simulink model "MIL4L3_SW6_V1_20220211"  (R2018b)
settings: Solver=FixedStepAuto  StartTime=0.0  StopTime=inf  FixedStep=0.001  RelTol=1e-3
PreLoadFcn:
  | A0_MILtest;
undefined symbols (not defined in the file or in its folder): Clb_ICADirect_LaneDisp_StateFive, Clb_ICADirect_LaneDisp_StateFour, Clb_ICADirect_LaneDisp_StateOne, Clb_ICADirect_LaneDisp_StateThree, Clb_ICADirect_LaneDisp_StateTwo, Clb_ICADirect_LaneDisp_StateZero, Clb_ICADirect_LaneDispSW, Clb_ICADirect_TrnLghtsCom_Switch, Clb_ICADirect_TrnLghtsCom_Value, Clb_ICADirect_TrnLghtsCrtl_Inhb, IMAP_Clb_ACU_Driver_Belt, IMAP_Clb_ACU_Driver_Belt_Over, IMAP_Clb_ACU_Passenger_Belt, IMAP_Clb_ACU_Passenger_Belt_Over, IMAP_Clb_ACU_RearLeft_Belt, IMAP_Clb_ACU_RearLeft_Belt_Over, IMAP_Clb_ACU_RearMiddle_Belt, IMAP_Clb_ACU_RearMiddle_Belt_Over, IMAP_Clb_ACU_RearRight_Belt, IMAP_Clb_ACU_RearRight_Belt_Over, IMAP_Clb_AEB_Switch, IMAP_Clb_AEB_Switch_Over, IMAP_Clb_ALC_TLC_Mode, IMAP_Clb_ALC_TLC_Mode_Over, IMAP_Clb_BCM_Battery_Voltage, IMAP_Clb_BCM_Battery_Voltage_Over, IMAP_Clb_BCM_BrakeLamp_State, IMAP_Clb_BCM_BrakeLamp_State_Over, IMAP_Clb_BCM_CHMSL_Status, IMAP_Clb_BCM_CHMSL_Status_Over, IMAP_Clb_BCM_Door_Lock_State, IMAP_Clb_BCM_Door_Lock_State_Over, IMAP_Clb_BCM_FrontWiper_State, IMAP_Clb_BCM_FrontWiper_State_Over, IMAP_Clb_BCM_FrontWiper_Switch, IMAP_Clb_BCM_FrontWiper_Switch_Over, IMAP_Clb_BCM_HazardLamp, IMAP_Clb_BCM_HazardLamp_Over, IMAP_Clb_BCM_HazardLamp_Switch, IMAP_Clb_BCM_HazardLamp_Switch_Over, IMAP_Clb_BCM_HighBeam_State, IMAP_Clb_BCM_HighBeam_State_Over, IMAP_Clb_BCM_Ignition_State, IMAP_Clb_BCM_Ignition_State_Over, IMAP_Clb_BCM_IHBC_Enabled, IMAP_Clb_BCM_IHBC_Enabled_Over, IMAP_Clb_BCM_Left_Light, IMAP_Clb_BCM_Left_Light_Over, IMAP_Clb_BCM_LeftTurn_Switch, IMAP_Clb_BCM_LeftTurn_Switch_Over, IMAP_Clb_BCM_LF_Door_State, IMAP_Clb_BCM_LF_Door_State_Over, IMAP_Clb_BCM_LowBeam_State, IMAP_Clb_BCM_LowBeam_State_Over, IMAP_Clb_BCM_LR_Door_State, IMAP_Clb_BCM_LR_Door_State_Over, IMAP_Clb_BCM_RF_Door_State, IMAP_Clb_BCM_RF_Door_State_Over, IMAP_Clb_BCM_Right_Light, IMAP_Clb_BCM_Right_Light_Over ... (+547)
libraries: CarMaker4SL x2153, simulink x292, dspstat3 x3, canmsglib x2, simulink_extras x1
(part 31 of 52)

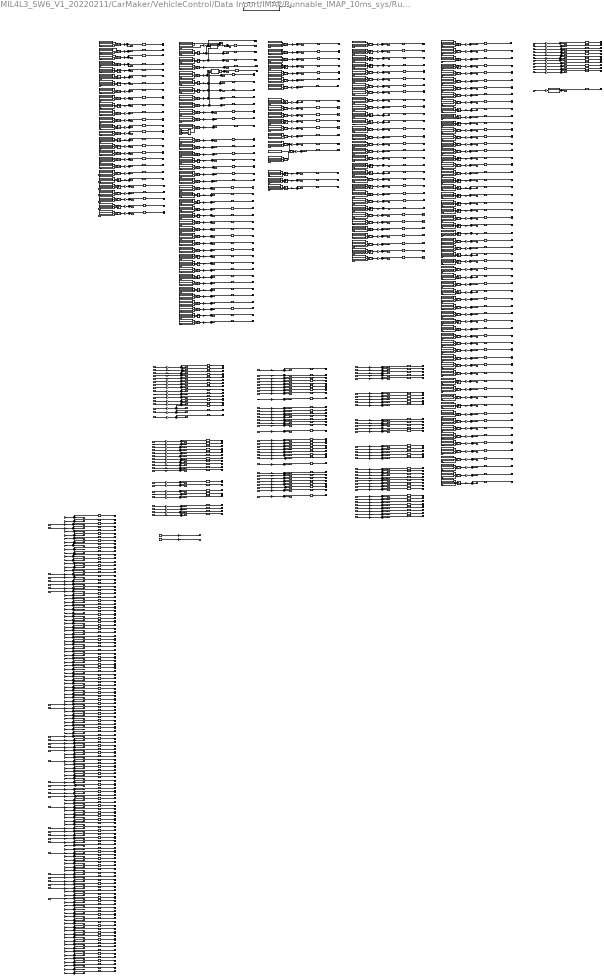
== system MIL4L3_SW6_V1_20220211/CarMaker/VehicleControl/Data Inport/IMAP/Runnable_IMAP_10ms_sys/Runnable_IMAP_10ms_sys/IMAP_Module ==
  note: SDFA_Lane_Back
  note: ORI
  note: SDFA_Sensor_Status
  note: MP5
  note: EMS
  note: SDFA_Lane
  note: SDFA_Obj
  note: BCM
  note: EPS
  note: DMS
  note: ESC
  note: 三个信号TBOX/语音/物理按键取或关系转译，转译结果0：开关关闭，1：开关开启
  SWINve_y_ABS_in_regulation : Inport
  SWINve_g_ACCEL_LONGI_CALIB : Inport  Port=2
  SWINve_y_ASR_ESP_disconnected : Inport  Port=3
  SWINve_y_ASR_in_regulation : Inport  Port=4
  SWINve_y_BCM_BrakeLampStatus : Inport  Port=5
  SWINve_y_BCM_CHMSLStatus : Inport  Port=6
  SWINve_y_BCM_State_Front_Wiper : Inport  Port=7
  SWINve_y_BCM_Status_Indicator : Inport  Port=8
  SWINve_y_Brake_secondary_contact : Inport  Port=9
  SWINve_y_Braking_effort : Inport  Port=10
  SWINve_y_Dynamic_slope : Inport  Port=11
  SWINve_y_Dynamic_slope_accuracy : Inport  Port=12
  SWINve_y_EMS_ACC_Effecitive_EMS : Inport  Port=13
  SWINve_y_EMS_ACCcontrol_Available : Inport  Port=14
  SWINve_g_EMS_Acceleration_pedal_position : Inport  Port=15
  SWINve_g_EMS_Actual_torque : Inport  Port=16
  SWINve_g_EMS_Actual_whlTrq : Inport  Port=17
  SWINve_g_EMS_Driver_request : Inport  Port=18
  SWINve_g_EMS_Driver_wheel_torque : Inport  Port=19
  SWINve_g_EMS_Engine_RPM : Inport  Port=20
  SWINve_y_EMS_Engine_state : Inport  Port=21
  SWINve_y_EMS_GearBox_ACC_Ctl_Available : Inport  Port=22
  SWINve_g_EMS_WhlTrq_max : Inport  Port=23
  SWINve_g_EMS_WhlTrq_max_offset : Inport  Port=24
  SWINve_g_EMS_WhlTrq_min : Inport  Port=25
  SWINve_g_EMS_WhlTrq_min_offset : Inport  Port=26
  SWINve_y_ESP_in_regulation : Inport  Port=27
  SWINve_y_Front_Left_pulse_malfunction : Inport  Port=28
  SWINve_y_Front_right_pulse_malfunction : Inport  Port=29
  SWINve_y_GW_BCM_SEV_main_state : Inport  Port=30
  SWINve_y_GW_EMS_ACC_Ihibited_By_Engine : Inport  Port=31
  SWINve_y_GW_EMS_EMS_Status_ACC : Inport  Port=32
  SWINve_g_GW_EMS_Pot_WhlTrq_Max : Inport  Port=33
  SWINve_g_GW_EMS_Pot_WhlTrq_Min : Inport  Port=34
  SWINve_y_GW_Mp5_ISA_Switch : Inport  Port=35
  SWINve_y_GW_Mp5_TSR_Switch : Inport  Port=36
  SWINve_y_GW_SCC_LeftSteeringWheelSwitch : Inport  Port=37
  SWINve_y_GW_SCC_RightSteeringWheelSwitch : Inport  Port=38
  SWINve_y_BCM_HazardSwitchrSt : Inport  Port=39  OutDataTypeStr=uint8  PortDimensions=1
  SWINve_y_MP5_HazardLampCtrlReq : Inport  Port=40  OutDataTypeStr=uint8  PortDimensions=1
  SWINve_y_T_box_RemoteHazardReq : Inport  Port=41  OutDataTypeStr=uint8  PortDimensions=1
  SWINve_y_High_beam_state : Inport  Port=42
  SWINve_y_IC_Fcw_Activation_Config : Inport  Port=43
  SWINve_y_IC_FCW_Sensitivity : Inport  Port=44
  SWINve_y_IC_passengerBeltSwitchSig : Inport  Port=45
  SWINve_y_IC_seat_bealt_driver_state : Inport  Port=46
  SWINve_y_Internal_SWS_status : Inport  Port=47
  SWINve_g_Lateral_acceleration : Inport  Port=48
  SWINve_y_LC_Mode : Inport  Port=49
  SWINve_y_LKA_main_switch : Inport  Port=50
  SWINve_y_Message_from_ESC_informing : Inport  Port=51
  SWINve_y_MP5_AEB_Activation_Config : Inport  Port=52
  SWINve_y_MSR_in_regulation : Inport  Port=53
  SWINve_g_No_filtered_front_left_speed : Inport  Port=54
  SWINve_g_No_filtered_front_right_speed : Inport  Port=55
  SWINve_g_No_filtered_rear_left_speed : Inport  Port=56
  SWINve_g_No_filtered_rear_rignt_speed : Inport  Port=57
  SWINve_g_number_of_kilometer : Inport  Port=58
  SWINve_y_Park_brake_function_status : Inport  Port=59
  SWINve_g_Pulse_counter_front_left_wheel : Inport  Port=60
  SWINve_g_Pulse_counter_front_right_wheel : Inport  Port=61
  SWINve_g_Pulse_counter_rearleft_wheel : Inport  Port=62
  SWINve_g_Pulse_counter_rearright_wheel : Inport  Port=63
  SWINve_y_Rear_Left_pulse_malfunction : Inport  Port=64
  SWINve_y_Rear_Right_pulse_malfunction : Inport  Port=65
  SWINve_y_Request_to_light_fault_lamp : Inport  Port=66
  SWINve_y_State_indicating_steer_or_not : Inport  Port=67
  SWINve_y_State_of_EPS_for_LKA_function : Inport  Port=68
  SWINve_g_Static_slope : Inport  Port=69
  SWINve_g_Steering_wheel_angle : Inport  Port=70
  SWINve_g_Steering_wheel_rotation_speed : Inport  Port=71
  SWINve_g_Steering_wheel_torque : Inport  Port=72
  SWINve_y_SWS_calibration : Inport  Port=73
  SWINve_y_SWS_trim : Inport  Port=74
  SWINve_y_TCU_AGB_Target_position : Inport  Port=75
  SWINve_y_TCU_ATFailure : Inport  Port=76
  SWINve_y_TCU_DCTClutchStatus : Inport  Port=77
  SWINve_y_TCU_Gear_lever_position : Inport  Port=78
  SWINve_y_TCU_GearEngagement : Inport  Port=79
  SWINve_y_TCU_PROGRAMME_ACC : Inport  Port=80
  SWINve_g_TMC_pressure : Inport  Port=81
  SWINve_y_Torque_limitation_if_DAE_limit : Inport  Port=82
  SWINve_y_Vehicle_detected_as_stationary : Inport  Port=83
  SWINve_y_Vehicle_driving_direction : Inport  Port=84
  SWINve_y_Vehicle_Hold_Status : Inport  Port=85
  SWINve_g_Vehicle_speed_of_wheelsensor : Inport  Port=86
  SWINve_y_Vehiclespd_unavailability_flag : Inport  Port=87
  SWINve_g_Yaw_speed : Inport  Port=88
  SWINve_g_YawRate_Raw : Inport  Port=89
  System_Clock : Inport  Port=90
  SDFAve_d_sensor_status : Inport  Port=91
  SDFAve_d_sen_sta_LF_radar : Inport  Port=92
  SDFAve_d_sen_sta_RF_radar : Inport  Port=93
  SDFAve_d_sen_sta_LB_radar : Inport  Port=94
  SDFAve_d_sen_sta_RB_radar : Inport  Port=95
  SDFAve_d_fusion_status : Inport  Port=96
  SDFAve_d_fusion_time_stamp : Inport  Port=97
  SDFAve_d_obj_Num : Inport  Port=98
  SDFAva_y_obj_id : Inport  Port=99
  SDFAva_g_obj_pos_x : Inport  Port=100
  SDFAva_g_obj_pos_y : Inport  Port=101
  SDFAva_g_obj_vel_x : Inport  Port=102
  SDFAva_g_obj_vel_y : Inport  Port=103
  SDFAva_g_obj_acc_x : Inport  Port=104
  SDFAva_g_obj_acc_y : Inport  Port=105
  SDFAva_g_obj_pos_var_x : Inport  Port=106
  SDFAva_g_obj_pos_var_y : Inport  Port=107
  SDFAva_g_obj_pos_var_xy : Inport  Port=108
  SDFAva_g_obj_width : Inport  Port=109
  SDFAva_g_obj_length : Inport  Port=110
  SDFAva_y_obj_class : Inport  Port=111
  SDFAva_y_obj_lane : Inport  Port=112
  SDFAva_d_obj_status : Inport  Port=113
  SDFAva_d_obj_age : Inport  Port=114
  SDFAva_y_obj_TurnLight : Inport  Port=115
  SDFAva_y_obj_BrakeLight : Inport  Port=116
  SDFAva_y_obj_MotionStatus : Inport  Port=117
  SDFAve_y_ROAD_TYPE : Inport  Port=118
  SDFAve_g_L0_C0_COEF : Inport  Port=119
  SDFAve_g_L0_C1_COEF : Inport  Port=120
  SDFAve_g_L0_C2_COEF : Inport  Port=121
  SDFAve_g_L0_C3_COEF : Inport  Port=122
  SDFAve_g_L0_VIEW_RANGE : Inport  Port=123
  SDFAve_y_L0_DETECT_QUALITY : Inport  Port=124
  SDFAve_d_L0_LINE_TYPE : Inport  Port=125
  SDFAve_g_L0_MARK_WIDTH : Inport  Port=126
  SDFAve_g_R0_C0_COEF : Inport  Port=127
  SDFAve_g_R0_C1_COEF : Inport  Port=128
  SDFAve_g_R0_C2_COEF : Inport  Port=129
  SDFAve_g_R0_C3_COEF : Inport  Port=130
  SDFAve_g_R0_VIEW_RANGE : Inport  Port=131
  SDFAve_y_R0_DETECT_QUALITY : Inport  Port=132
  SDFAve_d_R0_LINE_TYPE : Inport  Port=133
  SDFAve_g_R0_MARK_WIDTH : Inport  Port=134
  SDFAve_g_L1_C0_COEF : Inport  Port=135
  SDFAve_g_L1_C1_COEF : Inport  Port=136
  SDFAve_g_L1_C2_COEF : Inport  Port=137
  SDFAve_g_L1_C3_COEF : Inport  Port=138
  SDFAve_g_L1_VIEW_RANGE : Inport  Port=139
  SDFAve_y_L1_DETECT_QUALITY : Inport  Port=140
  SDFAve_d_L1_LINE_TYPE : Inport  Port=141
  SDFAve_g_L1_MARK_WIDTH : Inport  Port=142
  SDFAve_g_R1_C0_COEF : Inport  Port=143
  SDFAve_g_R1_C1_COEF : Inport  Port=144
  SDFAve_g_R1_C2_COEF : Inport  Port=145
  SDFAve_g_R1_C3_COEF : Inport  Port=146
  SDFAve_g_R1_VIEW_RANGE : Inport  Port=147
  SDFAve_y_R1_DETECT_QUALITY : Inport  Port=148
  SDFAve_d_R1_LINE_TYPE : Inport  Port=149
  SDFAve_g_R1_MARK_WIDTH : Inport  Port=150
  SDFAve_g_L0_C0_BACK_COEF : Inport  Port=151
  SDFAve_g_L0_C1_BACK_COEF : Inport  Port=152
  SDFAve_g_L0_C2_BACK_COEF : Inport  Port=153
  SDFAve_g_L0_C3_BACK_COEF : Inport  Port=154
  SDFAve_g_L0_BACK_RANGE : Inport  Port=155
  SDFAve_g_R0_C0_BACK_COEF : Inport  Port=156
  SDFAve_g_R0_C1_BACK_COEF : Inport  Port=157
  SDFAve_g_R0_C2_BACK_COEF : Inport  Port=158
  SDFAve_g_R0_C3_BACK_COEF : Inport  Port=159
  SDFAve_g_R0_BACK_RANGE : Inport  Port=160
  SDFAve_g_L1_C0_BACK_COEF : Inport  Port=161
  SDFAve_g_L1_C1_BACK_COEF : Inport  Port=162
  SDFAve_g_L1_C2_BACK_COEF : Inport  Port=163
  SDFAve_g_L1_C3_BACK_COEF : Inport  Port=164
  SDFAve_g_L1_BACK_RANGE : Inport  Port=165
  SDFAve_g_R1_C0_BACK_COEF : Inport  Port=166
  SDFAve_g_R1_C1_BACK_COEF : Inport  Port=167
  SDFAve_g_R1_C2_BACK_COEF : Inport  Port=168
  SDFAve_g_R1_C3_BACK_COEF : Inport  Port=169
  SDFAve_g_R1_BACK_RANGE : Inport  Port=170
  SDFAve_g_Lrg_C0_BACK_COEF : Inport  Port=171
  SDFAve_g_Lrg_C1_BACK_COEF : Inport  Port=172
  SDFAve_g_Lrg_C2_BACK_COEF : Inport  Port=173
  SDFAve_g_Lrg_C3_BACK_COEF : Inport  Port=174
  SDFAve_g_Lrg_VIEW_RANGE_start : Inport  Port=175
  SDFAve_g_Lrg_VIEW_RANGE_end : Inport  Port=176
  SDFAve_y_Lrg_DETECT_QUALITY : Inport  Port=177
  SDFAve_y_Lrg_LINE_TYPE : Inport  Port=178
  SDFAve_g_Rrg_C0_BACK_COEF : Inport  Port=179
  SDFAve_g_Rrg_C1_BACK_COEF : Inport  Port=180
  SDFAve_g_Rrg_C2_BACK_COEF : Inport  Port=181
  SDFAve_g_Rrg_C3_BACK_COEF : Inport  Port=182
  SDFAve_g_Rrg_VIEW_RANGE_start : Inport  Port=183
  SDFAve_g_Rrg_VIEW_RANGE_end : Inport  Port=184
  SDFAve_y_Rrg_DETECT_QUALITY : Inport  Port=185
  SDFAve_y_Rrg_LINE_TYPE : Inport  Port=186
  SDFAve_y_ISAValue : Inport  Port=187
  SDFAve_y_ISAPopupMessage : Inport  Port=188
  SDFAve_y_ISASignType : Inport  Port=189
  SDFAve_y_ISAStatus : Inport  Port=190
  SDFAve_y_TSR_Sign_Type : Inport  Port=191
  SDFAve_g_CameraSignalFault : Inport  Port=192
  SDFAve_y_Radar_State : Inport  Port=193
  SDFAve_y_OperatingStatus : Inport  Port=194
  SDFAve_y_Radar_FaultBitSetting_Signal : Inport  Port=195
  SWINve_y_ESC_FLWDirection : Inport  Port=196  OutDataTypeStr=uint8  PortDimensions=1
  SWINve_y_ESC_FRWDirection : Inport  Port=197  OutDataTypeStr=uint8  PortDimensions=1
  SWINve_y_ESC_TCSErrorStatus : Inport  Port=198  OutDataTypeStr=uint8  PortDimensions=1
  SWINve_y_ESC-RLWDirection : Inport  Port=199  OutDataTypeStr=uint8  PortDimensions=1
  SWINve_y_ESC_RRWDirection : Inport  Port=200  OutDataTypeStr=uint8  PortDimensions=1
  SWINve_y_ESC_EPBErrorStatus : Inport  Port=201  OutDataTypeStr=uint8  PortDimensions=1
  SWINve_y_EPS_SteeringAngle_Flag : Inport  Port=202  OutDataTypeStr=uint8  PortDimensions=1
  SWINve_g_EPS_SteeringAngle : Inport  Port=203  OutDataTypeStr=single  PortDimensions=1
  SWINve_y_EPS_DriverOverride : Inport  Port=204  OutDataTypeStr=uint8  PortDimensions=1
  SWINve_y_EPS_DriverInitializedESA : Inport  Port=205  OutDataTypeStr=uint8
  SWINve_y_EPS_ESAState : Inport  Port=206  OutDataTypeStr=uint8
  SWINve_y_ACU_RearLeftBeltSwitchSig : Inport  Port=207  OutDataTypeStr=uint8
  SWINve_y_ACU_RearMiddleBeltSwitchSig : Inport  Port=208  OutDataTypeStr=uint8
  SWINve_y_ACU_RearRightBeltSwitchSig : Inport  Port=209  OutDataTypeStr=uint8
  SWINve_y_EMS_PowertrainControlSt : Inport  Port=210  OutDataTypeStr=uint8
  SWINve_y_TCU_TCUAvailable : Inport  Port=211  OutDataTypeStr=uint8
  SWINve_y_BCM_LeftTurnSwitchSt : Inport  Port=212  OutDataTypeStr=uint8
  SWINve_y_BCM_RightTurnSwitchSt : Inport  Port=213  OutDataTypeStr=uint8
  SWINve_y_BCM_FrontWiperSwitchSt : Inport  Port=214  OutDataTypeStr=uint8
  SWINve_y_BCM_IHBC_Function_Enabled : Inport  Port=215  OutDataTypeStr=uint8
  SWINve_y_MP5_WorkSt : Inport  Port=216  OutDataTypeStr=uint8
  SWINve_y_MP5_APAModeSelect : Inport  Port=217  OutDataTypeStr=uint8
  SWINve_y_MP5_LanguageSet : Inport  Port=218  OutDataTypeStr=uint8
  SWINve_y_MP5_UPASwitch : Inport  Port=219  OutDataTypeStr=uint8
  SWINve_y_MP5_FLKActivation : Inport  Port=220  OutDataTypeStr=uint8
  SWINve_y_MP5_AutoPilotSwitch : Inport  Port=221  OutDataTypeStr=uint8
  SWINve_y_MP5_DMS_MessageType : Inport  Port=222  OutDataTypeStr=uint8
  SWINve_y_MP5_DMS_SystemEnable : Inport  Port=223  OutDataTypeStr=uint8
  SWINve_y_MP5_DMS_DeleteUserNum : Inport  Port=224  OutDataTypeStr=uint8
  SWINve_y_MP5_DMS_Sensity : Inport  Port=225  OutDataTypeStr=uint8
  SWINve_y_MP5_DMS_EyeFatigueMonitor : Inport  Port=226  OutDataTypeStr=uint8
  SWINve_y_MP5_DMS_LongtimeDriveMonitor : Inport  Port=227  OutDataTypeStr=uint8
  SWINve_y_MP5_DMS_SideViewMonitor : Inport  Port=228  OutDataTypeStr=uint8
  SWINve_y_MP5_DMS_UsingPhoneMonitor : Inport  Port=229  OutDataTypeStr=uint8
  SWINve_y_MP5_DMS_SmokingMonitor : Inport  Port=230  OutDataTypeStr=uint8
  SWINve_y_MP5_DMS_DrinkWaterMonitor : Inport  Port=231  OutDataTypeStr=uint8
  SWINve_y_MP5_DMS_UserAccount : Inport  Port=232  OutDataTypeStr=uint8
  SWINve_y_Mp5_ISAMode : Inport  Port=233  OutDataTypeStr=uint8  PortDimensions=1
  SWINve_y_Mp5_LDWWarningMode : Inport  Port=234  OutDataTypeStr=uint8  PortDimensions=1
  SWINve_y_MP5_ADASSpeedLimit : Inport  Port=235  OutDataTypeStr=uint8  PortDimensions=1
  SWINve_y_MP5_TLCModeSelection : Inport  Port=236  OutDataTypeStr=uint8  PortDimensions=1
  SWINve_y_MP5_ESASwitch : Inport  Port=237  OutDataTypeStr=uint8  PortDimensions=1
  SWINve_y_Mp5_ELKSwitch : Inport  Port=238  OutDataTypeStr=uint8
  SWINve_y_PEPS_RKECommand : Inport  Port=239  OutDataTypeStr=uint8  PortDimensions=1
  SWINve_y_MP5_BSD_LCW_Activation : Inport  Port=240  OutDataTypeStr=uint8  PortDimensions=1
  SWINve_y_MP5_FCTAActivation : Inport  Port=241  OutDataTypeStr=uint8  PortDimensions=1
  SWINve_y_MP5_RCTAActivation : Inport  Port=242  OutDataTypeStr=uint8  PortDimensions=1
  SWINve_y_MP5_DOWActivation : Inport  Port=243  OutDataTypeStr=uint8
  SWINve_y_MP5_JA_Modes : Inport  Port=244  OutDataTypeStr=uint8
  SWINve_y_MP5_JA_Alert_Switch : Inport  Port=245  OutDataTypeStr=uint8
  SWINve_y_ESC_BLRequest : Inport  Port=246  OutDataTypeStr=uint8  PortDimensions=1
  SWINve_y_PEPS_DoorLockReq : Inport  Port=247  OutDataTypeStr=uint8  PortDimensions=1
  SWINve_y_BCM_DoorLockSt : Inport  Port=248  OutDataTypeStr=uint8  PortDimensions=1
  SWINve_y_BCM_LowBeamStatus : Inport  Port=249  OutDataTypeStr=uint8  PortDimensions=1
  SWINve_g_BCM_BattVolt : Inport  Port=250  OutDataTypeStr=single  PortDimensions=1
  SWINve_d_TBOX_LocalTimeYear : Inport  Port=251  OutDataTypeStr=uint16  PortDimensions=1
  SWINve_y_TBOX_LocalTimeMonth : Inport  Port=252  OutDataTypeStr=uint8  PortDimensions=1
  SWINve_y_TBOX_LocalTimeDate : Inport  Port=253  OutDataTypeStr=uint8  PortDimensions=1
  SWINve_y_TBOX_LocalTimeHour : Inport  Port=254  OutDataTypeStr=uint8  PortDimensions=1
  SWINve_y_TBOX_LocalTimeMinute : Inport  Port=255  OutDataTypeStr=uint8
  SWINve_y_TBOX_LocalTimeSecond : Inport  Port=256  OutDataTypeStr=uint8
  SWINve_y_TBOX_LocalTimeValid : Inport  Port=257  OutDataTypeStr=uint8
  SWINve_g_AC_AmbTemp : Inport  Port=258  OutDataTypeStr=single
  SWINve_y_EPS_SteeringTorqueSensorSt : Inport  Port=259  OutDataTypeStr=uint8  PortDimensions=1
  SWINve_g_EPS_LKACurrentOverlay : Inport  Port=260  OutDataTypeStr=single  PortDimensions=1
  SWINve_y_EPS_WarningLampSt : Inport  Port=261  OutDataTypeStr=uint8  PortDimensions=1
  SWINve_g_EPS_ElectPowerConsumption : Inport  Port=262  OutDataTypeStr=single  PortDimensions=1
  SWINve_g_EMS_EngActualIndTorque : Inport  Port=263  OutDataTypeStr=single  PortDimensions=1
  SWINve_y_EMS_AccPedalFaultBit : Inport  Port=264  OutDataTypeStr=uint8  PortDimensions=1
  SWINve_y_TCU_PRNDLStatus : Inport  Port=265  OutDataTypeStr=uint8  PortDimensions=1
  SWINve_y_TCU_ShiftLeverPosValidFlag : Inport  Port=266  OutDataTypeStr=uint8  PortDimensions=1
  SWINve_y_ESC_LateralAccelarationValidity : Inport  Port=267  OutDataTypeStr=uint8  PortDimensions=1
  SWINve_y_ESC_YawrateValidity : Inport  Port=268  OutDataTypeStr=uint8
  SWINve_y_ESC_LongitudinalAccelerationValidity : Inport  Port=269  OutDataTypeStr=uint8
  SWINve_y_ESC_ABSValidity : Inport  Port=270  OutDataTypeStr=uint8
  SWINve_y_ESC_ABSAlarmSig : Inport  Port=271  OutDataTypeStr=uint8
  SWINve_y_ESC_FLWHeelSpdFaultSignal : Inport  Port=272  OutDataTypeStr=uint8
  SWINve_y_ESC_FRWHeelSpdFaultSignal : Inport  Port=273  OutDataTypeStr=uint8
  SWINve_y_ESC_RLWHeelSpdFaultSignal : Inport  Port=274  OutDataTypeStr=uint8
  SWINve_y_ESC_RRWHeelSpdFaultSignal : Inport  Port=275  OutDataTypeStr=uint8
  SWINve_y_ESC_AEBAvailable : Inport  Port=276  OutDataTypeStr=uint8
  SWINve_y_ESC_AEBActive : Inport  Port=277  OutDataTypeStr=uint8
  SWINve_y_ESC_ACCAvailable : Inport  Port=278  OutDataTypeStr=uint8
  SWINve_y_ESC_ACCActive : Inport  Port=279  OutDataTypeStr=uint8
  SWINve_y_ESC_EPBDisplayMessageReq : Inport  Port=280  OutDataTypeStr=uint8
  SWINve_y_ESC_EPBWarningIndicationReq : Inport  Port=281  OutDataTypeStr=uint8
  SWINve_y_ESC_EPBSwitchStatics : Inport  Port=282  OutDataTypeStr=uint8
  SWINve_y_ESC_EPBSwitchStaticsValidity : Inport  Port=283  OutDataTypeStr=uint8
  SWINve_y_ESC_EBDAlarmSig : Inport  Port=284  OutDataTypeStr=uint8
  SWINve_y_ESC_AVHStatus : Inport  Port=285  OutDataTypeStr=uint8
  SWINve_y_BCM_LeftlightSt : Inport  Port=286  OutDataTypeStr=uint8  PortDimensions=1
  SWINve_y_BCM_RightlightSt : Inport  Port=287  OutDataTypeStr=uint8  PortDimensions=1
  SWINve_y_BCM_TrunkSt : Inport  Port=288  OutDataTypeStr=uint8  PortDimensions=1
  SWINve_y_BCM_LFDoorSwitchSt : Inport  Port=289  OutDataTypeStr=uint8  PortDimensions=1
  SWINve_y_BCM_RFDoorSwitchSt : Inport  Port=290  OutDataTypeStr=uint8  PortDimensions=1
  SWINve_y_BCM_RRDoorSwitchSt : Inport  Port=291  OutDataTypeStr=uint8  PortDimensions=1
  SWINve_y_BCM_LRDoorSwitchSt : Inport  Port=292  OutDataTypeStr=uint8  PortDimensions=1
  SWINve_g_ESC_BrakeWheelCylinderPressure : Inport  Port=293  OutDataTypeStr=single  PortDimensions=1
  FAPAve_Cnt_AdvancedParkingAssist : Inport  Port=294
  SDFAve_d_ORI_CIPV_ID : Inport  Port=295
  SDFAve_d_ORI_Obj_Num : Inport  Port=296
  SDFAva_g_ORI_Obj_AbsAx : Inport  Port=297  PortDimensions=20
  SDFAva_g_ORI_Obj_AbsAy : Inport  Port=298  PortDimensions=20
  SDFAva_g_ORI_Obj_RelVel : Inport  Port=299  PortDimensions=20
  SDFAva_g_ORI_Obj_RelVely : Inport  Port=300  PortDimensions=20
  SDFAva_g_ORI_Obj_LongDis : Inport  Port=301  PortDimensions=20
  SDFAva_g_ORI_Obj_LateralDis : Inport  Port=302  PortDimensions=20
  SDFAva_d_ORI_Obj_Class : Inport  Port=303  PortDimensions=20
  SDFAva_d_ORI_Obj_ID : Inport  Port=304  PortDimensions=20
  SDFAve_g_ORI_L0_C3 : Inport  Port=305
  SDFAve_g_ORI_L0_C2 : Inport  Port=306
  SDFAve_g_ORI_L0_C1 : Inport  Port=307
  SDFAve_g_ORI_L0_C0 : Inport  Port=308
  SDFAve_d_ORI_L0_Type : Inport  Port=309
  SDFAve_g_ORI_L0_VR : Inport  Port=310
  SDFAve_g_ORI_L1_C3 : Inport  Port=311
  SDFAve_g_ORI_L1_C2 : Inport  Port=312
  SDFAve_g_ORI_L1_C1 : Inport  Port=313
  SDFAve_g_ORI_L1_C0 : Inport  Port=314
  SDFAve_d_ORI_L1_Type : Inport  Port=315
  SDFAve_g_ORI_L1_VR : Inport  Port=316
  SDFAve_g_ORI_R0_C3 : Inport  Port=317
  SDFAve_g_ORI_R0_C2 : Inport  Port=318
  SDFAve_g_ORI_R0_C1 : Inport  Port=319
  SDFAve_g_ORI_R0_C0 : Inport  Port=320
  SDFAve_d_ORI_R0_LT : Inport  Port=321
  SDFAve_g_ORI_R0_VR : Inport  Port=322
  SDFAve_g_ORI_R1_C3 : Inport  Port=323
  SDFAve_g_ORI_R1_C2 : Inport  Port=324
  SDFAve_g_ORI_R1_C1 : Inport  Port=325
  SDFAve_g_ORI_R1_C0 : Inport  Port=326
  SDFAve_d_ORI_R1_LT : Inport  Port=327
  SDFAve_g_ORI_R1_VR : Inport  Port=328
  AND : Logic  Operator=OR  Inputs=3  AllPortsSameDT=off  OutDataTypeStr=boolean
  Constant : Constant  Value=IMAP_Clb_LKA_Main_Switch  OutDataTypeStr=uint16
  Constant1 : Constant  Value=IMAP_Clb_LKA_Main_Switch_Over  OutDataTypeStr=boolean
  Constant10 : Constant  Value=IMAP_Clb_ISA_Switch  OutDataTypeStr=uint16
  Constant100 : Constant  Value=IMAP_Clb_TBOX_LocalTimeM  OutDataTypeStr=uint16
  Constant101 : Constant  Value=IMAP_Clb_TBOX_LocalTimeM_Over  OutDataTypeStr=boolean
  Constant102 : Constant  Value=IMAP_Clb_TBOX_LocalTimeD  OutDataTypeStr=uint16
  Constant103 : Constant  Value=IMAP_Clb_TBOX_LocalTimeD_Over  OutDataTypeStr=boolean
  Constant104 : Constant  Value=IMAP_Clb_TBOX_LocalTimeH  OutDataTypeStr=uint16
  Constant105 : Constant  Value=IMAP_Clb_TBOX_LocalTimeH_Over  OutDataTypeStr=boolean
  Constant106 : Constant  Value=IMAP_Clb_TBOX_LocalTimeMin  OutDataTypeStr=uint16
  Constant107 : Constant  Value=IMAP_Clb_TBOX_LocalTimeMin_Over  OutDataTypeStr=boolean
  Constant108 : Constant  Value=IMAP_Clb_TBOX_LocalTimeS  OutDataTypeStr=uint16
  Constant109 : Constant  Value=IMAP_Clb_TBOX_LocalTimeS_Over  OutDataTypeStr=boolean
  Constant11 : Constant  Value=IMAP_Clb_ISA_Switch_Over  OutDataTypeStr=boolean
  Constant110 : Constant  Value=IMAP_Clb_TBOX_LocalTime_Valid  OutDataTypeStr=uint16
  Constant111 : Constant  Value=IMAP_Clb_TBOX_LocalTime_Valid_Over  OutDataTypeStr=boolean
  Constant112 : Constant  Value=IMAP_Clb_Time_System_Clock  OutDataTypeStr=uint16
  Constant113 : Constant  Value=IMAP_Clb_Time_System_Clock_Over  OutDataTypeStr=boolean
  Constant114 : Constant  Value=IMAP_Clb_GW_IC_Odometer  OutDataTypeStr=uint32
  Constant115 : Constant  Value=IMAP_Clb_GW_IC_Odometer_Over  OutDataTypeStr=boolean
  Constant116 : Constant  Value=IMAP_Clb_Outside_Temp  OutDataTypeStr=uint16
  Constant117 : Constant  Value=IMAP_Clb_Outside_Temp_Over  OutDataTypeStr=boolean
  Constant118 : Constant  Value=IMAP_Clb_ACU_RearLeft_Belt  OutDataTypeStr=uint16
  Constant119 : Constant  Value=IMAP_Clb_ACU_RearLeft_Belt_Over  OutDataTypeStr=boolean
  Constant12 : Constant  Value=IMAP_Clb_TSR_Switch  OutDataTypeStr=uint16
  Constant120 : Constant  Value=IMAP_Clb_ACU_RearMiddle_Belt  OutDataTypeStr=uint16
  Constant121 : Constant  Value=IMAP_Clb_ACU_RearMiddle_Belt_Over  OutDataTypeStr=boolean
  Constant122 : Constant  Value=IMAP_Clb_ACU_RearRight_Belt  OutDataTypeStr=uint16
  Constant123 : Constant  Value=IMAP_Clb_ACU_RearRight_Belt_Over  OutDataTypeStr=boolean
  Constant124 : Constant  Value=IMAP_Clb_BCM_LeftTurn_Switch  OutDataTypeStr=uint16
  Constant125 : Constant  Value=IMAP_Clb_BCM_LeftTurn_Switch_Over  OutDataTypeStr=boolean
  Constant126 : Constant  Value=IMAP_Clb_BCM_RightTurn_Switch  OutDataTypeStr=uint16
  Constant127 : Constant  Value=IMAP_Clb_BCM_RightTurn_Switch_Over  OutDataTypeStr=boolean
  Constant128 : Constant  Value=IMAP_Clb_BCM_FrontWiper_Switch  OutDataTypeStr=uint16
  Constant129 : Constant  Value=IMAP_Clb_BCM_FrontWiper_Switch_Over  OutDataTypeStr=boolean
  Constant13 : Constant  Value=IMAP_Clb_TSR_Switch_Over  OutDataTypeStr=boolean
  Constant130 : Constant  Value=IMAP_Clb_BCM_IHBC_Enabled  OutDataTypeStr=uint16
  Constant131 : Constant  Value=IMAP_Clb_BCM_IHBC_Enabled_Over  OutDataTypeStr=boolean
  Constant132 : Constant  Value=IMAP_Clb_EPS_LKA_State  OutDataTypeStr=uint16
  Constant133 : Constant  Value=IMAP_Clb_EPS_LKA_State_Over  OutDataTypeStr=boolean
  Constant134 : Constant  Value=IMAP_Clb_EPS_SW_Trq  OutDataTypeStr=single
  Constant135 : Constant  Value=IMAP_Clb_EPS_SW_Trq_Over  OutDataTypeStr=boolean
  Constant136 : Constant  Value=IMAP_Clb_EPS_Trq_State  OutDataTypeStr=uint16
  Constant137 : Constant  Value=IMAP_Clb_EPS_Trq_State_Over  OutDataTypeStr=boolean
  Constant138 : Constant  Value=IMAP_Clb_SAS_Clb_State  OutDataTypeStr=uint16
  Constant139 : Constant  Value=IMAP_Clb_SAS_Clb_State_Over  OutDataTypeStr=boolean
  Constant14 : Constant  Value=IMAP_Clb_ISA_ISLC_Mode  OutDataTypeStr=uint16
  Constant140 : Constant  Value=IMAP_Clb_SAS_Trim_State  OutDataTypeStr=uint16
  Constant141 : Constant  Value=IMAP_Clb_SAS_Trim_State_Over  OutDataTypeStr=boolean
  Constant142 : Constant  Value=IMAP_Clb_EPS_TrqLim_State  OutDataTypeStr=uint16
  Constant143 : Constant  Value=IMAP_Clb_EPS_TrqLim_State_Over  OutDataTypeStr=boolean
  Constant144 : Constant  Value=IMAP_Clb_EPS_LKA_Current  OutDataTypeStr=single
  Constant145 : Constant  Value=IMAP_Clb_EPS_LKA_Current_Over  OutDataTypeStr=boolean
  Constant146 : Constant  Value=IMAP_Clb_SW_Angle  OutDataTypeStr=single
  Constant147 : Constant  Value=IMAP_Clb_SW_Angle_Over  OutDataTypeStr=boolean
  Constant148 : Constant  Value=IMAP_Clb_SW_Angle_Speed  OutDataTypeStr=single
  Constant149 : Constant  Value=IMAP_Clb_SW_Angle_Speed_Over  OutDataTypeStr=boolean
  Constant15 : Constant  Value=IMAP_Clb_ISA_ISLC_Mode_Over  OutDataTypeStr=boolean
  Constant150 : Constant  Value=IMAP_Clb_SWS_Failure_Status  OutDataTypeStr=uint16
  Constant151 : Constant  Value=IMAP_Clb_SWS_Failure_Status_Over  OutDataTypeStr=boolean
  Constant152 : Constant  Value=IMAP_Clb_EPS_Steer_Hold_State  OutDataTypeStr=uint16
  Constant153 : Constant  Value=IMAP_Clb_EPS_Steer_Hold_State_Over  OutDataTypeStr=boolean
  Constant154 : Constant  Value=IMAP_Clb_EPS_Warning_State  OutDataTypeStr=uint16
  Constant155 : Constant  Value=IMAP_Clb_EPS_Warning_State_Over  OutDataTypeStr=boolean
  Constant156 : Constant  Value=IMAP_Clb_EPS_PowerCon  OutDataTypeStr=single
  Constant157 : Constant  Value=IMAP_Clb_EPS_PowerCon_Over  OutDataTypeStr=boolean
  Constant158 : Constant  Value=IMAP_Clb_EPS_SteeringAngle_Flag  OutDataTypeStr=uint16
  Constant159 : Constant  Value=IMAP_Clb_EPS_SteeringAngle_Flag_Over  OutDataTypeStr=boolean
  Constant16 : Constant  Value=IMAP_Clb_LDW_Warn_Mode  OutDataTypeStr=uint16
  Constant160 : Constant  Value=IMAP_Clb_EPS_SteeringAngle  OutDataTypeStr=single
  Constant161 : Constant  Value=IMAP_Clb_EPS_SteeringAngle_Over  OutDataTypeStr=boolean
  Constant162 : Constant  Value=IMAP_Clb_EPS_Driver_Override  OutDataTypeStr=uint16
  Constant163 : Constant  Value=IMAP_Clb_EPS_Driver_Override_Over  OutDataTypeStr=boolean
  Constant164 : Constant  Value=IMAP_Clb_EPS_Driver_Active_ESA  OutDataTypeStr=uint16
  Constant165 : Constant  Value=IMAP_Clb_EPS_Driver_Active_ESA_Over  OutDataTypeStr=boolean
  Constant166 : Constant  Value=IMAP_Clb_EPS_ESA_State  OutDataTypeStr=uint16
  Constant167 : Constant  Value=IMAP_Clb_EPS_ESA_State_Over  OutDataTypeStr=boolean
  Constant168 : Constant  Value=IMAP_Clb_EMS_ACC_Status  OutDataTypeStr=uint16
  Constant169 : Constant  Value=IMAP_Clb_EMS_ACC_Status_Over  OutDataTypeStr=boolean
  Constant17 : Constant  Value=IMAP_Clb_LDW_Warn_Mode_Over  OutDataTypeStr=boolean
  Constant170 : Constant  Value=IMAP_Clb_EMS_Pot_WhlT_Max  OutDataTypeStr=single
  Constant171 : Constant  Value=IMAP_Clb_EMS_Pot_WhlT_Max_Over  OutDataTypeStr=boolean
  Constant172 : Constant  Value=IMAP_Clb_EMS_Pot_WhlT_Min  OutDataTypeStr=single
  Constant173 : Constant  Value=IMAP_Clb_EMS_Pot_WhlT_Min_Over  OutDataTypeStr=boolean
  Constant174 : Constant  Value=IMAP_Clb_EMS_RealPedal  OutDataTypeStr=single
  Constant175 : Constant  Value=IMAP_Clb_EMS_RealPedal_Over  OutDataTypeStr=boolean
  Constant176 : Constant  Value=IMAP_Clb_EMS_MaxTWhl  OutDataTypeStr=single
  Constant177 : Constant  Value=IMAP_Clb_EMS_MaxTWhl_Over  OutDataTypeStr=boolean
  Constant178 : Constant  Value=IMAP_Clb_EMS_MaxTWhl_Offset  OutDataTypeStr=single
  Constant179 : Constant  Value=IMAP_Clb_EMS_MaxTWhl_Offset_Over  OutDataTypeStr=boolean
  Constant18 : Constant  Value=0  OutDataTypeStr=uint32  SampleTime=-1
  Constant180 : Constant  Value=IMAP_Clb_EMS_MinTWhl  OutDataTypeStr=single
  Constant181 : Constant  Value=IMAP_Clb_EMS_MinTWhl_Over  OutDataTypeStr=boolean
  Constant182 : Constant  Value=IMAP_Clb_EMS_MinTWhl_Offset  OutDataTypeStr=single
  Constant183 : Constant  Value=IMAP_Clb_EMS_MinTWhl_Offset_Over  OutDataTypeStr=boolean
  Constant184 : Constant  Value=IMAP_Clb_EMS_Actual_FlwT  OutDataTypeStr=single
  Constant185 : Constant  Value=IMAP_Clb_EMS_Actual_FlwT_Over  OutDataTypeStr=boolean
  Constant186 : Constant  Value=IMAP_Clb_EMS_Actual_IndT  OutDataTypeStr=single
  Constant187 : Constant  Value=IMAP_Clb_EMS_Actual_IndT_Over  OutDataTypeStr=boolean
  Constant188 : Constant  Value=IMAP_Clb_EMS_Realize_TWhl  OutDataTypeStr=single
  Constant189 : Constant  Value=IMAP_Clb_EMS_Realize_TWhl_Over  OutDataTypeStr=boolean
  Constant19 : Constant  Value=0  OutDataTypeStr=uint32  SampleTime=-1
  Constant190 : Constant  Value=IMAP_Clb_EMS_ACC_VirtualPedal  OutDataTypeStr=single
  Constant191 : Constant  Value=IMAP_Clb_EMS_ACC_VirtualPedal_Over  OutDataTypeStr=boolean
  Constant192 : Constant  Value=IMAP_Clb_EMS_AccPedal_Fault  OutDataTypeStr=uint16
  Constant193 : Constant  Value=IMAP_Clb_EMS_AccPedal_Fault_Over  OutDataTypeStr=boolean
  Constant194 : Constant  Value=IMAP_Clb_EMS_Driver_Torque  OutDataTypeStr=single
  Constant195 : Constant  Value=IMAP_Clb_EMS_Driver_Torque_Over  OutDataTypeStr=boolean
  Constant196 : Constant  Value=IMAP_Clb_EMS_Engine_Speed  OutDataTypeStr=single
  Constant197 : Constant  Value=IMAP_Clb_EMS_Engine_Speed_Over  OutDataTypeStr=boolean
  Constant198 : Constant  Value=IMAP_Clb_TCU_Actual_Gear  OutDataTypeStr=uint16
  Constant199 : Constant  Value=IMAP_Clb_TCU_Actual_Gear_Over  OutDataTypeStr=boolean
  Constant2 : Constant  Value=IMAP_Clb_LKA_Mode  OutDataTypeStr=uint16
  Constant20 : Constant  Value=IMAP_Clb_Speed_Limit  OutDataTypeStr=uint16
  Constant200 : Constant  Value=IMAP_Clb_TCU_Target_Gear  OutDataTypeStr=uint16
  Constant201 : Constant  Value=IMAP_Clb_TCU_Target_Gear_Over  OutDataTypeStr=boolean
  Constant202 : Constant  Value=IMAP_Clb_TCU_PRND_State  OutDataTypeStr=uint16
  Constant203 : Constant  Value=IMAP_Clb_TCU_PRND_State_Over  OutDataTypeStr=boolean
  Constant204 : Constant  Value=IMAP_Clb_TCU_AT_Failure  OutDataTypeStr=uint16
  Constant205 : Constant  Value=IMAP_Clb_TCU_AT_Failure_Over  OutDataTypeStr=boolean
  Constant206 : Constant  Value=IMAP_Clb_TCU_Shift_Valid  OutDataTypeStr=uint16
  Constant207 : Constant  Value=IMAP_Clb_TCU_Shift_Valid_Over  OutDataTypeStr=boolean
  Constant208 : Constant  Value=IMAP_Clb_TCU_DCT_Clutch_State  OutDataTypeStr=uint16
  Constant209 : Constant  Value=IMAP_Clb_TCU_DCT_Clutch_State_Over  OutDataTypeStr=boolean
  Constant21 : Constant  Value=IMAP_Clb_Speed_Limit_Over  OutDataTypeStr=boolean
  Constant210 : Constant  Value=IMAP_Clb_TCU_Gear_Engage  OutDataTypeStr=uint16
  Constant211 : Constant  Value=IMAP_Clb_TCU_Gear_Engage_Over  OutDataTypeStr=boolean
  Constant212 : Constant  Value=IMAP_Clb_TCU_Select_ATMode  OutDataTypeStr=uint16
  Constant213 : Constant  Value=IMAP_Clb_TCU_Select_ATMode_Over  OutDataTypeStr=boolean
  Constant214 : Constant  Value=IMAP_Clb_EMS_Engine_Status  OutDataTypeStr=uint16
  Constant215 : Constant  Value=IMAP_Clb_EMS_Engine_Status_Over  OutDataTypeStr=boolean
  Constant216 : Constant  Value=IMAP_Clb_EMS_Gearbox_CtlAvail  OutDataTypeStr=uint16
  Constant217 : Constant  Value=IMAP_Clb_EMS_Gearbox_CtlAvail_Over  OutDataTypeStr=boolean
  Constant218 : Constant  Value=IMAP_Clb_EMS_ACC_Effective  OutDataTypeStr=uint16
  Constant219 : Constant  Value=IMAP_Clb_EMS_ACC_Effective_Over  OutDataTypeStr=boolean
  Constant22 : Constant  Value=IMAP_Clb_ALC_TLC_Mode  OutDataTypeStr=uint16
  Constant220 : Constant  Value=IMAP_Clb_EMS_ACC_CtlAvail  OutDataTypeStr=uint16
  Constant221 : Constant  Value=IMAP_Clb_EMS_ACC_CtlAvail_Over  OutDataTypeStr=boolean
  Constant222 : Constant  Value=IMAP_Clb_EMS_ACC_Inhibited  OutDataTypeStr=uint16
  Constant223 : Constant  Value=IMAP_Clb_EMS_ACC_Inhibited_Over  OutDataTypeStr=boolean
  Constant224 : Constant  Value=IMAP_Clb_EMS_Brake_Pedal  OutDataTypeStr=uint16
  Constant225 : Constant  Value=IMAP_Clb_EMS_Brake_Pedal_Over  OutDataTypeStr=boolean
  Constant226 : Constant  Value=IMAP_Clb_EMS_PowertrainCtl_State  OutDataTypeStr=uint16
  Constant227 : Constant  Value=IMAP_Clb_EMS_PowertrainCtl_State_Over  OutDataTypeStr=boolean
  Constant228 : Constant  Value=IMAP_Clb_TCU_TCU_Available  OutDataTypeStr=uint16
  Constant229 : Constant  Value=IMAP_Clb_TCU_TCU_Available_Over  OutDataTypeStr=boolean
  Constant23 : Constant  Value=IMAP_Clb_ALC_TLC_Mode_Over  OutDataTypeStr=boolean
  Constant230 : Constant  Value=IMAP_Clb_ESC_LatAcc  OutDataTypeStr=single
  Constant231 : Constant  Value=IMAP_Clb_ESC_LatAcc_Over  OutDataTypeStr=boolean
  Constant232 : Constant  Value=IMAP_Clb_ESC_LatAcc_Valid  OutDataTypeStr=uint16
  Constant233 : Constant  Value=IMAP_Clb_ESC_LatAcc_Valid_Over  OutDataTypeStr=boolean
  Constant234 : Constant  Value=IMAP_Clb_ESC_YawRate  OutDataTypeStr=single
  Constant235 : Constant  Value=IMAP_Clb_ESC_YawRate_Over  OutDataTypeStr=boolean
  Constant236 : Constant  Value=IMAP_Clb_ESC_YawRate_Valid  OutDataTypeStr=uint16
  Constant237 : Constant  Value=IMAP_Clb_ESC_YawRate_Valid_Over  OutDataTypeStr=boolean
  Constant238 : Constant  Value=IMAP_Clb_ESC_UnYawRate  OutDataTypeStr=single
  Constant239 : Constant  Value=IMAP_Clb_ESC_UnYawRate_Over  OutDataTypeStr=boolean
  Constant24 : Constant  Value=IMAP_Clb_ESA_Switch  OutDataTypeStr=uint16
  Constant240 : Constant  Value=IMAP_Clb_ESC_VehSpd  OutDataTypeStr=single
  Constant241 : Constant  Value=IMAP_Clb_ESC_VehSpd_Over  OutDataTypeStr=boolean
  Constant242 : Constant  Value=IMAP_Clb_ESC_LonAcc  OutDataTypeStr=single
  Constant243 : Constant  Value=IMAP_Clb_ESC_LonAcc_Over  OutDataTypeStr=boolean
  Constant244 : Constant  Value=IMAP_Clb_ESC_LonAcc_Valid  OutDataTypeStr=uint16
  Constant245 : Constant  Value=IMAP_Clb_ESC_LonAcc_Valid_Over  OutDataTypeStr=boolean
  Constant246 : Constant  Value=IMAP_Clb_ESC_Brake_Press  OutDataTypeStr=single
  Constant247 : Constant  Value=IMAP_Clb_ESC_Brake_Press_Over  OutDataTypeStr=boolean
  Constant248 : Constant  Value=IMAP_Clb_ESC_Static_Slope  OutDataTypeStr=single
  Constant249 : Constant  Value=IMAP_Clb_ESC_Static_Slope_Over  OutDataTypeStr=boolean
  Constant25 : Constant  Value=IMAP_Clb_ESA_Switch_Over  OutDataTypeStr=boolean
  Constant250 : Constant  Value=IMAP_Clb_ESC_DySlope_Accuracy  OutDataTypeStr=single
  Constant251 : Constant  Value=IMAP_Clb_ESC_DySlope_Accuracy_Over  OutDataTypeStr=boolean
  Constant252 : Constant  Value=IMAP_Clb_ESC_DySlope  OutDataTypeStr=single
  Constant253 : Constant  Value=IMAP_Clb_ESC_DySlope_Over  OutDataTypeStr=boolean
  Constant254 : Constant  Value=IMAP_Clb_ESC_Brake_Effort  OutDataTypeStr=uint16
  Constant255 : Constant  Value=IMAP_Clb_ESC_Brake_Effort_Over  OutDataTypeStr=boolean
  Constant256 : Constant  Value=IMAP_Clb_ESC_Veh_Standstill  OutDataTypeStr=uint16
  Constant257 : Constant  Value=IMAP_Clb_ESC_Veh_Standstill_Over  OutDataTypeStr=boolean
  Constant258 : Constant  Value=IMAP_Clb_ESC_OFF  OutDataTypeStr=uint16
  Constant259 : Constant  Value=IMAP_Clb_ESC_OFF_Over  OutDataTypeStr=boolean
  Constant26 : Constant  Value=IMAP_Clb_ELK_Switch  OutDataTypeStr=uint16
  Constant260 : Constant  Value=IMAP_Clb_ESC_AlarmSig  OutDataTypeStr=uint16
  Constant261 : Constant  Value=IMAP_Clb_ESC_AlarmSig_Over  OutDataTypeStr=boolean
  Constant262 : Constant  Value=IMAP_Clb_ESC_ESC_Active  OutDataTypeStr=uint16
  Constant263 : Constant  Value=IMAP_Clb_ESC_ESC_Active_Over  OutDataTypeStr=boolean
  Constant264 : Constant  Value=IMAP_Clb_ESC_MSR_Active  OutDataTypeStr=uint16
  Constant265 : Constant  Value=IMAP_Clb_ESC_MSR_Active_Over  OutDataTypeStr=boolean
  Constant266 : Constant  Value=IMAP_Clb_ESC_TCS_Active  OutDataTypeStr=uint16
  Constant267 : Constant  Value=IMAP_Clb_ESC_TCS_Active_Over  OutDataTypeStr=boolean
  Constant268 : Constant  Value=IMAP_Clb_ESC_VehSpd_Valid  OutDataTypeStr=uint16
  Constant269 : Constant  Value=IMAP_Clb_ESC_VehSpd_Valid_Over  OutDataTypeStr=boolean
  Constant27 : Constant  Value=IMAP_Clb_ELK_Switch_Over  OutDataTypeStr=boolean
  Constant270 : Constant  Value=IMAP_Clb_ESC_ABS_Active  OutDataTypeStr=uint16
  Constant271 : Constant  Value=IMAP_Clb_ESC_ABS_Active_Over  OutDataTypeStr=boolean
  Constant272 : Constant  Value=IMAP_Clb_ESC_ABS_Valid  OutDataTypeStr=uint16
  Constant273 : Constant  Value=IMAP_Clb_ESC_ABS_Valid_Over  OutDataTypeStr=boolean
  Constant274 : Constant  Value=IMAP_Clb_ESC_ABS_AlarmSig  OutDataTypeStr=uint16
  Constant275 : Constant  Value=IMAP_Clb_ESC_ABS_AlarmSig_Over  OutDataTypeStr=boolean
  Constant276 : Constant  Value=IMAP_Clb_ESC_FL_WheelPulVal  OutDataTypeStr=uint16
  Constant277 : Constant  Value=IMAP_Clb_ESC_FL_WheelPulVal_Over  OutDataTypeStr=boolean
  Constant278 : Constant  Value=IMAP_Clb_ESC_FR_WheelPulVal  OutDataTypeStr=uint16
  Constant279 : Constant  Value=IMAP_Clb_ESC_FR_WheelPulVal_Over  OutDataTypeStr=boolean
  Constant28 : Constant  Value=IMAP_Clb_PEPS_RKE_Command  OutDataTypeStr=uint16
  Constant280 : Constant  Value=IMAP_Clb_ESC_RL_WheelPulVal  OutDataTypeStr=uint16
  Constant281 : Constant  Value=IMAP_Clb_ESC_RL_WheelPulVal_Over  OutDataTypeStr=boolean
  Constant282 : Constant  Value=IMAP_Clb_ESC_RR_WheelPulVal  OutDataTypeStr=uint16
  Constant283 : Constant  Value=IMAP_Clb_ESC_RR_WheelPulVal_Over  OutDataTypeStr=boolean
  Constant284 : Constant  Value=IMAP_Clb_ESC_FL_WhlSpd  OutDataTypeStr=single
  Constant285 : Constant  Value=IMAP_Clb_ESC_FL_WhlSpd_Over  OutDataTypeStr=boolean
  Constant286 : Constant  Value=IMAP_Clb_ESC_FL_WhlSpd_Fault  OutDataTypeStr=uint16
  Constant287 : Constant  Value=IMAP_Clb_ESC_FL_WhlSpd_Fault_Over  OutDataTypeStr=boolean
  Constant288 : Constant  Value=IMAP_Clb_ESC_FR_WhlSpd  OutDataTypeStr=single
  Constant289 : Constant  Value=IMAP_Clb_ESC_FR_WhlSpd_Over  OutDataTypeStr=boolean
  Constant29 : Constant  Value=IMAP_Clb_PEPS_RKE_Command_Over  OutDataTypeStr=boolean
  Constant290 : Constant  Value=IMAP_Clb_ESC_FR_WhlSpd_Fault  OutDataTypeStr=uint16
  Constant291 : Constant  Value=IMAP_Clb_ESC_FR_WhlSpd_Fault_Over  OutDataTypeStr=boolean
  Constant292 : Constant  Value=IMAP_Clb_ESC_RL_WhlSpd  OutDataTypeStr=single
  Constant293 : Constant  Value=IMAP_Clb_ESC_RL_WhlSpd_Over  OutDataTypeStr=boolean
  Constant294 : Constant  Value=IMAP_Clb_ESC_RL_WhlSpd_Fault  OutDataTypeStr=uint16
  Constant295 : Constant  Value=IMAP_Clb_ESC_RL_WhlSpd_Fault_Over  OutDataTypeStr=boolean
  Constant296 : Constant  Value=IMAP_Clb_ESC_RR_WhlSpd  OutDataTypeStr=single
  Constant297 : Constant  Value=IMAP_Clb_ESC_RR_WhlSpd_Over  OutDataTypeStr=boolean
  Constant298 : Constant  Value=IMAP_Clb_ESC_RR_WhlSpd_Fault  OutDataTypeStr=uint16
  Constant299 : Constant  Value=IMAP_Clb_ESC_RR_WhlSpd_Fault_Over  OutDataTypeStr=boolean
  Constant3 : Constant  Value=IMAP_Clb_LKA_Mode_Over  OutDataTypeStr=boolean
  Constant30 : Constant  Value=IMAP_Clb_BSD_LCW_Switch  OutDataTypeStr=uint16
  Constant300 : Constant  Value=IMAP_Clb_ESC_FL_Wheel_Pulse  OutDataTypeStr=uint16
  Constant301 : Constant  Value=IMAP_Clb_ESC_FL_Wheel_Pulse_Over  OutDataTypeStr=boolean
  Constant302 : Constant  Value=IMAP_Clb_ESC_FR_Wheel_Pulse  OutDataTypeStr=uint16
  Constant303 : Constant  Value=IMAP_Clb_ESC_FR_Wheel_Pulse_Over  OutDataTypeStr=boolean
  Constant304 : Constant  Value=IMAP_Clb_ESC_RL_Wheel_Pulse  OutDataTypeStr=uint16
  Constant305 : Constant  Value=IMAP_Clb_ESC_RL_Wheel_Pulse_Over  OutDataTypeStr=boolean
  Constant306 : Constant  Value=IMAP_Clb_ESC_RR_Wheel_Pulse  OutDataTypeStr=uint16
  Constant307 : Constant  Value=IMAP_Clb_ESC_RR_Wheel_Pulse_Over  OutDataTypeStr=boolean
  Constant308 : Constant  Value=IMAP_Clb_ESC_Brake_Failsafe  OutDataTypeStr=uint16
  Constant309 : Constant  Value=IMAP_Clb_ESC_Brake_Failsafe_Over  OutDataTypeStr=boolean
  Constant31 : Constant  Value=IMAP_Clb_BSD_LCW_Switch_Over  OutDataTypeStr=boolean
  Constant310 : Constant  Value=IMAP_Clb_ESC_AEB_Available  OutDataTypeStr=uint16
  Constant311 : Constant  Value=IMAP_Clb_ESC_AEB_Available_Over  OutDataTypeStr=boolean
  Constant312 : Constant  Value=IMAP_Clb_ESC_AEB_Active  OutDataTypeStr=uint16
  Constant313 : Constant  Value=IMAP_Clb_ESC_AEB_Active_Over  OutDataTypeStr=boolean
  Constant314 : Constant  Value=IMAP_Clb_ESC_ACC_Available  OutDataTypeStr=uint16
  Constant315 : Constant  Value=IMAP_Clb_ESC_ACC_Available_Over  OutDataTypeStr=boolean
  Constant316 : Constant  Value=IMAP_Clb_ESC_ACC_Active  OutDataTypeStr=uint16
  Constant317 : Constant  Value=IMAP_Clb_ESC_ACC_Active_Over  OutDataTypeStr=boolean
  Constant318 : Constant  Value=IMAP_Clb_EPB_Status  OutDataTypeStr=uint16
  Constant319 : Constant  Value=IMAP_Clb_EPB_Status_Over  OutDataTypeStr=boolean
  Constant32 : Constant  Value=IMAP_Clb_FCTA_Switch  OutDataTypeStr=uint16
  Constant320 : Constant  Value=IMAP_Clb_EPB_Display_Req  OutDataTypeStr=uint16
  Constant321 : Constant  Value=IMAP_Clb_EPB_Display_Req_Over  OutDataTypeStr=boolean
  Constant322 : Constant  Value=IMAP_Clb_EPB_Warn_Req  OutDataTypeStr=uint16
  Constant323 : Constant  Value=IMAP_Clb_EPB_Warn_Req_Over  OutDataTypeStr=boolean
  Constant324 : Constant  Value=IMAP_Clb_EPB_Switch_State  OutDataTypeStr=uint16
  Constant325 : Constant  Value=IMAP_Clb_EPB_Switch_State_Over  OutDataTypeStr=boolean
  Constant326 : Constant  Value=IMAP_Clb_EPB_Switch_Valid  OutDataTypeStr=uint16
  Constant327 : Constant  Value=IMAP_Clb_EPB_Switch_Valid_Over  OutDataTypeStr=boolean
  Constant328 : Constant  Value=IMAP_Clb_ESC_Drive_Direction  OutDataTypeStr=uint16
  Constant329 : Constant  Value=IMAP_Clb_ESC_Drive_Direction_Over  OutDataTypeStr=boolean
  Constant33 : Constant  Value=IMAP_Clb_FCTA_Switch_Over  OutDataTypeStr=boolean
  Constant330 : Constant  Value=IMAP_Clb_ESC_Hold_State  OutDataTypeStr=uint16
  Constant331 : Constant  Value=IMAP_Clb_ESC_Hold_State_Over  OutDataTypeStr=boolean
  Constant332 : Constant  Value=IMAP_Clb_ESC_EBD_AlarmSig  OutDataTypeStr=uint16
  Constant333 : Constant  Value=IMAP_Clb_ESC_EBD_AlarmSig_Over  OutDataTypeStr=boolean
  Constant334 : Constant  Value=IMAP_Clb_ESC_AVH_Status  OutDataTypeStr=uint16
  Constant335 : Constant  Value=IMAP_Clb_ESC_AVH_Status_Over  OutDataTypeStr=boolean
  Constant336 : Constant  Value=IMAP_Clb_ESC_FLW_Direction  OutDataTypeStr=uint16
  Constant337 : Constant  Value=IMAP_Clb_ESC_FLW_Direction_Over  OutDataTypeStr=boolean
  Constant338 : Constant  Value=IMAP_Clb_ESC_FRW_Direction  OutDataTypeStr=uint16
  Constant339 : Constant  Value=IMAP_Clb_ESC_FRW_Direction_Over  OutDataTypeStr=boolean
  Constant34 : Constant  Value=IMAP_Clb_RCTA_Swtich  OutDataTypeStr=uint16
  Constant340 : Constant  Value=IMAP_Clb_ESC_TCS_ErrorStatus  OutDataTypeStr=uint16
  Constant341 : Constant  Value=IMAP_Clb_ESC_TCS_ErrorStatus_Over  OutDataTypeStr=boolean
  Constant342 : Constant  Value=IMAP_Clb_ESC_RLW_Direction  OutDataTypeStr=uint16
  Constant343 : Constant  Value=IMAP_Clb_ESC_RLW_Direction_Over  OutDataTypeStr=boolean
  Constant344 : Constant  Value=IMAP_Clb_ESC_RRW_Direction  OutDataTypeStr=uint16
  Constant345 : Constant  Value=IMAP_Clb_ESC_RRW_Direction_Over  OutDataTypeStr=boolean
  Constant346 : Constant  Value=IMAP_Clb_ESC_EPB_ErrorStatus  OutDataTypeStr=uint16
  Constant347 : Constant  Value=IMAP_Clb_ESC_EPB_ErrorStatus_Over  OutDataTypeStr=boolean
  Constant348 : Constant  Value=IMAP_Clb_ESC_BrkWhlCylinder_Pressure  OutDataTypeStr=single
  Constant349 : Constant  Value=IMAP_Clb_ESC_BrkWhlCylinder_Pressure_Over  OutDataTypeStr=boolean
  Constant35 : Constant  Value=IMAP_Clb_RCTA_Swtich_Over  OutDataTypeStr=boolean
  Constant351 : Constant  Value=IMAP_Clb_BCM_HazardLamp_Switch  OutDataTypeStr=uint16
  Constant352 : Constant  Value=IMAP_Clb_BCM_HazardLamp_Switch_Over  OutDataTypeStr=boolean
  Constant354 : Constant  Value=IMAP_Clb_SAS_Or_EPS_SW_Angle_Over  OutDataTypeStr=boolean
  Constant36 : Constant  Value=IMAP_Clb_DOW_Switch  OutDataTypeStr=uint16
  Constant37 : Constant  Value=IMAP_Clb_DOW_Switch_Over  OutDataTypeStr=boolean
  Constant38 : Constant  Value=IMAP_Clb_JA_Brake_Switch  OutDataTypeStr=uint16
  Constant39 : Constant  Value=IMAP_Clb_JA_Brake_Switch_Over  OutDataTypeStr=boolean
  Constant4 : Constant  Value=IMAP_Clb_AEB_Switch  OutDataTypeStr=uint16
  Constant40 : Constant  Value=IMAP_Clb_JA_Alert_Switch  OutDataTypeStr=uint16
  Constant41 : Constant  Value=IMAP_Clb_JA_Alert_Switch_Over  OutDataTypeStr=boolean
  Constant42 : Constant  Value=IMAP_Clb_MP5_Work_State  OutDataTypeStr=uint16
  Constant43 : Constant  Value=IMAP_Clb_MP5_Work_State_Over  OutDataTypeStr=boolean
  Constant44 : Constant  Value=IMAP_Clb_MP5_APA_ModeSelect  OutDataTypeStr=uint16
  Constant45 : Constant  Value=IMAP_Clb_MP5_APA_ModeSelect_Over  OutDataTypeStr=boolean
  Constant46 : Constant  Value=IMAP_Clb_MP5_LanguageSet  OutDataTypeStr=uint16
  Constant47 : Constant  Value=IMAP_Clb_MP5_LanguageSet_Over  OutDataTypeStr=boolean
  Constant48 : Constant  Value=IMAP_Clb_MP5_UPA_Switch  OutDataTypeStr=uint16
  Constant49 : Constant  Value=IMAP_Clb_MP5_UPA_Switch_Over  OutDataTypeStr=boolean
  Constant5 : Constant  Value=IMAP_Clb_AEB_Switch_Over  OutDataTypeStr=boolean
  Constant50 : Constant  Value=IMAP_Clb_MP5_FLK_Activation  OutDataTypeStr=uint16
  Constant51 : Constant  Value=IMAP_Clb_MP5_FLK_Activation_Over  OutDataTypeStr=boolean
  Constant52 : Constant  Value=IMAP_Clb_MP5_AutoPilot_Switch  OutDataTypeStr=uint16
  Constant53 : Constant  Value=IMAP_Clb_MP5_AutoPilot_Switch_Over  OutDataTypeStr=boolean
  Constant54 : Constant  Value=IMAP_Clb_BCM_HazardLamp  OutDataTypeStr=uint16
  Constant55 : Constant  Value=IMAP_Clb_BCM_HazardLamp_Over  OutDataTypeStr=boolean
  Constant56 : Constant  Value=IMAP_Clb_BCM_Left_Light  OutDataTypeStr=uint16
  Constant57 : Constant  Value=IMAP_Clb_BCM_Left_Light_Over  OutDataTypeStr=boolean
  Constant58 : Constant  Value=IMAP_Clb_BCM_Right_Light  OutDataTypeStr=uint16
  Constant59 : Constant  Value=IMAP_Clb_BCM_Right_Light_Over  OutDataTypeStr=boolean
  Constant6 : Constant  Value=IMAP_Clb_FCW_Switch  OutDataTypeStr=uint16
  Constant60 : Constant  Value=IMAP_Clb_ESC_BrakeLamp_Req  OutDataTypeStr=uint16
  Constant61 : Constant  Value=IMAP_Clb_ESC_BrakeLamp_Req_Over  OutDataTypeStr=boolean
  Constant62 : Constant  Value=IMAP_Clb_BCM_Trunk_State  OutDataTypeStr=uint16
  Constant63 : Constant  Value=IMAP_Clb_BCM_Trunk_State_Over  OutDataTypeStr=boolean
  Constant64 : Constant  Value=IMAP_Clb_BCM_LF_Door_State  OutDataTypeStr=uint16
  Constant65 : Constant  Value=IMAP_Clb_BCM_LF_Door_State_Over  OutDataTypeStr=boolean
  Constant66 : Constant  Value=IMAP_Clb_BCM_RF_Door_State  OutDataTypeStr=uint16
  Constant67 : Constant  Value=IMAP_Clb_BCM_RF_Door_State_Over  OutDataTypeStr=boolean
  Constant68 : Constant  Value=IMAP_Clb_BCM_RR_Door_State  OutDataTypeStr=uint16
  Constant69 : Constant  Value=IMAP_Clb_BCM_RR_Door_State_Over  OutDataTypeStr=boolean
  Constant7 : Constant  Value=IMAP_Clb_FCW_Switch_Over  OutDataTypeStr=boolean
  Constant70 : Constant  Value=IMAP_Clb_BCM_LR_Door_State  OutDataTypeStr=uint16
  Constant71 : Constant  Value=IMAP_Clb_BCM_LR_Door_State_Over  OutDataTypeStr=boolean
  Constant72 : Constant  Value=IMAP_Clb_SCC_Left_SwitchSig  OutDataTypeStr=uint16
  Constant73 : Constant  Value=IMAP_Clb_SCC_Left_SwitchSig_Over  OutDataTypeStr=boolean
  Constant74 : Constant  Value=IMAP_Clb_SCC_Right_SwitchSig  OutDataTypeStr=uint16
  Constant75 : Constant  Value=IMAP_Clb_SCC_Right_SwitchSig_Over  OutDataTypeStr=boolean
  Constant76 : Constant  Value=IMAP_Clb_PEPS_Door_Lock_Req  OutDataTypeStr=uint16
  Constant77 : Constant  Value=IMAP_Clb_PEPS_Door_Lock_Req_Over  OutDataTypeStr=boolean
  Constant78 : Constant  Value=IMAP_Clb_BCM_Door_Lock_State  OutDataTypeStr=uint16
  Constant79 : Constant  Value=IMAP_Clb_BCM_Door_Lock_State_Over  OutDataTypeStr=boolean
  Constant8 : Constant  Value=IMAP_Clb_FCW_Sensitivity  OutDataTypeStr=uint16
  Constant80 : Constant  Value=IMAP_Clb_BCM_Ignition_State  OutDataTypeStr=uint16
  Constant81 : Constant  Value=IMAP_Clb_BCM_Ignition_State_Over  OutDataTypeStr=boolean
  Constant82 : Constant  Value=IMAP_Clb_ACU_Driver_Belt  OutDataTypeStr=uint16
  Constant83 : Constant  Value=IMAP_Clb_ACU_Driver_Belt_Over  OutDataTypeStr=boolean
  Constant84 : Constant  Value=IMAP_Clb_BCM_FrontWiper_State  OutDataTypeStr=uint16
  Constant85 : Constant  Value=IMAP_Clb_BCM_FrontWiper_State_Over  OutDataTypeStr=boolean
  Constant86 : Constant  Value=IMAP_Clb_BCM_CHMSL_Status  OutDataTypeStr=uint16
  Constant87 : Constant  Value=IMAP_Clb_BCM_CHMSL_Status_Over  OutDataTypeStr=boolean
  Constant88 : Constant  Value=IMAP_Clb_BCM_BrakeLamp_State  OutDataTypeStr=uint16
  Constant89 : Constant  Value=IMAP_Clb_BCM_BrakeLamp_State_Over  OutDataTypeStr=boolean
  Constant9 : Constant  Value=IMAP_Clb_FCW_Sensitivity_Over  OutDataTypeStr=boolean
  Constant90 : Constant  Value=IMAP_Clb_ACU_Passenger_Belt  OutDataTypeStr=uint16
  Constant91 : Constant  Value=IMAP_Clb_ACU_Passenger_Belt_Over  OutDataTypeStr=boolean
  Constant92 : Constant  Value=IMAP_Clb_BCM_LowBeam_State  OutDataTypeStr=uint16
  Constant93 : Constant  Value=IMAP_Clb_BCM_LowBeam_State_Over  OutDataTypeStr=boolean
  Constant94 : Constant  Value=IMAP_Clb_BCM_HighBeam_State  OutDataTypeStr=uint16
  Constant95 : Constant  Value=IMAP_Clb_BCM_HighBeam_State_Over  OutDataTypeStr=boolean
  Constant96 : Constant  Value=IMAP_Clb_BCM_Battery_Voltage  OutDataTypeStr=single
  Constant97 : Constant  Value=IMAP_Clb_BCM_Battery_Voltage_Over  OutDataTypeStr=boolean
  Constant98 : Constant  Value=IMAP_Clb_TBOX_LocalTimeY  OutDataTypeStr=uint16
  Constant99 : Constant  Value=IMAP_Clb_TBOX_LocalTimeY_Over  OutDataTypeStr=boolean
  Data Type Conversion : DataTypeConversion  OutDataTypeStr=uint16
  Data Type Conversion{1..7,9..71,73..116,118..131,134..140,142,144..145,147..150,154..157,159..160,162,164..167,169..170,172,174..177,179..180,182,184..187,189..190,192..234,236,238..244,246,249..255,257,260..266,268,271..277,279,282..286,291..295,300..304,309..313,318..328,330..347,349..350,353..354,360..371,374..387,389..401,403..488} (423 alike) : DataTypeConversion
  Data Type Conversion8 : DataTypeConversion  OutDataTypeStr=uint16
  Gain{,288,354..357,359,364..369,380..381,384,386..387,390,392,396..397,400..403,405..406,408..416,421..427,432..434} (47 alike) : Gain  OutDataTypeStr=single  SaturateOnIntegerOverflow=on  ParamDataTypeStr=Inherit: Same as input
  Gain{1..5,8,12,15..16,27..29,37,39..58,63..94,96..99,102..103,105,108..109,128,130..132,138,155,162..163,169..170,176..177,183..189,192..194,196,201..212,215..218,228..236,241,249,255,273,279..280,282,286..287,289..318,320..328,330,333..353,373..374,378..379,385,391,443,445,448..452} (205 alike) : Gain  OutDataTypeStr=uint16
  Gain{6..7,9..11,13..14,17..26,30..36,38,59..62,95,101,104,106..107,110..127,129,134..137,140,143..147,150..154,157..161,165..168,172,174..175,179,190..191,198..200,213..214,219..227,238..239,242,244,246..247,250,252,254,256,258,260,262,264,266..267,270..271,274,277..278,281,283..285,319,329,331..332,375..377,442,444} (131 alike) : Gain  OutDataTypeStr=single
  Gain100 : Gain  OutDataTypeStr=uint32
  Gain{237,261,265,269} (4 alike) : Gain  Gain=0.5  OutDataTypeStr=single
  Gain{358,361..363,371..372,382..383,388..389,393..395,398,404,407,417..420,428..431,435..441} (31 alike) : Gain  OutDataTypeStr=uint16  SaturateOnIntegerOverflow=on  ParamDataTypeStr=Inherit: Same as input
  Gain360 : Gain  Gain=0.5  OutDataTypeStr=single  SaturateOnIntegerOverflow=on  ParamDataTypeStr=Inherit: Same as input
  Gain370 : Gain  Gain=0.5  OutDataTypeStr=single  SaturateOnIntegerOverflow=on  ParamDataTypeStr=Inherit: Same as input
  Gain399 : Gain  SaturateOnIntegerOverflow=on  OutDataTypeStr=Inherit: Same as input  ParamDataTypeStr=Inherit: Same as input
  Gain446 : Gain  OutDataTypeStr=uint32
  Gain447 : Gain  OutDataTypeStr=uint32
  MATLAB Function : MATLAB Function  TreatAsAtomicUnit=on
  Switch{,1..175} (176 alike) : Switch  Criteria=u2 > Threshold
  Terminator{1..143,145..148,150..151,153,155..158,160..161,163,165..168,170..171,173,175..178,180..181,183..225,227,229..235,237,240..246,248,251..257,259,262..268,270,273..277,282..286,291..295,300..304,309..319,321..353,356..383,385..471} (425 alike) : Terminator
  Version : Constant  Value=1126  OutDataTypeStr=uint16
  array_transfer10 : MATLAB Function  TreatAsAtomicUnit=on
  array_transfer11 : MATLAB Function  TreatAsAtomicUnit=on
  IMAPve_d_LKA_Main_Switch : Outport
  IMAPve_d_LKA_Mode : Outport  Port=2
  IMAPve_d_AEB_Switch : Outport  Port=3
  IMAPve_d_FCW_Switch : Outport  Port=4
  IMAPve_d_FCW_Sensitivity : Outport  Port=5
  IMAPve_d_ISA_Switch : Outport  Port=6
  IMAPve_d_TSR_Switch : Outport  Port=7
  IMAPve_d_ISA_ISLC_Mode : Outport  Port=8
  IMAPve_d_LDW_Warn_Mode : Outport  Port=9
  IMAPve_d_Speed_Limit : Outport  Port=10
  IMAPve_d_ALC_TLC_Mode : Outport  Port=11
  IMAPve_d_ESA_Switch : Outport  Port=12
  IMAPve_d_ELK_Switch : Outport  Port=13
  IMAPve_d_PEPS_RKE_Command : Outport  Port=14
  IMAPve_d_BSD_LCW_Switch : Outport  Port=15
  IMAPve_d_FCTA_Switch : Outport  Port=16
  IMAPve_d_RCTA_Swtich : Outport  Port=17
  IMAPve_d_DOW_Switch : Outport  Port=18
  IMAPve_d_JA_Brake_Switch : Outport  Port=19
  IMAPve_d_JA_Alert_Switch : Outport  Port=20
  IMAPve_d_EPS_LKA_State : Outport  Port=21
  IMAPve_g_EPS_SW_Trq : Outport  Port=22
  IMAPve_d_EPS_Trq_State : Outport  Port=23
  IMAPve_d_SAS_Clb_State : Outport  Port=24
  IMAPve_d_SAS_Trim_State : Outport  Port=25
  IMAPve_d_EPS_TrqLim_State : Outport  Port=26
  IMAPve_g_EPS_LKA_Current : Outport  Port=27
  IMAPve_g_ESC_LatAcc : Outport  Port=28
  IMAPve_d_ESC_LatAcc_Valid : Outport  Port=29
  IMAPve_g_ESC_YawRate : Outport  Port=30
  IMAPve_d_ESC_YawRate_Valid : Outport  Port=31
  IMAPve_g_ESC_UnYawRate : Outport  Port=32
  IMAPve_g_ESC_VehSpd : Outport  Port=33
  IMAPve_g_ESC_LonAcc : Outport  Port=34
  IMAPve_d_ESC_LonAcc_Valid : Outport  Port=35
  IMAPve_g_ESC_Brake_Press : Outport  Port=36
  IMAPve_g_ESC_Static_Slope : Outport  Port=37
  IMAPve_g_ESC_DySlope_Accuracy : Outport  Port=38
  IMAPve_g_ESC_DySlope : Outport  Port=39
  IMAPve_g_SW_Angle : Outport  Port=40
  IMAPve_g_SW_Angle_Speed : Outport  Port=41
  IMAPve_d_BCM_HazardLamp : Outport  Port=42
  IMAPve_d_BCM_Left_Light : Outport  Port=43
  IMAPve_d_BCM_Right_Light : Outport  Port=44
  IMAPve_d_ESC_BrakeLamp_Req : Outport  Port=45
  IMAPve_d_BCM_Opening_State : Outport  Port=46
  IMAPve_d_BCM_Trunk_State : Outport  Port=47
  IMAPve_d_BCM_LF_Door_State : Outport  Port=48
  IMAPve_d_BCM_RF_Door_State : Outport  Port=49
  IMAPve_d_BCM_RR_Door_State : Outport  Port=50
  IMAPve_d_BCM_LR_Door_State : Outport  Port=51
  IMAPve_d_SCC_Left_SwitchSig : Outport  Port=52
  IMAPve_d_SCC_Right_SwitchSig : Outport  Port=53
  IMAPve_d_BCM_HazardLamp_Switch : Outport  Port=54
  IMAPve_d_PEPS_Door_Lock_Req : Outport  Port=55
  IMAPve_d_BCM_Door_Lock_State : Outport  Port=56
  IMAPve_d_EMS_ACC_Status : Outport  Port=57
  IMAPve_g_EMS_Pot_WhlT_Max : Outport  Port=58
  IMAPve_g_EMS_Pot_WhlT_Min : Outport  Port=59
  IMAPve_g_EMS_RealPedal : Outport  Port=60
  IMAPve_g_EMS_MaxTWhl : Outport  Port=61
  IMAPve_g_EMS_MaxTWhl_Offset : Outport  Port=62
  IMAPve_g_EMS_MinTWhl : Outport  Port=63
  IMAPve_g_EMS_MinTWhl_Offset : Outport  Port=64
  IMAPve_g_EMS_Actual_FlwT : Outport  Port=65
  IMAPve_g_EMS_Actual_IndT : Outport  Port=66
  IMAPve_g_EMS_Realize_TWhl : Outport  Port=67
  IMAPve_g_EMS_ACC_VirtualPedal : Outport  Port=68
  IMAPve_d_EMS_AccPedal_Fault : Outport  Port=69
  IMAPve_g_EMS_Driver_Torque : Outport  Port=70
  IMAPve_d_ESC_Brake_Effort : Outport  Port=71
  IMAPve_g_EMS_Engine_Speed : Outport  Port=72
  IMAPve_d_ESC_Veh_Standstill : Outport  Port=73
  IMAPve_d_TCU_Actual_Gear : Outport  Port=74
  IMAPve_d_TCU_Target_Gear : Outport  Port=75
  IMAPve_d_TCU_PRND_State : Outport  Port=76
  IMAPve_d_BCM_Ignition_State : Outport  Port=77
  IMAPve_d_ACU_Driver_Belt : Outport  Port=78
  IMAPve_d_SWS_Failure_Status : Outport  Port=79
  IMAPve_d_ESC_OFF : Outport  Port=80
  IMAPve_d_ESC_AlarmSig : Outport  Port=81
  IMAPve_d_ESC_ESC_Active : Outport  Port=82
  IMAPve_d_ESC_MSR_Active : Outport  Port=83
  IMAPve_d_ESC_TCS_Active : Outport  Port=84
  IMAPve_d_ESC_VehSpd_Valid : Outport  Port=85
  IMAPve_d_ESC_ABS_Active : Outport  Port=86
  IMAPve_d_ESC_ABS_Valid : Outport  Port=87
  IMAPve_d_ESC_ABS_AlarmSig : Outport  Port=88
  IMAPve_d_ESC_FL_WheelPulVal : Outport  Port=89
  IMAPve_d_ESC_FR_WheelPulVal : Outport  Port=90
  IMAPve_d_ESC_RL_WheelPulVal : Outport  Port=91
  IMAPve_d_ESC_RR_WheelPulVal : Outport  Port=92
  IMAPve_g_ESC_FL_WhlSpd : Outport  Port=93
  IMAPve_d_ESC_FL_WhlSpd_Fault : Outport  Port=94
  IMAPve_g_ESC_FR_WhlSpd : Outport  Port=95
  IMAPve_d_ESC_FR_WhlSpd_Fault : Outport  Port=96
  IMAPve_g_ESC_RL_WhlSpd : Outport  Port=97
  IMAPve_d_ESC_RL_WhlSpd_Fault : Outport  Port=98
  IMAPve_g_ESC_RR_WhlSpd : Outport  Port=99
  IMAPve_d_ESC_RR_WhlSpd_Fault : Outport  Port=100
  IMAPve_d_ESC_FL_Wheel_Pulse : Outport  Port=101
  IMAPve_d_ESC_FR_Wheel_Pulse : Outport  Port=102
  IMAPve_d_ESC_RL_Wheel_Pulse : Outport  Port=103
  IMAPve_d_ESC_RR_Wheel_Pulse : Outport  Port=104
  IMAPve_d_TCU_AT_Failure : Outport  Port=105
  IMAPve_d_TCU_Shift_Valid : Outport  Port=106
  IMAPve_d_TCU_DCT_Clutch_State : Outport  Port=107
  IMAPve_d_TCU_Gear_Engage : Outport  Port=108
  IMAPve_d_TCU_Select_ATMode : Outport  Port=109
  IMAPve_d_EMS_Engine_Status : Outport  Port=110
  IMAPve_d_EMS_Gearbox_CtlAvail : Outport  Port=111
  IMAPve_d_ESC_Brake_Failsafe : Outport  Port=112
  IMAPve_d_ESC_AEB_Available : Outport  Port=113
  IMAPve_d_ESC_AEB_Active : Outport  Port=114
  IMAPve_d_ESC_ACC_Available : Outport  Port=115
  IMAPve_d_ESC_ACC_Active : Outport  Port=116
  IMAPve_d_EMS_ACC_Effective : Outport  Port=117
  IMAPve_d_BCM_FrontWiper_State : Outport  Port=118
  IMAPve_d_BCM_CHMSL_Status : Outport  Port=119
  IMAPve_d_BCM_BrakeLamp_State : Outport  Port=120
  IMAPve_d_ACU_Passenger_Belt : Outport  Port=121
  IMAPve_d_EMS_ACC_CtlAvail : Outport  Port=122
  IMAPve_d_EMS_ACC_Inhibited : Outport  Port=123
  IMAPve_d_EMS_Brake_Pedal : Outport  Port=124
  IMAPve_d_BCM_LowBeam_State : Outport  Port=125
  IMAPve_d_BCM_HighBeam_State : Outport  Port=126
  IMAPve_d_EPB_Status : Outport  Port=127
  IMAPve_d_EPB_Display_Req : Outport  Port=128
  IMAPve_d_EPB_Warn_Req : Outport  Port=129
  IMAPve_d_EPB_Switch_State : Outport  Port=130
  IMAPve_d_EPB_Switch_Valid : Outport  Port=131
  IMAPve_d_ESC_Drive_Direction : Outport  Port=132
  IMAPve_d_ESC_Hold_State : Outport  Port=133
  IMAPve_d_EPS_Steer_Hold_State : Outport  Port=134
  IMAPve_d_EPS_Warning_State : Outport  Port=135
  IMAPve_g_EPS_PowerCon : Outport  Port=136
  IMAPve_d_ESC_EBD_AlarmSig : Outport  Port=137
  IMAPve_d_ESC_AVH_Status : Outport  Port=138
  IMAPve_g_BCM_Battery_Voltage : Outport  Port=139
  IMAPve_d_TBOX_LocalTimeY : Outport  Port=140
  IMAPve_d_TBOX_LocalTimeM : Outport  Port=141
  IMAPve_d_TBOX_LocalTimeD : Outport  Port=142
  IMAPve_d_TBOX_LocalTimeH : Outport  Port=143
  IMAPve_d_TBOX_LocalTimeMin : Outport  Port=144
  IMAPve_d_TBOX_LocalTimeS : Outport  Port=145
  IMAPve_d_TBOX_LocalTime_Valid : Outport  Port=146
  IMAPve_d_Radar_State : Outport  Port=147
  IMAPve_d_Time_System_Clock : Outport  Port=148
  IMAPve_g_GW_IC_Odometer : Outport  Port=149
  IMAPve_d_Outside_Temp : Outport  Port=150
  IMAPve_d_ORI_CIPV_ID : Outport  Port=151  OutDataTypeStr=uint16
  IMAPve_d_ORI_Obj_Num : Outport  Port=152  OutDataTypeStr=uint16
  IMAPva_d_ORI_Obj_Class : Outport  Port=153  OutDataTypeStr=uint16  PortDimensions=20
  IMAPva_g_ORI_Obj_RelVel : Outport  Port=154  OutDataTypeStr=single  PortDimensions=20
  IMAPva_g_ORI_Obj_LongDis : Outport  Port=155  OutDataTypeStr=single  PortDimensions=20
  IMAPva_g_ORI_Obj_LAngle : Outport  Port=156  OutDataTypeStr=single  PortDimensions=20
  IMAPva_g_ORI_Obj_RAngle : Outport  Port=157  OutDataTypeStr=single  PortDimensions=20
  IMAPva_g_ORI_Obj_Width : Outport  Port=158  OutDataTypeStr=single  PortDimensions=20
  IMAPva_d_ORI_Obj_ID : Outport  Port=159  OutDataTypeStr=uint16  PortDimensions=20
  IMAPve_g_ORI_L0_C3 : Outport  Port=160  OutDataTypeStr=single
  IMAPve_g_ORI_L0_C2 : Outport  Port=161  OutDataTypeStr=single
  IMAPve_g_ORI_L0_C1 : Outport  Port=162  OutDataTypeStr=single
  IMAPve_g_ORI_L0_C0 : Outport  Port=163  OutDataTypeStr=single
  IMAPve_d_ORI_L0_Type : Outport  Port=164  OutDataTypeStr=uint16
  IMAPve_g_ORI_L0_VR : Outport  Port=165  OutDataTypeStr=single
  IMAPve_g_ORI_L0_W : Outport  Port=166  OutDataTypeStr=single
  IMAPve_g_ORI_L1_C3 : Outport  Port=167  OutDataTypeStr=single
  IMAPve_g_ORI_L1_C2 : Outport  Port=168  OutDataTypeStr=single
  IMAPve_g_ORI_L1_C1 : Outport  Port=169  OutDataTypeStr=single
  IMAPve_g_ORI_L1_C0 : Outport  Port=170  OutDataTypeStr=single
  IMAPve_d_ORI_L1_Type : Outport  Port=171  OutDataTypeStr=uint16
  IMAPve_g_ORI_L1_VR : Outport  Port=172  OutDataTypeStr=single
  IMAPve_g_ORI_L1_W : Outport  Port=173  OutDataTypeStr=single
  IMAPve_g_ORI_R0_C3 : Outport  Port=174  OutDataTypeStr=single
  IMAPve_g_ORI_R0_C2 : Outport  Port=175  OutDataTypeStr=single
  IMAPve_g_ORI_R0_C1 : Outport  Port=176  OutDataTypeStr=single
  IMAPve_g_ORI_R0_C0 : Outport  Port=177  OutDataTypeStr=single
  IMAPve_d_ORI_R0_LT : Outport  Port=178  OutDataTypeStr=uint16
  IMAPve_g_ORI_R0_VR : Outport  Port=179  OutDataTypeStr=single
  IMAPve_g_ORI_R0_W : Outport  Port=180  OutDataTypeStr=single
  IMAPve_g_ORI_R1_C3 : Outport  Port=181  OutDataTypeStr=single
  IMAPve_g_ORI_R1_C2 : Outport  Port=182  OutDataTypeStr=single
  IMAPve_g_ORI_R1_C1 : Outport  Port=183  OutDataTypeStr=single
  IMAPve_g_ORI_R1_C0 : Outport  Port=184  OutDataTypeStr=single
  IMAPve_d_ORI_R1_LT : Outport  Port=185  OutDataTypeStr=uint16
  IMAPve_g_ORI_R1_VR : Outport  Port=186  OutDataTypeStr=single
  IMAPve_g_ORI_R1_W : Outport  Port=187  OutDataTypeStr=single
  IMAPve_d_Sensor_Status : Outport  Port=188
  IMAPve_d_LF_Radar_Status : Outport  Port=189
  IMAPve_d_RF_Radar_Status : Outport  Port=190
  IMAPve_d_LR_Radar_Status : Outport  Port=191
  IMAPve_d_RR_Radar_Status : Outport  Port=192
  IMAPve_d_Fusion_Status : Outport  Port=193
  IMAPve_d_Fusion_Time_Stamp : Outport  Port=194
  IMAPve_d_obj_Num : Outport  Port=195
  IMAPva_d_obj_id : Outport  Port=196
  IMAPva_g_obj_pos_x : Outport  Port=197
  IMAPva_g_obj_pos_y : Outport  Port=198
  IMAPva_g_obj_vel_x : Outport  Port=199
  IMAPva_g_obj_vel_y : Outport  Port=200
  IMAPva_g_obj_acc_x : Outport  Port=201
  IMAPva_g_obj_acc_y : Outport  Port=202
  IMAPva_g_obj_pos_var_x : Outport  Port=203
  IMAPva_g_obj_pos_var_y : Outport  Port=204
  IMAPva_g_obj_pos_var_xy : Outport  Port=205
  IMAPva_g_obj_width : Outport  Port=206
  IMAPva_g_obj_length : Outport  Port=207
  IMAPva_d_obj_class : Outport  Port=208
  IMAPva_d_obj_lane : Outport  Port=209
  IMAPva_d_obj_status : Outport  Port=210
  IMAPva_d_obj_age : Outport  Port=211
  IMAPva_d_obj_TurnLight : Outport  Port=212
  IMAPva_d_obj_BrakeLight : Outport  Port=213
  IMAPva_d_obj_MotionStatus : Outport  Port=214
  IMAPve_d_Road_Type : Outport  Port=215
  IMAPve_g_L0_C0 : Outport  Port=216
  IMAPve_g_L0_C1 : Outport  Port=217
  IMAPve_g_L0_C2 : Outport  Port=218
  IMAPve_g_L0_C3 : Outport  Port=219
  IMAPve_g_L0_VR : Outport  Port=220
  IMAPve_d_L0_Q : Outport  Port=221
  IMAPve_d_L0_Type : Outport  Port=222
  IMAPve_g_L0_W : Outport  Port=223
  IMAPve_g_R0_C0 : Outport  Port=224
  IMAPve_g_R0_C1 : Outport  Port=225
  IMAPve_g_R0_C2 : Outport  Port=226
  IMAPve_g_R0_C3 : Outport  Port=227
  IMAPve_g_R0_VR : Outport  Port=228
  IMAPve_d_R0_Q : Outport  Port=229
  IMAPve_d_R0_Type : Outport  Port=230
  IMAPve_g_R0_W : Outport  Port=231
  IMAPve_g_L1_C0 : Outport  Port=232
  IMAPve_g_L1_C1 : Outport  Port=233
  IMAPve_g_L1_C2 : Outport  Port=234
  IMAPve_g_L1_C3 : Outport  Port=235
  IMAPve_g_L1_VR : Outport  Port=236
  IMAPve_d_L1_Q : Outport  Port=237
  IMAPve_d_L1_Type : Outport  Port=238
  IMAPve_g_L1_W : Outport  Port=239
  IMAPve_g_R1_C0 : Outport  Port=240
  IMAPve_g_R1_C1 : Outport  Port=241
  IMAPve_g_R1_C2 : Outport  Port=242
  IMAPve_g_R1_C3 : Outport  Port=243
  IMAPve_g_R1_VR : Outport  Port=244
  IMAPve_d_R1_Q : Outport  Port=245
  IMAPve_d_R1_Type : Outport  Port=246
  IMAPve_g_R1_W : Outport  Port=247
  IMAPve_g_L0_C0_Back : Outport  Port=248
  IMAPve_g_L0_C1_Back : Outport  Port=249
  IMAPve_g_L0_C2_Back : Outport  Port=250
  IMAPve_g_L0_C3_Back : Outport  Port=251
  IMAPve_g_L0_Range_Back : Outport  Port=252
  IMAPve_g_R0_C0_Back : Outport  Port=253
  IMAPve_g_R0_C1_Back : Outport  Port=254
  IMAPve_g_R0_C2_Back : Outport  Port=255
  IMAPve_g_R0_C3_Back : Outport  Port=256
  IMAPve_g_R0_Range_Back : Outport  Port=257
  IMAPve_g_L1_C0_Back : Outport  Port=258
  IMAPve_g_L1_C1_Back : Outport  Port=259
  IMAPve_g_L1_C2_Back : Outport  Port=260
  IMAPve_g_L1_C3_Back : Outport  Port=261
  IMAPve_g_L1_Range_Back : Outport  Port=262
  IMAPve_g_R1_C0_Back : Outport  Port=263
  IMAPve_g_R1_C1_Back : Outport  Port=264
  IMAPve_g_R1_C2_Back : Outport  Port=265
  IMAPve_g_R1_C3_Back : Outport  Port=266
  IMAPve_g_R1_Range_Back : Outport  Port=267
  IMAPve_g_Lrg_C0_BACK : Outport  Port=268
  IMAPve_g_Lrg_C1_BACK : Outport  Port=269
  IMAPve_g_Lrg_C2_BACK : Outport  Port=270
  IMAPve_g_Lrg_C3_BACK : Outport  Port=271
  IMAPve_g_Lrg_VR_Start_BACK : Outport  Port=272
  IMAPve_g_Lrg_VR_End_BACK : Outport  Port=273
  IMAPve_d_Lrg_Q_BACK : Outport  Port=274
  IMAPve_d_Lrg_TYPE_BACK : Outport  Port=275
  IMAPve_g_Rrg_C0_BACK : Outport  Port=276
  IMAPve_g_Rrg_C1_BACK : Outport  Port=277
  IMAPve_g_Rrg_C2_BACK : Outport  Port=278
  IMAPve_g_Rrg_C3_BACK : Outport  Port=279
  IMAPve_g_Rrg_VR_Start_BACK : Outport  Port=280
  IMAPve_g_Rrg_VR_End_BACK : Outport  Port=281
  IMAPve_d_Rrg_Q_BACK : Outport  Port=282
  IMAPve_d_Rrg_TYPE_BACK : Outport  Port=283
  IMAPve_d_Sign_ISA_Value : Outport  Port=284
  IMAPve_d_ISA_Popup_Message : Outport  Port=285
  IMAPve_d_ISA_Sign_Type : Outport  Port=286
  IMAPve_d_ISA_Status : Outport  Port=287
  IMAPve_d_TSR_Sign_Type : Outport  Port=288
  IMAPve_g_Camera_Signal_Fault : Outport  Port=289
  IMAPve_d_Camera_State : Outport  Port=290
  IMAPve_d_Radar_FaultBitSetting_Signal : Outport  Port=291
  IMAPve_d_Camera_Status : Outport  Port=292  OutDataTypeStr=uint16
  IMAPve_d_ESC_FLW_Direction : Outport  Port=293
  IMAPve_d_ESC_FRW_Direction : Outport  Port=294
  IMAPve_d_ESC_TCS_ErrorStatus : Outport  Port=295
  IMAPve_d_ESC_RLW_Direction : Outport  Port=296
  IMAPve_d_ESC_RRW_Direction : Outport  Port=297
  IMAPve_d_ESC_EPB_ErrorStatus : Outport  Port=298
  IMAPve_d_EPS_SteeringAngle_Flag : Outport  Port=299
  IMAPve_g_EPS_SteeringAngle : Outport  Port=300
  IMAPve_d_EPS_Driver_Override : Outport  Port=301
  IMAPve_d_EPS_Driver_Active_ESA : Outport  Port=302
  IMAPve_d_EPS_ESA_State : Outport  Port=303
  IMAPve_d_ACU_RearLeft_Belt : Outport  Port=304
  IMAPve_d_ACU_RearMiddle_Belt : Outport  Port=305
  IMAPve_d_ACU_RearRight_Belt : Outport  Port=306
  IMAPve_d_EMS_PowertrainCtl_State : Outport  Port=307
  IMAPve_d_TCU_TCU_Available : Outport  Port=308
  IMAPve_d_BCM_LeftTurn_Switch : Outport  Port=309
  IMAPve_d_BCM_RightTurn_Switch : Outport  Port=310
  IMAPve_d_BCM_FrontWiper_Switch : Outport  Port=311
  IMAPve_d_BCM_IHBC_Enabled : Outport  Port=312
  IMAPve_d_MP5_Work_State : Outport  Port=313
  IMAPve_d_MP5_APA_ModeSelect : Outport  Port=314
  IMAPve_d_MP5_LanguageSet : Outport  Port=315
  IMAPve_d_MP5_UPA_Switch : Outport  Port=316
  IMAPve_d_MP5_FLK_Activation : Outport  Port=317
  IMAPve_d_MP5_AutoPilot_Switch : Outport  Port=318
  IMAPve_d_MP5_DMS_MessageType : Outport  Port=319
  IMAPve_d_MP5_DMS_SystemEnable : Outport  Port=320
  IMAPve_d_MP5_DMS_DelUserNum : Outport  Port=321
  IMAPve_d_MP5_DMS_Sensity : Outport  Port=322
  IMAPve_d_MP5_DMS_EyeFatigue : Outport  Port=323
  IMAPve_d_MP5_DMS_LongtimeDrive : Outport  Port=324
  IMAPve_d_MP5_DMS_SideView : Outport  Port=325
  IMAPve_d_MP5_DMS_UsingPhone : Outport  Port=326
  IMAPve_d_MP5_DMS_Smoking : Outport  Port=327
  IMAPve_d_MP5_DMS_DrinkWater : Outport  Port=328
  IMAPve_d_MP5_DMS_UserAccount : Outport  Port=329
  IMAPve_g_ESC_BrkWhlCylinder_Pressure : Outport  Port=330
  IMAPva_d_ORI_Obj_TimeStamp : Outport  Port=331  OutDataTypeStr=uint16  PortDimensions=20
  IMAPve_d_ORI_FS_OutOfCalib : Outport  Port=332  OutDataTypeStr=uint16
  IMAPve_d_ORI_FS_Rain : Outport  Port=333  OutDataTypeStr=uint16
  IMAPve_d_ORI_FS_Fog : Outport  Port=334  OutDataTypeStr=uint16
  IMAPve_d_ORI_FS_Splashes0 : Outport  Port=335  OutDataTypeStr=uint16
  IMAPve_d_ORI_FS_SunRay0 : Outport  Port=336  OutDataTypeStr=uint16
  IMAPve_d_ORI_FS_LowSun0 : Outport  Port=337  OutDataTypeStr=uint16
  IMAPve_d_ORI_FS_BlurImage0 : Outport  Port=338  OutDataTypeStr=uint16
  IMAPve_d_ORI_FS_PartialBlockage0 : Outport  Port=339  OutDataTypeStr=uint16
  IMAPve_d_ORI_FS_FullBlockage0 : Outport  Port=340  OutDataTypeStr=uint16
  IMAPve_d_ORI_FS_FrozenWindshield0 : Outport  Port=341  OutDataTypeStr=uint16
  IMAPve_d_ORI_FS_OutOfFocus0 : Outport  Port=342  OutDataTypeStr=uint16
  IMAPva_g_ORI_Obj_AbsAx : Outport  Port=343  OutDataTypeStr=single  PortDimensions=20
  IMAPva_g_ORI_Obj_AbsAy : Outport  Port=344  OutDataTypeStr=single  PortDimensions=20
  IMAPva_g_ORI_Obj_RelVely : Outport  Port=345  OutDataTypeStr=single  PortDimensions=20
  IMAPva_g_ORI_Obj_LateralDis : Outport  Port=346  OutDataTypeStr=single  PortDimensions=20
  IMAPva_g_ORI_Obj_AbsAxStdDev : Outport  Port=347  OutDataTypeStr=single  PortDimensions=20
  IMAPva_g_ORI_Obj_AbsAyStdDev : Outport  Port=348  OutDataTypeStr=single  PortDimensions=20
  IMAPva_g_ORI_Obj_RelVelStdDev : Outport  Port=349  OutDataTypeStr=single  PortDimensions=20
  IMAPva_g_ORI_Obj_RelVelyStdDev : Outport  Port=350  OutDataTypeStr=single  PortDimensions=20
  IMAPva_g_ORI_Obj_LongDisStdDev : Outport  Port=351  OutDataTypeStr=single  PortDimensions=20
  IMAPva_g_ORI_Obj_LateralDisStdDev : Outport  Port=352  OutDataTypeStr=single  PortDimensions=20
  IMAPva_d_ORI_Obj_RelVelValid : Outport  Port=353  OutDataTypeStr=uint16  PortDimensions=20
  IMAPva_d_ORI_Obj_RelVelyValid : Outport  Port=354  OutDataTypeStr=uint16  PortDimensions=20
  IMAPva_d_ORI_Obj_RelVelStdDevValid : Outport  Port=355  OutDataTypeStr=uint16  PortDimensions=20
  IMAPva_d_ORI_Obj_RelVelyStdDevValid : Outport  Port=356  OutDataTypeStr=uint16  PortDimensions=20
  IMAPva_g_ORI_Obj_ExistProb : Outport  Port=357  OutDataTypeStr=single  PortDimensions=20
  IMAPva_g_ORI_Obj_ClassProb : Outport  Port=358  OutDataTypeStr=single  PortDimensions=20
  IMAPva_g_ORI_Obj_Height : Outport  Port=359  OutDataTypeStr=single  PortDimensions=20
  IMAPva_g_ORI_Obj_LengthStdDev : Outport  Port=360  OutDataTypeStr=single  PortDimensions=20
  IMAPva_g_ORI_Obj_WidthStdDev : Outport  Port=361  OutDataTypeStr=single  PortDimensions=20
  IMAPva_g_ORI_Obj_HeightStdDev : Outport  Port=362  OutDataTypeStr=single  PortDimensions=20
  IMAPva_g_ORI_Obj_3DAngle : Outport  Port=363  OutDataTypeStr=single  PortDimensions=20
  IMAPva_g_ORI_Obj_LAngleStdDev : Outport  Port=364  OutDataTypeStr=single  PortDimensions=20
  IMAPva_g_ORI_Obj_RAngleStdDev : Outport  Port=365  OutDataTypeStr=single  PortDimensions=20
  IMAPva_g_ORI_Obj_3DAngleStdDev : Outport  Port=366  OutDataTypeStr=single  PortDimensions=20
  IMAPva_g_ORI_Obj_AngleRate : Outport  Port=367  OutDataTypeStr=single  PortDimensions=20
  IMAPva_g_ORI_Obj_AngleRateStdDev : Outport  Port=368  OutDataTypeStr=single  PortDimensions=20
  IMAPva_g_ORI_Obj_PhiBottom : Outport  Port=369  OutDataTypeStr=single  PortDimensions=20
  IMAPva_g_ORI_Obj_PhiBottomStdDev : Outport  Port=370  OutDataTypeStr=single  PortDimensions=20
  IMAPva_d_ORI_Obj_Measured : Outport  Port=371  OutDataTypeStr=uint16  PortDimensions=20
  IMAPva_g_ORI_Obj_Heading : Outport  Port=372  OutDataTypeStr=single  PortDimensions=20
  IMAPva_g_ORI_Obj_HeadingStdDev : Outport  Port=373  OutDataTypeStr=single  PortDimensions=20
  IMAPva_d_ORI_Obj_HeadOrientation : Outport  Port=374  OutDataTypeStr=uint16  PortDimensions=20
  IMAPva_g_ORI_Obj_TTIPC : Outport  Port=375  OutDataTypeStr=single  PortDimensions=20
  IMAPva_g_ORI_Obj_TTIPCStdDev : Outport  Port=376  OutDataTypeStr=single  PortDimensions=20
  IMAPva_d_ORI_Obj_DirectionIndicator : Outport  Port=377  OutDataTypeStr=uint16  PortDimensions=20
  IMAPva_d_ORI_Obj_BrakeLight : Outport  Port=378  OutDataTypeStr=uint16  PortDimensions=20
  IMAPve_d_ORI_L0_ID : Outport  Port=379  OutDataTypeStr=uint16
  IMAPve_g_ORI_L0_ExistProb : Outport  Port=380  OutDataTypeStr=single
  IMAPve_g_ORI_L0_DxStart : Outport  Port=381  OutDataTypeStr=single
  IMAPve_d_ORI_L0_ColorClass : Outport  Port=382  OutDataTypeStr=uint16
  IMAPve_d_ORI_L0_MeasureType : Outport  Port=383  OutDataTypeStr=uint16
  IMAPve_g_ORI_L0_TypeConf : Outport  Port=384  OutDataTypeStr=single
  IMAPve_d_ORI_R0_ID : Outport  Port=385  OutDataTypeStr=uint16
  IMAPve_g_ORI_R0_ExistProb : Outport  Port=386  OutDataTypeStr=single
  IMAPve_g_ORI_R0_Dxstart : Outport  Port=387  OutDataTypeStr=single
  IMAPve_d_ORI_R0_ColorClass : Outport  Port=388  OutDataTypeStr=uint16
  IMAPve_d_ORI_R0_MeasureType : Outport  Port=389  OutDataTypeStr=uint16
  IMAPve_g_ORI_R0_TypeConf : Outport  Port=390  OutDataTypeStr=single
  IMAPve_d_ORI_L1_ID : Outport  Port=391  OutDataTypeStr=uint16
  IMAPve_g_ORI_L1_ExistProb : Outport  Port=392  OutDataTypeStr=single
  IMAPve_g_ORI_L1_Dxstart : Outport  Port=393  OutDataTypeStr=single
  IMAPve_d_ORI_L1_ColorClass : Outport  Port=394  OutDataTypeStr=uint16
  IMAPve_d_ORI_L1_MeasureType : Outport  Port=395  OutDataTypeStr=uint16
  IMAPve_g_ORI_L1_TypeConf : Outport  Port=396  OutDataTypeStr=single
  IMAPve_d_ORI_R1_ID : Outport  Port=397  OutDataTypeStr=uint16
  IMAPve_g_ORI_R1_ExistProb : Outport  Port=398  OutDataTypeStr=single
  IMAPve_g_ORI_R1_Dxstart : Outport  Port=399  OutDataTypeStr=single
  IMAPve_d_ORI_R1_ColorClass : Outport  Port=400  OutDataTypeStr=uint16
  IMAPve_d_ORI_R1_MeasureType : Outport  Port=401  OutDataTypeStr=uint16
  IMAPve_g_ORI_R1_TypeConf : Outport  Port=402  OutDataTypeStr=single
  IMAPve_d_ORI_RoadedgeL0_ID : Outport  Port=403  OutDataTypeStr=uint16
  IMAPve_g_ORI_RoadedgeL0_ExistProb : Outport  Port=404  OutDataTypeStr=single
  IMAPve_g_ORI_RoadedgeL0_DxStart : Outport  Port=405  OutDataTypeStr=single
  IMAPve_g_ORI_RoadedgeL0_DxEnd : Outport  Port=406  OutDataTypeStr=single
  IMAPve_g_ORI_RoadedgeL0_C1 : Outport  Port=407  OutDataTypeStr=single
  IMAPve_g_ORI_RoadedgeL0_C0 : Outport  Port=408  OutDataTypeStr=single
  IMAPve_g_ORI_RoadedgeL0_C3 : Outport  Port=409  OutDataTypeStr=single
  IMAPve_g_ORI_RoadedgeL0_C2 : Outport  Port=410  OutDataTypeStr=single
  IMAPve_d_ORI_RoadedgeL0_MeasureType : Outport  Port=411  OutDataTypeStr=uint16
  IMAPve_d_ORI_RoadedgeL0_Type : Outport  Port=412  OutDataTypeStr=uint16
  IMAPve_d_ORI_RoadedgeR0_ID : Outport  Port=413  OutDataTypeStr=uint16
  IMAPve_g_ORI_RoadedgeR0_ExistProb : Outport  Port=414  OutDataTypeStr=single
  IMAPve_g_ORI_RoadedgeR0_DxStart : Outport  Port=415  OutDataTypeStr=single
  IMAPve_g_ORI_RoadedgeR0_DxEnd : Outport  Port=416  OutDataTypeStr=single
  IMAPve_g_ORI_RoadedgeR0_C1 : Outport  Port=417  OutDataTypeStr=single
  IMAPve_g_ORI_RoadedgeR0_C0 : Outport  Port=418  OutDataTypeStr=single
  IMAPve_g_ORI_RoadedgeR0_C3 : Outport  Port=419  OutDataTypeStr=single
  IMAPve_g_ORI_RoadedgeR0_C2 : Outport  Port=420  OutDataTypeStr=single
  IMAPve_d_ORI_RoadedgeR0_MeasureType : Outport  Port=421  OutDataTypeStr=uint16
  IMAPve_d_ORI_RoadedgeR0_Type : Outport  Port=422  OutDataTypeStr=uint16
  IMAPve_d_APA_AutoPark_WorkSt : Outport  Port=423
  IMAPve_g_ob020H_100 : Outport  Port=424
  IMAPve_g_ob020L_100 : Outport  Port=425
  wires:
  Data Type Conversion63/1 -> Terminator143/1  "ob_IMAPve_d_Rrg_Q_BACK"
  Gain131/1 -> Data Type Conversion63/1, IMAPve_d_Rrg_Q_BACK/1  "IMAPve_d_Rrg_Q_BACK"
  SDFAve_y_Rrg_DETECT_QUALITY/1 -> Gain131/1
  Gain132/1 -> Data Type Conversion66/1, IMAPve_d_Rrg_TYPE_BACK/1  "IMAPve_d_Rrg_TYPE_BACK"
  Data Type Conversion66/1 -> Terminator142/1  "ob_IMAPve_d_Rrg_TYPE_BACK"
  SDFAve_y_Rrg_LINE_TYPE/1 -> Gain132/1
  SDFAve_y_Lrg_LINE_TYPE/1 -> Gain130/1
  Gain130/1 -> Data Type Conversion57/1, IMAPve_d_Lrg_TYPE_BACK/1  "IMAPve_d_Lrg_TYPE_BACK"
  SDFAve_y_Lrg_DETECT_QUALITY/1 -> Gain128/1
  Data Type Conversion57/1 -> Terminator134/1  "ob_IMAPve_d_Lrg_TYPE_BACK"
  Gain128/1 -> Data Type Conversion41/1, IMAPve_d_Lrg_Q_BACK/1  "IMAPve_d_Lrg_Q_BACK"
  Data Type Conversion41/1 -> Terminator137/1  "ob_IMAPve_d_Lrg_Q_BACK"
  SDFAve_g_Rrg_VIEW_RANGE_end/1 -> Gain127/1
  SDFAve_g_Rrg_C0_BACK_COEF/1 -> Gain13/1
  Gain127/1 -> Data Type Conversion33/1, IMAPve_g_Rrg_VR_End_BACK/1  "IMAPve_g_Rrg_VR_End_BACK"
  SDFAve_g_Rrg_VIEW_RANGE_start/1 -> Gain107/1
  SDFAve_g_Rrg_C2_BACK_COEF/1 -> Gain14/1
  Data Type Conversion33/1 -> Terminator54/1  "ob_IMAPve_g_Rrg_VR_End_BACK"
  Gain110/1 -> Data Type Conversion17/1, IMAPve_g_Rrg_C1_BACK/1  "IMAPve_g_Rrg_C1_BACK"
  Data Type Conversion26/1 -> Terminator124/1  "ob_IMAPve_g_Rrg_C3_BACK"
  Data Type Conversion25/1 -> Terminator109/1  "ob_IMAPve_g_Rrg_C2_BACK"
  Gain106/1 -> Data Type Conversion26/1, IMAPve_g_Rrg_C3_BACK/1  "IMAPve_g_Rrg_C3_BACK"
  Gain14/1 -> Data Type Conversion25/1, IMAPve_g_Rrg_C2_BACK/1  "IMAPve_g_Rrg_C2_BACK"
  SDFAve_g_Rrg_C3_BACK_COEF/1 -> Gain106/1
  Gain107/1 -> Data Type Conversion27/1, IMAPve_g_Rrg_VR_Start_BACK/1  "IMAPve_g_Rrg_VR_Start_BACK"
  Data Type Conversion17/1 -> Terminator63/1  "ob_IMAPve_g_Rrg_C1_BACK"
  Data Type Conversion27/1 -> Terminator132/1  "ob_IMAPve_g_Rrg_VR_Start_BACK"
  SDFAve_g_Rrg_C1_BACK_COEF/1 -> Gain110/1
  Gain13/1 -> Data Type Conversion16/1, IMAPve_g_Rrg_C0_BACK/1  "IMAPve_g_Rrg_C0_BACK"
  Data Type Conversion16/1 -> Terminator57/1  "ob_IMAPve_g_Rrg_C0_BACK"
  SDFAve_g_Lrg_VIEW_RANGE_end/1 -> Gain126/1
  Gain126/1 -> Data Type Conversion28/1, IMAPve_g_Lrg_VR_End_BACK/1  "IMAPve_g_Lrg_VR_End_BACK"
  Data Type Conversion28/1 -> Terminator125/1  "ob_IMAPve_g_Lrg_VR_End_BACK"
  Data Type Conversion13/1 -> Terminator26/1  "ob_IMAPve_g_Lrg_C2_BACK"
  Gain123/1 -> Data Type Conversion11/1, IMAPve_g_Lrg_C1_BACK/1  "IMAPve_g_Lrg_C1_BACK"
  SDFAve_g_Lrg_C2_BACK_COEF/1 -> Gain116/1
  SDFAve_g_Lrg_VIEW_RANGE_start/1 -> Gain118/1
  SDFAve_g_Lrg_C0_BACK_COEF/1 -> Gain115/1
  Data Type Conversion11/1 -> Terminator18/1  "ob_IMAPve_g_Lrg_C1_BACK"
  Gain118/1 -> Data Type Conversion15/1, IMAPve_g_Lrg_VR_Start_BACK/1  "IMAPve_g_Lrg_VR_Start_BACK"
  SDFAve_g_Lrg_C3_BACK_COEF/1 -> Gain117/1
  Gain116/1 -> Data Type Conversion13/1, IMAPve_g_Lrg_C2_BACK/1  "IMAPve_g_Lrg_C2_BACK"
  Gain115/1 -> Data Type Conversion10/1, IMAPve_g_Lrg_C0_BACK/1  "IMAPve_g_Lrg_C0_BACK"
  Gain117/1 -> Data Type Conversion14/1, IMAPve_g_Lrg_C3_BACK/1  "IMAPve_g_Lrg_C3_BACK"
  Data Type Conversion14/1 -> Terminator32/1  "ob_IMAPve_g_Lrg_C3_BACK"
  Data Type Conversion10/1 -> Terminator17/1  "ob_IMAPve_g_Lrg_C0_BACK"
  Data Type Conversion15/1 -> Terminator48/1  "ob_IMAPve_g_Lrg_VR_Start_BACK"
  SDFAve_g_Lrg_C1_BACK_COEF/1 -> Gain123/1
  SWINve_y_T_box_RemoteHazardReq/1 -> AND/3
  SWINve_y_MP5_HazardLampCtrlReq/1 -> AND/2
  SWINve_y_BCM_HazardSwitchrSt/1 -> AND/1
  AND/1 -> Switch175/3
  Switch175/1 -> Gain8/1  "IMAPve_d_BCM_HazardLamp_Switch"
  Data Type Conversion12/1 -> Terminator19/1  "ob_IMAPve_d_BCM_HazardLamp_Switch"
  Constant351/1 -> Switch175/1
  Gain8/1 -> Data Type Conversion12/1, IMAPve_d_BCM_HazardLamp_Switch/1
  Constant352/1 -> Switch175/2
  array_transfer10/1(output) -> Switch26/3
  Gain185/1 -> IMAPve_d_FCW_Switch/1, Data Type Conversion37/1
  Data Type Conversion393/1 -> Terminator389/1  "ob_IMAPva_g_ORI_Obj_AbsAy"
  Data Type Conversion84/1 -> Terminator75/1  "ob_IMAPve_g_EMS_Realize_TWhl"
  Data Type Conversion60/1 -> Terminator51/1  "ob_IMAPve_d_BCM_HighBeam_State"
  Data Type Conversion79/1 -> Terminator70/1  "ob_IMAPve_g_EMS_MaxTWhl"
  ? -> Gain362/1
  Data Type Conversion480/1 -> Terminator461/1  "ob_IMAPve_d_ORI_RoadedgeR0_Type"
  Data Type Conversion455/1 -> Terminator436/1  "ob_IMAPve_g_ORI_L1_ExistProb"
  Gain397/1 -> IMAPve_g_ORI_L0_DxStart/1, Data Type Conversion444/1  "IMAPve_g_ORI_L0_DxStart"
  Gain317/1 -> Data Type Conversion31/1, IMAPve_d_BCM_Door_Lock_State/1
  ? -> Gain426/1
  Gain389/1 -> Data Type Conversion448/1, IMAPve_d_ORI_R0_ID/1
  Gain442/1 -> Data Type Conversion486/1, IMAPve_g_ESC_BrkWhlCylinder_Pressure/1
  ? -> Gain428/1
  Data Type Conversion292/1 -> Terminator283/1  "ob_IMAPve_g_R0_C1_Back"
  ? -> Gain397/1
  Data Type Conversion223/1 -> Terminator214/1  "ob_IMAPva_d_obj_lane"
  Data Type Conversion83/1 -> Terminator74/1  "ob_IMAPve_g_EMS_Actual_FlwT"
  Gain418/1 -> Data Type Conversion419/1, IMAPva_d_ORI_Obj_RelVelStdDevValid/1  "IMAPva_d_ORI_Obj_RelVelStdDevValid"
  SDFAve_g_L0_BACK_RANGE/1 -> Gain129/1
  Gain187/1 -> IMAPve_d_ISA_Switch/1, Data Type Conversion39/1
  Constant19/1 -> Gain447/1
  Gain304/1 -> Data Type Conversion1/1, IMAPve_d_ISA_ISLC_Mode/1
  Gain404/1 -> IMAPva_d_ORI_Obj_Measured/1, Data Type Conversion435/1  "IMAPva_d_ORI_Obj_Measured"
  ? -> Gain408/1
  Data Type Conversion98/1 -> Terminator89/1  "ob_IMAPve_d_TCU_Gear_Engage"
  Data Type Conversion409/1 -> Terminator338/1  "ob_IMAPve_d_BCM_IHBC_Enabled"
  Gain447/1 -> IMAPve_g_ob020L_100/1  "IMAPve_g_ob020L_100"
  Gain320/1 -> Data Type Conversion342/1, IMAPve_d_TBOX_LocalTimeY/1
  Data Type Conversion341/1 -> Terminator332/1  "ob_IMAPve_d_ORI_FS_FullBlockage0"
  Data Type Conversion384/1 -> Terminator380/1  "ob_IMAPve_d_EPB_Switch_State"
  ? -> Gain402/1
  Data Type Conversion4/1 -> Terminator5/1  "ob_IMAPve_d_ALC_TLC_Mode"
  FAPAve_Cnt_AdvancedParkingAssist/1 -> Gain445/1
  Data Type Conversion202/1 -> Terminator193/1  "ob_IMAPve_g_Camera_Signal_Fault"
  Data Type Conversion322/1 -> Terminator313/1  "ob_IMAPve_d_ESC_RLW_Direction"
  Data Type Conversion294/1 -> Terminator285/1  "ob_IMAPve_g_R0_C3_Back"
  Data Type Conversion473/1 -> Terminator454/1  "ob_IMAPve_g_ORI_RoadedgeR0_ExistProb"
  SDFAva_y_obj_BrakeLight/1 -> Gain205/1
  Gain297/1 -> Data Type Conversion225/1, IMAPve_d_MP5_DMS_EyeFatigue/1  "IMAPve_d_MP5_DMS_EyeFatigue"
  SDFAve_g_R0_C3_COEF/1 -> Gain167/1
  ? -> Gain360/1
  Gain445/1 -> MATLAB Function/1(APA_FAPA_WorkSt)
  Gain2/1 -> Data Type Conversion140/1, IMAPve_d_ORI_Obj_Num/1  "IMAPve_d_ORI_Obj_Num"
  Data Type Conversion37/1 -> Terminator28/1  "ob_IMAPve_d_FCW_Switch"
  Data Type Conversion362/1 -> Terminator360/1  "ob_IMAPve_g_EPS_PowerCon"
  Gain22/1 -> Data Type Conversion105/1, IMAPve_g_ESC_Brake_Press/1
  Data Type Conversion447/1 -> Terminator428/1  "ob_IMAPve_d_ORI_R0_MeasureType"
  Data Type Conversion485/1 -> Terminator466/1  "ob_IMAPve_d_ORI_R1_ColorClass"
  Gain438/1 -> Data Type Conversion334/1, IMAPve_d_ORI_FS_Rain/1  "IMAPve_d_ORI_FS_Rain"
  Data Type Conversion423/1 -> Terminator404/1  "ob_IMAPva_g_ORI_Obj_Height"
  Gain10/1 -> Data Type Conversion148/1, IMAPva_g_ORI_Obj_RAngle/1  "IMAPva_g_ORI_Obj_RAngle"
  Gain108/1 -> Data Type Conversion200/1, IMAPve_d_Sign_ISA_Value/1  "IMAPve_d_Sign_ISA_Value"
  Data Type Conversion396/1 -> Terminator392/1  "ob_IMAPva_g_ORI_Obj_AbsAxStdDev"
  Gain431/1 -> Data Type Conversion340/1, IMAPve_d_ORI_FS_PartialBlockage0/1  "IMAPve_d_ORI_FS_PartialBlockage0"
  Gain229/1 -> Data Type Conversion194/1, IMAPve_d_LF_Radar_Status/1  "IMAPve_d_LF_Radar_Status"
  Gain444/1 -> Data Type Conversion394/1, IMAPva_g_ORI_Obj_RelVely/1  "IMAPva_g_ORI_Obj_RelVely"
  Data Type Conversion337/1 -> Terminator328/1  "ob_IMAPve_d_ORI_FS_SunRay0"
  Gain330/1 -> Data Type Conversion361/1, IMAPve_d_EPS_Warning_State/1
  Gain421/1 -> Data Type Conversion401/1, IMAPva_g_ORI_Obj_LateralDisStdDev/1  "IMAPva_g_ORI_Obj_LateralDisStdDev"
  Gain420/1 -> Data Type Conversion403/1, IMAPva_d_ORI_Obj_RelVelValid/1  "IMAPva_d_ORI_Obj_RelVelValid"
  Data Type Conversion263/1 -> Terminator254/1  "ob_IMAPve_g_L1_C3"
  ? -> Gain383/1
  Gain446/1 -> IMAPve_g_ob020H_100/1  "IMAPve_g_ob020H_100"
  ? -> Gain410/1
  Data Type Conversion20/1 -> Terminator11/1  "ob_IMAPve_d_FCTA_Switch"
  Data Type Conversion325/1 -> Terminator316/1  "ob_IMAPve_d_EPS_SteeringAngle_Flag"
  Gain163/1 -> Data Type Conversion266/1, IMAPve_d_L1_Type/1  "IMAPve_d_L1_Type"
  Constant18/1 -> Gain446/1
  Gain424/1 -> Data Type Conversion398/1, IMAPva_g_ORI_Obj_RelVelStdDev/1  "IMAPva_g_ORI_Obj_RelVelStdDev"
  Gain34/1 -> Data Type Conversion82/1, IMAPve_g_EMS_MinTWhl_Offset/1
  SDFAve_d_ORI_R1_LT/1 -> Gain241/1
  Data Type Conversion273/1 -> Terminator264/1  "ob_IMAPve_g_R1_C2"
  Data Type Conversion456/1 -> Terminator437/1  "ob_IMAPve_g_ORI_L1_Dxstart"
  Data Type Conversion126/1 -> Terminator118/1  "ob_IMAPve_g_ESC_RR_WhlSpd"
  Gain365/1 -> Data Type Conversion469/1, IMAPve_g_ORI_RoadedgeR0_DxStart/1  "IMAPve_g_ORI_RoadedgeR0_DxStart"
  Gain376/1 -> Data Type Conversion483/1, IMAPve_g_ORI_R1_ExistProb/1  "IMAPve_g_ORI_R1_ExistProb"
  SDFAve_g_R1_C0_COEF/1 -> Gain150/1
  Data Type Conversion24/1 -> Terminator15/1  "ob_IMAPve_d_JA_Alert_Switch"
  Data Type Conversion361/1 -> Terminator359/1  "ob_IMAPve_d_EPS_Warning_State"
  Data Type Conversion418/1 -> Terminator399/1  "ob_IMAPva_d_ORI_Obj_RelVelyValid"
  Gain124/1 -> Data Type Conversion301/1, IMAPve_g_L1_C1_Back/1  "IMAPve_g_L1_C1_Back"
  Gain439/1 -> Data Type Conversion333/1, IMAPve_d_ORI_FS_OutOfCalib/1  "IMAPve_d_ORI_FS_OutOfCalib"
  Data Type Conversion474/1 -> Terminator455/1  "ob_IMAPve_g_ORI_RoadedgeR0_DxEnd"
  Data Type Conversion479/1 -> Terminator460/1  "ob_IMAPve_d_ORI_RoadedgeR0_MeasureType"
  Data Type Conversion265/1 -> Terminator256/1  "ob_IMAPve_d_L1_Q"
  Data Type Conversion131/1 -> Terminator123/1  "ob_IMAPve_d_ESC_Brake_Failsafe"
  Gain206/1 -> Data Type Conversion230/1, IMAPva_d_obj_MotionStatus/1  "IMAPva_d_obj_MotionStatus"
  Data Type Conversion392/1 -> Terminator388/1  "ob_IMAPva_g_ORI_Obj_AbsAx"
  Data Type Conversion471/1 -> Terminator452/1  "ob_IMAPve_d_ORI_RoadedgeL0_Type"
  Data Type Conversion427/1 -> Terminator408/1  "ob_IMAPva_g_ORI_Obj_3DAngle"
  ? -> Gain423/1
  Data Type Conversion467/1 -> Terminator448/1  "ob_IMAPve_g_ORI_RoadedgeL0_C0"
  Data Type Conversion466/1 -> Terminator447/1  "ob_IMAPve_g_ORI_RoadedgeL0_C1"
  SDFAva_g_obj_width/1 -> Gain213/1
  ? -> Gain424/1
  Data Type Conversion461/1 -> Terminator442/1  "ob_IMAPve_d_ORI_RoadedgeL0_ID"
  Data Type Conversion375/1 -> Terminator371/1  "ob_IMAPve_d_ESC_FR_WhlSpd_Fault"
  Data Type Conversion450/1 -> Terminator431/1  "ob_IMAPve_g_ORI_R0_Dxstart"
  Gain165/1 -> Data Type Conversion250/1, IMAPve_g_R0_C1/1  "IMAPve_g_R0_C1"
  Data Type Conversion457/1 -> Terminator438/1  "ob_IMAPve_d_ORI_L1_ColorClass"
  Gain277/1 -> IMAPve_g_ORI_L0_C3/1, Data Type Conversion154/1  "IMAPve_g_ORI_L0_C3"
  Data Type Conversion379/1 -> Terminator375/1  "ob_IMAPve_d_ESC_AEB_Active"
  SDFAve_g_L0_C1_COEF/1 -> Gain199/1
  Data Type Conversion458/1 -> Terminator439/1  "ob_IMAPve_d_ORI_L1_MeasureType"
  Data Type Conversion381/1 -> Terminator377/1  "ob_IMAPve_d_ESC_ACC_Active"
  Gain364/1 -> Data Type Conversion473/1, IMAPve_g_ORI_RoadedgeR0_ExistProb/1  "IMAPve_g_ORI_RoadedgeR0_ExistProb"
  Data Type Conversion448/1 -> Terminator429/1  "ob_IMAPve_d_ORI_R0_ID"
  Data Type Conversion445/1 -> Terminator426/1  "ob_IMAPve_d_ORI_L0_ColorClass"
  Data Type Conversion446/1 -> Terminator427/1  "ob_IMAPve_d_ORI_L0_MeasureType"
  Data Type Conversion419/1 -> Terminator400/1  "ob_IMAPva_d_ORI_Obj_RelVelStdDevValid"
  Gain100/1 -> Data Type Conversion62/1, IMAPve_g_GW_IC_Odometer/1
  ? -> Gain390/1
  Data Type Conversion429/1 -> Terminator410/1  "ob_IMAPva_g_ORI_Obj_RAngleStdDev"
  Data Type Conversion435/1 -> Terminator416/1  "ob_IMAPva_d_ORI_Obj_Measured"
  Data Type Conversion434/1 -> Terminator415/1  "ob_IMAPva_g_ORI_Obj_PhiBottomStdDev"
  ? -> Gain400/1
  Data Type Conversion334/1 -> Terminator325/1  "ob_IMAPve_d_ORI_FS_Rain"
  Data Type Conversion472/1 -> Terminator453/1  "ob_IMAPve_d_ORI_RoadedgeR0_ID"
  Data Type Conversion433/1 -> Terminator414/1  "ob_IMAPva_g_ORI_Obj_PhiBottom"
  Gain429/1 -> Data Type Conversion338/1, IMAPve_d_ORI_FS_LowSun0/1  "IMAPve_d_ORI_FS_LowSun0"
  Gain401/1 -> Data Type Conversion430/1, IMAPva_g_ORI_Obj_3DAngleStdDev/1  "IMAPva_g_ORI_Obj_3DAngleStdDev"
  Data Type Conversion432/1 -> Terminator413/1  "ob_IMAPva_g_ORI_Obj_AngleRateStdDev"
  ? -> Gain438/1
  Data Type Conversion424/1 -> Terminator405/1  "ob_IMAPva_g_ORI_Obj_LengthStdDev"
  Data Type Conversion336/1 -> Terminator327/1  "ob_IMAPve_d_ORI_FS_Splashes0"
  Data Type Conversion422/1 -> Terminator403/1  "ob_IMAPva_g_ORI_Obj_ClassProb"
  Data Type Conversion431/1 -> Terminator412/1  "ob_IMAPva_g_ORI_Obj_AngleRate"
  ? -> Gain395/1
  Data Type Conversion425/1 -> Terminator406/1  "ob_IMAPva_g_ORI_Obj_WidthStdDev"
  Data Type Conversion459/1 -> Terminator440/1  "ob_IMAPve_d_ORI_R1_MeasureType"
  Data Type Conversion463/1 -> Terminator444/1  "ob_IMAPve_g_ORI_RoadedgeL0_ExistProb"
  Data Type Conversion128/1 -> Terminator120/1  "ob_IMAPve_d_ESC_FR_Wheel_Pulse"
  Gain289/1 -> Data Type Conversion46/1, IMAPve_d_BCM_RR_Door_State/1, array_transfer11/4(RR_Door)
  ? -> Gain401/1
  Data Type Conversion454/1 -> Terminator435/1  "ob_IMAPve_d_ORI_L1_ID"
  Data Type Conversion400/1 -> Terminator396/1  "ob_IMAPva_g_ORI_Obj_LongDisStdDev"
  Data Type Conversion391/1 -> Terminator387/1  "ob_IMAPva_g_ORI_Obj_TTIPCStdDev"
  Data Type Conversion85/1 -> Terminator76/1  "ob_IMAPve_g_EMS_ACC_VirtualPedal"
  Gain428/1 -> Data Type Conversion337/1, IMAPve_d_ORI_FS_SunRay0/1  "IMAPve_d_ORI_FS_SunRay0"
  Data Type Conversion395/1 -> Terminator391/1  "ob_IMAPva_g_ORI_Obj_LateralDis"
  Data Type Conversion333/1 -> Terminator324/1  "ob_IMAPve_d_ORI_FS_OutOfCalib"
  Data Type Conversion339/1 -> Terminator330/1  "ob_IMAPve_d_ORI_FS_BlurImage0"
  Data Type Conversion332/1 -> Terminator323/1  "ob_IMAPva_d_ORI_Obj_TimeStamp"
  Gain427/1 -> Data Type Conversion395/1, IMAPva_g_ORI_Obj_LateralDis/1  "IMAPva_g_ORI_Obj_LateralDis"
  Data Type Conversion399/1 -> Terminator395/1  "ob_IMAPva_g_ORI_Obj_RelVelyStdDev"
  ? -> Gain440/1
  Gain440/1 -> Data Type Conversion336/1, IMAPve_d_ORI_FS_Splashes0/1  "IMAPve_d_ORI_FS_Splashes0"
  Gain437/1 -> IMAPve_d_ORI_FS_FullBlockage0/1, Data Type Conversion341/1  "IMAPve_d_ORI_FS_FullBlockage0"
  ? -> Gain439/1
  Gain434/1 -> Data Type Conversion391/1, IMAPva_g_ORI_Obj_TTIPCStdDev/1  "IMAPva_g_ORI_Obj_TTIPCStdDev"
  Gain433/1 -> Data Type Conversion392/1, IMAPva_g_ORI_Obj_AbsAx/1  "IMAPva_g_ORI_Obj_AbsAx"
  Gain84/1 -> Data Type Conversion319/1, IMAPve_d_ESC_FLW_Direction/1
  ? -> Gain437/1
  Data Type Conversion115/1 -> Terminator107/1  "ob_IMAPve_d_ESC_TCS_Active"
  Gain280/1 -> Data Type Conversion69/1, IMAPve_d_EPS_TrqLim_State/1
  Gain430/1 -> Data Type Conversion339/1, IMAPve_d_ORI_FS_BlurImage0/1  "IMAPve_d_ORI_FS_BlurImage0"
  Gain189/1 -> Data Type Conversion64/1, IMAPve_d_EPS_LKA_State/1
  Gain288/1 -> Data Type Conversion463/1, IMAPve_g_ORI_RoadedgeL0_ExistProb/1  "IMAPve_g_ORI_RoadedgeL0_ExistProb"
  Gain370/1 -> Data Type Conversion478/1, IMAPve_g_ORI_RoadedgeR0_C2/1  "IMAPve_g_ORI_RoadedgeR0_C2"
  ? -> Gain430/1
  Data Type Conversion217/1 -> Terminator208/1  "ob_IMAPve_d_MP5_DMS_SystemEnable"
  ? -> Gain422/1
  ? -> Gain387/1
  Gain71/1 -> Data Type Conversion89/1, IMAPve_d_EMS_Engine_Status/1
  Data Type Conversion437/1 -> Terminator418/1  "ob_IMAPva_g_ORI_Obj_HeadingStdDev"
  Data Type Conversion475/1 -> Terminator456/1  "ob_IMAPve_g_ORI_RoadedgeR0_C1"
  ? -> Gain415/1
  ? -> Gain420/1
  Gain414/1 -> Data Type Conversion426/1, IMAPva_g_ORI_Obj_HeightStdDev/1  "IMAPva_g_ORI_Obj_HeightStdDev"
  Gain408/1 -> Data Type Conversion431/1, IMAPva_g_ORI_Obj_AngleRate/1  "IMAPva_g_ORI_Obj_AngleRate"
  Data Type Conversion166/1 -> Terminator157/1  "ob_IMAPve_g_ORI_L1_C1"
  Data Type Conversion468/1 -> Terminator449/1  "ob_IMAPve_g_ORI_RoadedgeL0_C3"
  Gain405/1 -> IMAPva_g_ORI_Obj_Heading/1, Data Type Conversion436/1  "IMAPva_g_ORI_Obj_Heading"
  Switch26/1 -> Data Type Conversion8/1
  Gain155/1 -> Data Type Conversion276/1, IMAPve_d_R1_Q/1  "IMAPve_d_R1_Q"
  Gain395/1 -> IMAPve_d_ORI_L0_ID/1, Data Type Conversion442/1  "IMAPve_d_ORI_L0_ID"
  ? -> Gain394/1
  ? -> Gain356/1
  Data Type Conversion340/1 -> Terminator331/1  "ob_IMAPve_d_ORI_FS_PartialBlockage0"
  Gain236/1 -> Data Type Conversion206/1, IMAPva_d_obj_id/1  "IMAPva_d_obj_id"
  Gain125/1 -> Data Type Conversion295/1, IMAPve_g_R0_Range_Back/1  "IMAPve_g_R0_Range_Back"
  Gain394/1 -> IMAPva_d_ORI_Obj_BrakeLight/1, Data Type Conversion441/1  "IMAPva_d_ORI_Obj_BrakeLight"
  ? -> Gain403/1
  ? -> Gain384/1
  ? -> Gain393/1
  ? -> Gain421/1
  Data Type Conversion414/1 -> Terminator343/1  "ob_IMAPve_d_MP5_LanguageSet"
  Data Type Conversion107/1 -> Terminator98/1  "ob_IMAPve_g_ESC_DySlope_Accuracy"
  Gain161/1 -> Data Type Conversion264/1, IMAPve_g_L1_VR/1  "IMAPve_g_L1_VR"
  ? -> Gain382/1
  Data Type Conversion38/1 -> Terminator29/1  "ob_IMAPve_d_FCW_Sensitivity"
  Gain381/1 -> Data Type Conversion456/1, IMAPve_g_ORI_L1_Dxstart/1  "IMAPve_g_ORI_L1_Dxstart"
  Gain383/1 -> Data Type Conversion454/1, IMAPve_d_ORI_L1_ID/1  "IMAPve_d_ORI_L1_ID"
  SDFAve_d_sen_sta_RB_radar/1 -> Gain232/1
  ? -> Gain370/1
  Data Type Conversion207/1 -> Terminator198/1  "ob_IMAPva_g_obj_pos_x"
  ? -> Gain372/1
  Gain371/1 -> Data Type Conversion479/1, IMAPve_d_ORI_RoadedgeR0_MeasureType/1  "IMAPve_d_ORI_RoadedgeR0_MeasureType"
  Data Type Conversion335/1 -> Terminator326/1  "ob_IMAPve_d_ORI_FS_Fog"
  Data Type Conversion444/1 -> Terminator425/1  "ob_IMAPve_g_ORI_L0_DxStart"
  Data Type Conversion416/1 -> Terminator345/1  "ob_IMAPve_d_MP5_FLK_Activation"
  Gain129/1 -> Data Type Conversion286/1, IMAPve_g_L0_Range_Back/1  "IMAPve_g_L0_Range_Back"
  Data Type Conversion460/1 -> Terminator441/1  "ob_IMAPve_g_ORI_R1_TypeConf"
  Gain368/1 -> Data Type Conversion476/1, IMAPve_g_ORI_RoadedgeR0_C0/1  "IMAPve_g_ORI_RoadedgeR0_C0"
  Data Type Conversion112/1 -> Terminator104/1  "ob_IMAPve_d_ESC_AlarmSig"
  ? -> Gain367/1
  ? -> Gain368/1
  Gain367/1 -> Data Type Conversion475/1, IMAPve_g_ORI_RoadedgeR0_C1/1  "IMAPve_g_ORI_RoadedgeR0_C1"
  SDFAve_g_ORI_L0_VR/1 -> Gain274/1
  Gain415/1 -> Data Type Conversion422/1, IMAPva_g_ORI_Obj_ClassProb/1  "IMAPva_g_ORI_Obj_ClassProb"
  Data Type Conversion387/1 -> Terminator383/1  "ob_IMAPve_d_ESC_AVH_Status"
  Gain366/1 -> Data Type Conversion474/1, IMAPve_g_ORI_RoadedgeR0_DxEnd/1  "IMAPve_g_ORI_RoadedgeR0_DxEnd"
  ? -> Gain359/1
  ? -> Gain366/1
  Data Type Conversion382/1 -> Terminator378/1  "ob_IMAPve_d_EPB_Display_Req"
  Gain363/1 -> IMAPve_d_ORI_RoadedgeR0_ID/1, Data Type Conversion472/1  "IMAPve_d_ORI_RoadedgeR0_ID"
  Gain270/1 -> IMAPve_g_ORI_L0_C1/1, Data Type Conversion156/1  "IMAPve_g_ORI_L0_C1"
  Gain407/1 -> Data Type Conversion438/1, IMAPva_d_ORI_Obj_HeadOrientation/1  "IMAPva_d_ORI_Obj_HeadOrientation"
  Gain135/1 -> Data Type Conversion292/1, IMAPve_g_R0_C1_Back/1  "IMAPve_g_R0_C1_Back"
  Gain204/1 -> Data Type Conversion228/1, IMAPva_d_obj_TurnLight/1  "IMAPva_d_obj_TurnLight"
  Data Type Conversion93/1 -> Terminator84/1  "ob_IMAPve_d_EMS_ACC_Inhibited"
  ? -> Gain363/1
  Gain331/1 -> Data Type Conversion362/1, IMAPve_g_EPS_PowerCon/1
  Gain86/1 -> Data Type Conversion135/1, IMAPve_d_ESC_Drive_Direction/1
  Gain18/1 -> Data Type Conversion101/1, IMAPve_g_ESC_YawRate/1
  Data Type Conversion330/1 -> Terminator321/1  "ob_IMAPve_d_EPS_ESA_State"
  Gain/1 -> Data Type Conversion460/1, IMAPve_g_ORI_R1_TypeConf/1  "IMAPve_g_ORI_R1_TypeConf"
  Gain362/1 -> Data Type Conversion471/1, IMAPve_d_ORI_RoadedgeL0_Type/1  "IMAPve_d_ORI_RoadedgeL0_Type"
  Gain355/1 -> Data Type Conversion465/1, IMAPve_g_ORI_RoadedgeL0_DxEnd/1  "IMAPve_g_ORI_RoadedgeL0_DxEnd"
  Gain237/1 -> IMAPve_g_ORI_R1_C2/1, Data Type Conversion185/1  "IMAPve_g_ORI_R1_C2"
  ? -> Gain288/1
  ? -> Gain389/1
  ? -> Gain354/1
  ? -> Gain357/1
  Gain92/1 -> Data Type Conversion323/1, IMAPve_d_ESC_RRW_Direction/1
  Gain302/1 -> Data Type Conversion234/1, IMAPve_d_MP5_DMS_DrinkWater/1  "IMAPve_d_MP5_DMS_DrinkWater"
  Data Type Conversion301/1 -> Terminator292/1  "ob_IMAPve_g_L1_C1_Back"
  ? -> Gain379/1
  SDFAva_g_obj_pos_y/1 -> Gain220/1
  ? -> Gain381/1
  Data Type Conversion312/1 -> Terminator303/1  "ob_IMAPve_g_R1_C3_Back"
  ? -> Gain413/1
  Data Type Conversion5/1 -> Terminator6/1  "ob_IMAPve_d_ESA_Switch"
  Gain413/1 -> Data Type Conversion425/1, IMAPva_g_ORI_Obj_WidthStdDev/1  "IMAPva_g_ORI_Obj_WidthStdDev"
  Gain419/1 -> Data Type Conversion418/1, IMAPva_d_ORI_Obj_RelVelyValid/1  "IMAPva_d_ORI_Obj_RelVelyValid"
  Data Type Conversion483/1 -> Terminator464/1  "ob_IMAPve_g_ORI_R1_ExistProb"
  Data Type Conversion385/1 -> Terminator381/1  "ob_IMAPve_d_EPB_Switch_Valid"
  ? -> Gain391/1
  Data Type Conversion476/1 -> Terminator457/1  "ob_IMAPve_g_ORI_RoadedgeR0_C0"
  ? -> Gain431/1
  Data Type Conversion486/1 -> Terminator467/1  "ob_IMAPve_g_ESC_BrkWhlCylinder_Pressure"
  Data Type Conversion462/1 -> Terminator443/1  "ob_IMAPve_g_ORI_RoadedgeL0_C2"
  Gain45/1 -> Data Type Conversion95/1, IMAPve_d_TCU_Target_Gear/1
  Data Type Conversion184/1 -> Terminator175/1  "ob_IMAPve_g_ORI_R1_C3"
  Data Type Conversion441/1 -> Terminator422/1  "ob_IMAPva_d_ORI_Obj_BrakeLight"
  Data Type Conversion478/1 -> Terminator459/1  "ob_IMAPve_g_ORI_RoadedgeR0_C2"
  Data Type Conversion2/1 -> Terminator3/1  "ob_IMAPve_d_LDW_Warn_Mode"
  MATLAB Function/1(IMAP_FAPA_WorkSt) -> Data Type Conversion487/1, IMAPve_d_APA_AutoPark_WorkSt/1  "IMAPve_d_APA_AutoPark_WorkSt"
  Data Type Conversion18/1 -> Terminator9/1  "ob_IMAPve_d_PEPS_RKE_Command"
  Gain378/1 -> Data Type Conversion482/1, IMAPve_d_ORI_R1_ID/1  "IMAPve_d_ORI_R1_ID"
  ? -> Gain262/1
  ? -> Gain/1
  Gain374/1 -> Data Type Conversion485/1, IMAPve_d_ORI_R1_ColorClass/1  "IMAPve_d_ORI_R1_ColorClass"
  Gain388/1 -> Data Type Conversion451/1, IMAPve_d_ORI_R0_ColorClass/1
  Gain379/1 -> Data Type Conversion458/1, IMAPve_d_ORI_L1_MeasureType/1  "IMAPve_d_ORI_L1_MeasureType"
  Gain390/1 -> Data Type Conversion449/1, IMAPve_g_ORI_R0_ExistProb/1
  ? -> Gain434/1
  SDFAva_g_obj_pos_var_x/1 -> Gain225/1
  SWINve_y_MP5_DMS_EyeFatigueMonitor/1 -> Gain297/1
  Gain328/1 -> Data Type Conversion354/1, IMAPve_d_EPS_Trq_State/1
  Gain255/1 -> Data Type Conversion169/1, IMAPve_d_ORI_L1_Type/1  "IMAPve_d_ORI_L1_Type"
  Data Type Conversion383/1 -> Terminator379/1  "ob_IMAPve_d_EPB_Warn_Req"
  ? -> Gain388/1
  ? -> Gain385/1
  ? -> Gain386/1
  Data Type Conversion182/1 -> Terminator173/1  "ob_IMAPve_g_ORI_R0_W"
  Data Type Conversion366/1 -> Terminator364/1  "ob_IMAPve_d_TCU_Shift_Valid"
  Gain75/1 -> Data Type Conversion58/1, IMAPve_d_ACU_Passenger_Belt/1
  Data Type Conversion104/1 -> Terminator95/1  "ob_IMAPve_g_ESC_LonAcc"
  Data Type Conversion380/1 -> Terminator376/1  "ob_IMAPve_d_ESC_ACC_Available"
  Gain411/1 -> Data Type Conversion423/1, IMAPva_g_ORI_Obj_Height/1  "IMAPva_g_ORI_Obj_Height"
  Gain93/1 -> Data Type Conversion324/1, IMAPve_d_ESC_EPB_ErrorStatus/1
  Data Type Conversion377/1 -> Terminator373/1  "ob_IMAPve_d_ESC_RR_WhlSpd_Fault"
  Data Type Conversion368/1 -> Terminator366/1  "ob_IMAPve_d_ESC_YawRate_Valid"
  SWINve_y_MP5_DMS_DrinkWaterMonitor/1 -> Gain302/1
  Gain183/1 -> IMAPve_d_LKA_Mode/1, Data Type Conversion35/1
  Gain373/1 -> Data Type Conversion459/1, IMAPve_d_ORI_R1_MeasureType/1  "IMAPve_d_ORI_R1_MeasureType"
  Data Type Conversion125/1 -> Terminator117/1  "ob_IMAPve_g_ESC_RL_WhlSpd"
  Data Type Conversion360/1 -> Terminator358/1  "ob_IMAPve_g_EPS_LKA_Current"
  Data Type Conversion363/1 -> Terminator361/1  "ob_IMAPve_g_EMS_Actual_IndT"
  Data Type Conversion149/1 -> Terminator140/1  "ob_IMAPva_g_ORI_Obj_Width"
  Data Type Conversion342/1 -> Terminator347/1  "ob_IMAPve_d_TBOX_LocalTimeY"
  Gain53/1 -> array_transfer11/1(Trunk_State), Data Type Conversion43/1, IMAPve_d_BCM_Trunk_State/1
  SDFAve_g_L1_C2_COEF/1 -> Gain159/1
  Data Type Conversion138/1 -> Terminator129/1  "ob_IMAPve_g_BCM_Battery_Voltage"
  Data Type Conversion32/1 -> Terminator23/1  "ob_IMAPve_d_BCM_LowBeam_State"
  Data Type Conversion177/1 -> Terminator168/1  "ob_IMAPve_g_ORI_R0_C0"
  Data Type Conversion23/1 -> Terminator14/1  "ob_IMAPve_d_JA_Brake_Switch"
  Data Type Conversion22/1 -> Terminator13/1  "ob_IMAPve_d_DOW_Switch"
  Gain91/1 -> Data Type Conversion322/1, IMAPve_d_ESC_RLW_Direction/1
  ? -> Gain443/1
  Data Type Conversion50/1 -> Terminator41/1  "ob_IMAPve_d_BCM_Left_Light"
  Data Type Conversion3/1 -> Terminator4/1  "ob_IMAPve_d_Speed_Limit"
  Data Type Conversion1/1 -> Terminator2/1  "ob_IMAPve_d_ISA_ISLC_Mode"
  Data Type Conversion21/1 -> Terminator12/1  "ob_IMAPve_d_RCTA_Swtich"
  Data Type Conversion120/1 -> Terminator112/1  "ob_IMAPve_d_ESC_FR_WheelPulVal"
  Gain7/1 -> Data Type Conversion145/1, IMAPva_g_ORI_Obj_LongDis/1  "IMAPva_g_ORI_Obj_LongDis"
  Gain208/1 -> Data Type Conversion408/1, IMAPve_d_BCM_FrontWiper_Switch/1
  Data Type Conversion8/1 -> IMAPve_d_BCM_HazardLamp/1, Data Type Conversion49/1
  Data Type Conversion77/1 -> Terminator68/1  "ob_IMAPve_g_EMS_Pot_WhlT_Min"
  Version/1 -> Terminator1/1  "ob_IMAP_Version"
  Data Type Conversion68/1 -> Terminator59/1  "ob_IMAPve_d_SAS_Trim_State"
  Data Type Conversion206/1 -> Terminator197/1  "ob_IMAPva_d_obj_id"
  Data Type Conversion95/1 -> Terminator86/1  "ob_IMAPve_d_TCU_Target_Gear"
  ? -> Gain436/1
  Data Type Conversion229/1 -> Terminator220/1  "ob_IMAPva_d_obj_BrakeLight"
  Gain50/1 -> Data Type Conversion114/1, IMAPve_d_ESC_MSR_Active/1
  Gain292/1 -> Data Type Conversion417/1, IMAPve_d_MP5_AutoPilot_Switch/1
  Gain309/1 -> Data Type Conversion18/1, IMAPve_d_PEPS_RKE_Command/1
  SDFAve_g_L0_C3_BACK_COEF/1 -> Gain146/1
  Data Type Conversion35/1 -> Terminator25/1  "ob_IMAPve_d_LKA_Mode"
  Data Type Conversion412/1 -> Terminator341/1  "ob_IMAPve_d_MP5_Work_State"
  Data Type Conversion405/1 -> Terminator334/1  "ob_IMAPve_d_ACU_RearRight_Belt"
  Data Type Conversion410/1 -> Terminator339/1  "ob_IMAPve_d_EMS_PowertrainCtl_State"
  Data Type Conversion291/1 -> Terminator282/1  "ob_IMAPve_g_R0_C0_Back"
  Data Type Conversion224/1 -> Terminator215/1  "ob_IMAPva_d_obj_status"
  Data Type Conversion282/1 -> Terminator273/1  "ob_IMAPve_g_L0_C0_Back"
  Gain306/1 -> Data Type Conversion3/1, IMAPve_d_Speed_Limit/1
  Data Type Conversion413/1 -> Terminator342/1  "ob_IMAPve_d_MP5_APA_ModeSelect"
  Data Type Conversion78/1 -> Terminator69/1  "ob_IMAPve_g_EMS_RealPedal"
  Data Type Conversion408/1 -> Terminator337/1  "ob_IMAPve_d_BCM_FrontWiper_Switch"
  Data Type Conversion233/1 -> Terminator224/1  "ob_IMAPve_d_MP5_DMS_Smoking"
  Data Type Conversion415/1 -> Terminator344/1  "ob_IMAPve_d_MP5_UPA_Switch"
  Data Type Conversion404/1 -> Terminator333/1  "ob_IMAPve_d_ACU_RearMiddle_Belt"
  SDFAve_g_ORI_R0_VR/1 -> Gain250/1
  Data Type Conversion324/1 -> Terminator315/1  "ob_IMAPve_d_ESC_EPB_ErrorStatus"
  Gain282/1 -> array_transfer10/1(HazardLamp), Terminator128/1  "ob_IMAP_SWINve_y_BCM_Status_Indicator"
  Data Type Conversion331/1 -> Terminator322/1  "ob_IMAPve_d_ACU_RearLeft_Belt"
  Gain258/1 -> Data Type Conversion172/1, IMAPve_g_ORI_L1_W/1  "IMAPve_g_ORI_L1_W"
  Gain290/1 -> Data Type Conversion134/1, IMAPve_d_EPB_Status/1
  Data Type Conversion327/1 -> Terminator318/1  "ob_IMAPve_d_EPS_Driver_Override"
  Data Type Conversion319/1 -> Terminator310/1  "ob_IMAPve_d_ESC_FLW_Direction"
  SDFAve_g_L0_C0_BACK_COEF/1 -> Gain143/1
  Data Type Conversion226/1 -> Terminator217/1  "ob_IMAPve_d_MP5_DMS_LongtimeDrive"
  SWINve_y_MP5_DMS_UserAccount/1 -> Gain303/1
  Data Type Conversion303/1 -> Terminator294/1  "ob_IMAPve_g_L1_C3_Back"
  SDFAve_y_TSR_Sign_Type/1 -> Gain109/1
  Data Type Conversion231/1 -> Terminator222/1  "ob_IMAPve_d_MP5_DMS_SideView"
  ? -> Gain418/1
  Data Type Conversion320/1 -> Terminator311/1  "ob_IMAPve_d_ESC_FRW_Direction"
  Gain300/1 -> Data Type Conversion232/1, IMAPve_d_MP5_DMS_UsingPhone/1  "IMAPve_d_MP5_DMS_UsingPhone"
  Data Type Conversion482/1 -> Terminator463/1  "ob_IMAPve_d_ORI_R1_ID"
  Data Type Conversion121/1 -> Terminator113/1  "ob_IMAPve_d_ESC_RL_WheelPulVal"
  ? -> Gain396/1
  Data Type Conversion428/1 -> Terminator409/1  "ob_IMAPva_g_ORI_Obj_LAngleStdDev"
  Data Type Conversion369/1 -> Terminator367/1  "ob_IMAPve_d_ESC_LonAcc_Valid"
  Gain301/1 -> Data Type Conversion233/1, IMAPve_d_MP5_DMS_Smoking/1  "IMAPve_d_MP5_DMS_Smoking"
  Gain98/1 -> Data Type Conversion330/1, IMAPve_d_EPS_ESA_State/1
  Gain382/1 -> Data Type Conversion457/1, IMAPve_d_ORI_L1_ColorClass/1  "IMAPve_d_ORI_L1_ColorClass"
  Gain294/1 -> Data Type Conversion217/1, IMAPve_d_MP5_DMS_SystemEnable/1  "IMAPve_d_MP5_DMS_MessageType"
  Gain193/1 -> Data Type Conversion405/1, IMAPve_d_ACU_RearRight_Belt/1
  Data Type Conversion469/1 -> Terminator450/1  "ob_IMAPve_g_ORI_RoadedgeR0_DxStart"
  Gain443/1 -> Data Type Conversion332/1, IMAPva_d_ORI_Obj_TimeStamp/1  "IMAPva_d_ORI_Obj_TimeStamp"
  Data Type Conversion213/1 -> Terminator204/1  "ob_IMAPva_g_obj_pos_var_x"
  Gain194/1 -> Data Type Conversion410/1, IMAPve_d_EMS_PowertrainCtl_State/1
  Gain31/1 -> Data Type Conversion79/1, IMAPve_g_EMS_MaxTWhl/1
  Gain293/1 -> IMAPve_d_MP5_DMS_MessageType/1, Data Type Conversion216/1  "IMAPve_d_MP5_DMS_MessageType"
  Gain94/1 -> Data Type Conversion325/1, IMAPve_d_EPS_SteeringAngle_Flag/1
  Data Type Conversion487/1 -> Terminator468/1  "ob_IMAPve_d_APA_AutoPark_WorkSt"
  Gain210/1 -> Data Type Conversion412/1, IMAPve_d_MP5_Work_State/1
  SWINve_y_MP5_DMS_LongtimeDriveMonitor/1 -> Gain298/1
  SDFAve_g_R0_C2_COEF/1 -> Gain166/1
  SDFAva_d_obj_age/1 -> Gain203/1
  Data Type Conversion443/1 -> Terminator424/1  "ob_IMAPve_g_ORI_L0_ExistProb"
  Data Type Conversion417/1 -> Terminator346/1  "ob_IMAPve_d_MP5_AutoPilot_Switch"
  Data Type Conversion310/1 -> Terminator301/1  "ob_IMAPve_g_R1_C1_Back"
  Gain99/1 -> Data Type Conversion331/1, IMAPve_d_ACU_RearLeft_Belt/1
  Data Type Conversion484/1 -> Terminator465/1  "ob_IMAPve_g_ORI_R1_Dxstart"
  SWINve_y_MP5_DMS_Sensity/1 -> Gain296/1
  Data Type Conversion208/1 -> Terminator199/1  "ob_IMAPva_g_obj_pos_y"
  Data Type Conversion228/1 -> Terminator219/1  "ob_IMAPva_d_obj_TurnLight"
  Data Type Conversion407/1 -> Terminator336/1  "ob_IMAPve_d_BCM_RightTurn_Switch"
  Gain341/1 -> Data Type Conversion385/1, IMAPve_d_EPB_Switch_Valid/1
  Data Type Conversion376/1 -> Terminator372/1  "ob_IMAPve_d_ESC_RL_WhlSpd_Fault"
  Gain158/1 -> Data Type Conversion261/1, IMAPve_g_L1_C1/1  "IMAPve_g_L1_C1"
  Gain339/1 -> Data Type Conversion383/1, IMAPve_d_EPB_Warn_Req/1
  Gain74/1 -> Data Type Conversion377/1, IMAPve_d_ESC_RR_WhlSpd_Fault/1
  SDFAve_g_ORI_L0_C1/1 -> Gain270/1
  Data Type Conversion266/1 -> Terminator257/1  "ob_IMAPve_d_L1_Type"
  Gain344/1 -> Data Type Conversion380/1, IMAPve_d_ESC_ACC_Available/1
  Gain338/1 -> Data Type Conversion382/1, IMAPve_d_EPB_Display_Req/1
  Gain348/1 -> Data Type Conversion370/1, IMAPve_d_ESC_ABS_Valid/1
  Gain346/1 -> Data Type Conversion375/1, IMAPve_d_ESC_FR_WhlSpd_Fault/1
  Gain384/1 -> Data Type Conversion455/1, IMAPve_g_ORI_L1_ExistProb/1  "IMAPve_g_ORI_L1_ExistProb"
  Gain286/1 -> Data Type Conversion376/1, IMAPve_d_ESC_RL_WhlSpd_Fault/1
  ? -> Gain371/1
  ? -> Gain378/1
  Gain23/1 -> Data Type Conversion106/1, IMAPve_g_ESC_Static_Slope/1
  Gain361/1 -> Data Type Conversion470/1, IMAPve_d_ORI_RoadedgeL0_MeasureType/1  "IMAPve_d_ORI_RoadedgeL0_MeasureType"
  Gain326/1 -> Data Type Conversion350/1, IMAPve_d_TBOX_LocalTime_Valid/1
  Gain385/1 -> Data Type Conversion447/1, IMAPve_d_ORI_R0_MeasureType/1  "IMAPve_d_ORI_R0_MeasureType"
  Gain449/1 -> Data Type Conversion6/1, IMAPve_d_ELK_Switch/1
  Gain335/1 -> Data Type Conversion366/1, IMAPve_d_TCU_Shift_Valid/1
  Gain319/1 -> Data Type Conversion138/1, IMAPve_g_BCM_Battery_Voltage/1
  Gain332/1 -> Data Type Conversion363/1, IMAPve_g_EMS_Actual_IndT/1
  Gain352/1 -> Data Type Conversion367/1, IMAPve_d_ESC_LatAcc_Valid/1
  Gain402/1 -> IMAPva_g_ORI_Obj_PhiBottom/1, Data Type Conversion433/1  "IMAPva_g_ORI_Obj_PhiBottom"
  Data Type Conversion311/1 -> Terminator302/1  "ob_IMAPve_g_R1_C2_Back"
  ? -> Gain435/1
  Gain321/1 -> Data Type Conversion343/1, IMAPve_d_TBOX_LocalTimeM/1
  Gain351/1 -> Data Type Conversion368/1, IMAPve_d_ESC_YawRate_Valid/1
  Data Type Conversion255/1 -> Terminator246/1  "ob_IMAPve_d_R0_Type"
  Data Type Conversion313/1 -> Terminator304/1  "ob_IMAPve_g_R1_Range_Back"
  Gain316/1 -> Data Type Conversion30/1, IMAPve_d_PEPS_Door_Lock_Req/1
  Gain360/1 -> Data Type Conversion462/1, IMAPve_g_ORI_RoadedgeL0_C2/1  "IMAPve_g_ORI_RoadedgeL0_C2"
  Data Type Conversion345/1 -> Terminator350/1  "ob_IMAPve_d_TBOX_LocalTimeH"
  Data Type Conversion119/1 -> Terminator106/1  "ob_IMAPve_d_ESC_FL_WheelPulVal"
  Data Type Conversion82/1 -> Terminator73/1  "ob_IMAPve_g_EMS_MinTWhl_Offset"
  Data Type Conversion477/1 -> Terminator458/1  "ob_IMAPve_g_ORI_RoadedgeR0_C3"
  Gain314/1 -> Data Type Conversion23/1, IMAPve_d_JA_Brake_Switch/1
  Gain172/1 -> Data Type Conversion257/1, IMAPve_g_R0_W/1  "IMAPve_g_R0_W"
  ? -> Gain392/1
  Gain21/1 -> Data Type Conversion104/1, IMAPve_g_ESC_LonAcc/1
  Data Type Conversion300/1 -> Terminator291/1  "ob_IMAPve_g_L1_C0_Back"
  ? -> Gain404/1
  Data Type Conversion304/1 -> Terminator295/1  "ob_IMAPve_g_L1_Range_Back"
  Gain323/1 -> Data Type Conversion345/1, IMAPve_d_TBOX_LocalTimeH/1
  Data Type Conversion295/1 -> Terminator286/1  "ob_IMAPve_g_R0_Range_Back"
  SDFAve_d_ORI_CIPV_ID/1 -> Gain1/1
  Gain89/1 -> Data Type Conversion320/1, IMAPve_d_ESC_FRW_Direction/1
  Gain291/1 -> Data Type Conversion416/1, IMAPve_d_MP5_FLK_Activation/1
  Gain342/1 -> Data Type Conversion378/1, IMAPve_d_ESC_AEB_Available/1
  Data Type Conversion394/1 -> Terminator390/1  "ob_IMAPva_g_ORI_Obj_RelVely"
  Data Type Conversion44/1 -> Terminator35/1  "ob_IMAPve_d_BCM_LF_Door_State"
  SDFAve_g_L1_C1_COEF/1 -> Gain158/1
  Data Type Conversion127/1 -> Terminator119/1  "ob_IMAPve_d_ESC_FL_Wheel_Pulse"
  Data Type Conversion285/1 -> Terminator276/1  "ob_IMAPve_g_L0_C3_Back"
  Gain307/1 -> Data Type Conversion4/1, IMAPve_d_ALC_TLC_Mode/1
  SDFAve_g_R0_C0_COEF/1 -> Gain191/1
  Gain95/1 -> Data Type Conversion326/1, IMAPve_g_EPS_SteeringAngle/1
  Data Type Conversion261/1 -> Terminator252/1  "ob_IMAPve_g_L1_C1"
  Data Type Conversion155/1 -> Terminator146/1  "ob_IMAPve_g_ORI_L0_C2"
  Gain179/1 -> Data Type Conversion246/1, IMAPve_g_L0_W/1  "IMAPve_g_L0_W"
  Data Type Conversion254/1 -> Terminator245/1  "ob_IMAPve_d_R0_Q"
  Data Type Conversion154/1 -> Terminator145/1  "ob_IMAPve_g_ORI_L0_C3"
  Gain308/1 -> Data Type Conversion5/1, IMAPve_d_ESA_Switch/1
  Data Type Conversion257/1 -> Terminator248/1  "ob_IMAPve_g_R0_W"
  Gain267/1 -> Data Type Conversion167/1, IMAPve_g_ORI_L1_C0/1  "IMAPve_g_ORI_L1_C0"
  Data Type Conversion209/1 -> Terminator200/1  "ob_IMAPva_g_obj_vel_x"
  Data Type Conversion241/1 -> Terminator232/1  "ob_IMAPve_g_L0_C3"
  Data Type Conversion172/1 -> Terminator163/1  "ob_IMAPve_g_ORI_L1_W"
  Data Type Conversion111/1 -> Terminator103/1  "ob_IMAPve_d_ESC_OFF"
  SDFAva_y_obj_lane/1 -> Gain217/1
  ? -> Gain252/1
  Data Type Conversion215/1 -> Terminator206/1  "ob_IMAPva_g_obj_pos_var_xy"
  Data Type Conversion242/1 -> Terminator233/1  "ob_IMAPve_g_L0_VR"
  Data Type Conversion227/1 -> Terminator218/1  "ob_IMAPva_d_obj_age"
  ? -> Gain376/1
  Data Type Conversion239/1 -> Terminator230/1  "ob_IMAPve_g_L0_C1"
  Data Type Conversion397/1 -> Terminator393/1  "ob_IMAPva_g_ORI_Obj_AbsAyStdDev"
  Data Type Conversion230/1 -> Terminator221/1  "ob_IMAPva_d_obj_MotionStatus"
  Gain96/1 -> Data Type Conversion327/1, IMAPve_d_EPS_Driver_Override/1
  ? -> Gain419/1
  Data Type Conversion49/1 -> Terminator40/1  "ob_IMAPve_d_BCM_HazardLamp"
  SDFAva_g_ORI_Obj_LongDis/1 -> Gain7/1
  Data Type Conversion276/1 -> Terminator267/1  "ob_IMAPve_d_R1_Q"
  Data Type Conversion109/1 -> Terminator100/1  "ob_IMAPve_d_ESC_Brake_Effort"
  Data Type Conversion205/1 -> Terminator196/1  "ob_IMAPve_d_obj_Num"
  Data Type Conversion218/1 -> Terminator209/1  "ob_IMAPve_d_MP5_DMS_DelUserNum"
  Gain152/1 -> Data Type Conversion273/1, IMAPve_g_R1_C2/1  "IMAPve_g_R1_C2"
  Gain1/1 -> Data Type Conversion139/1, IMAPve_d_ORI_CIPV_ID/1  "IMAPve_d_ORI_CIPV_ID"
  Gain387/1 -> Data Type Conversion450/1, IMAPve_g_ORI_R0_Dxstart/1
  SDFAve_g_L1_C3_COEF/1 -> Gain160/1
  Data Type Conversion150/1 -> Terminator141/1  "ob_IMAPva_d_ORI_Obj_ID"
  Data Type Conversion192/1 -> Terminator183/1  "ob_IMAPve_g_ORI_R1_W"
  Data Type Conversion274/1 -> Terminator265/1  "ob_IMAPve_g_R1_C3"
  Data Type Conversion164/1 -> Terminator155/1  "ob_IMAPve_g_ORI_L1_C3"
  Data Type Conversion179/1 -> Terminator170/1  "ob_IMAPve_d_ORI_R0_LT"
  Data Type Conversion240/1 -> Terminator231/1  "ob_IMAPve_g_L0_C2"
  Gain422/1 -> Data Type Conversion400/1, IMAPva_g_ORI_Obj_LongDisStdDev/1  "IMAPva_g_ORI_Obj_LongDisStdDev"
  Data Type Conversion180/1 -> Terminator171/1  "ob_IMAPve_g_ORI_R0_VR"
  Gain410/1 -> Data Type Conversion432/1, IMAPva_g_ORI_Obj_AngleRateStdDev/1  "IMAPva_g_ORI_Obj_AngleRateStdDev"
  Gain59/1 -> Data Type Conversion123/1, IMAPve_g_ESC_FL_WhlSpd/1
  Data Type Conversion190/1 -> Terminator181/1  "ob_IMAPve_g_ORI_R1_VR"
  Data Type Conversion338/1 -> Terminator329/1  "ob_IMAPve_d_ORI_FS_LowSun0"
  Data Type Conversion176/1 -> Terminator167/1  "ob_IMAPve_g_ORI_R0_C1"
  Gain78/1 -> Data Type Conversion54/1, IMAPve_d_BCM_FrontWiper_State/1
  Data Type Conversion75/1 -> Terminator66/1  "ob_IMAPve_d_EMS_ACC_Status"
  Gain356/1 -> Data Type Conversion466/1, IMAPve_g_ORI_RoadedgeL0_C1/1  "IMAPve_g_ORI_RoadedgeL0_C1"
  Gain303/1 -> Data Type Conversion318/1, IMAPve_d_MP5_DMS_UserAccount/1  "IMAPve_d_MP5_DMS_UserAccount"
  Data Type Conversion216/1 -> Terminator207/1  "ob_IMAPve_d_MP5_DMS_MessageType"
  Data Type Conversion116/1 -> Terminator108/1  "ob_IMAPve_d_ESC_VehSpd_Valid"
  Data Type Conversion76/1 -> Terminator67/1  "ob_IMAPve_g_EMS_Pot_WhlT_Max"
  Data Type Conversion130/1 -> Terminator122/1  "ob_IMAPve_d_ESC_RR_Wheel_Pulse"
  Data Type Conversion354/1 -> Terminator357/1  "ob_IMAPve_d_EPS_Trq_State"
  Gain134/1 -> Data Type Conversion291/1, IMAPve_g_R0_C0_Back/1  "IMAPve_g_R0_C0_Back"
  SDFAva_g_ORI_Obj_AbsAx/1 -> Gain433/1
  Data Type Conversion105/1 -> Terminator96/1  "ob_IMAPve_g_ESC_Brake_Press"
  Data Type Conversion139/1 -> Terminator130/1  "ob_IMAPve_d_ORI_CIPV_ID"
  Data Type Conversion80/1 -> Terminator71/1  "ob_IMAPve_g_EMS_MaxTWhl_Offset"
  Data Type Conversion108/1 -> Terminator99/1  "ob_IMAPve_g_ESC_DySlope"
  Data Type Conversion279/1 -> Terminator270/1  "ob_IMAPve_g_R1_W"
  Gain170/1 -> Data Type Conversion255/1, IMAPve_d_R0_Type/1  "IMAPve_d_R0_Type"
  Data Type Conversion94/1 -> Terminator85/1  "ob_IMAPve_d_EMS_Brake_Pedal"
  Data Type Conversion449/1 -> Terminator430/1  "ob_IMAPve_g_ORI_R0_ExistProb"
  Data Type Conversion114/1 -> Terminator101/1  "ob_IMAPve_d_ESC_MSR_Active"
  Gain175/1 -> Data Type Conversion242/1, IMAPve_g_L0_VR/1  "IMAPve_g_L0_VR"
  Gain311/1 -> Data Type Conversion20/1, IMAPve_d_FCTA_Switch/1
  Data Type Conversion169/1 -> Terminator160/1  "ob_IMAPve_d_ORI_L1_Type"
  Gain79/1 -> Data Type Conversion55/1, IMAPve_d_BCM_CHMSL_Status/1
  Data Type Conversion53/1 -> Terminator44/1  "ob_IMAPve_d_ACU_Driver_Belt"
  Data Type Conversion92/1 -> Terminator83/1  "ob_IMAPve_d_EMS_ACC_CtlAvail"
  Gain83/1 -> Data Type Conversion94/1, IMAPve_d_EMS_Brake_Pedal/1
  Data Type Conversion54/1 -> Terminator45/1  "ob_IMAPve_d_BCM_FrontWiper_State"
  SWINve_y_MP5_DMS_SystemEnable/1 -> Gain294/1
  Gain349/1 -> Data Type Conversion371/1, IMAPve_d_ESC_ABS_AlarmSig/1
  Gain24/1 -> Data Type Conversion71/1, IMAPve_g_SW_Angle_Speed/1
  SDFAva_d_ORI_Obj_Class/1 -> Gain4/1
  Gain43/1 -> Data Type Conversion73/1, IMAPve_d_SWS_Failure_Status/1
  Gain353/1 -> array_transfer11/5(LR_Door), Data Type Conversion47/1, IMAPve_d_BCM_LR_Door_State/1
  Data Type Conversion91/1 -> Terminator82/1  "ob_IMAPve_d_EMS_ACC_Effective"
  Data Type Conversion48/1 -> Terminator39/1  "ob_IMAPve_d_SCC_Left_SwitchSig"
  Data Type Conversion73/1 -> Terminator64/1  "ob_IMAPve_d_SWS_Failure_Status"
  Data Type Conversion89/1 -> Terminator80/1  "ob_IMAPve_d_EMS_Engine_Status"
  Data Type Conversion90/1 -> Terminator81/1  "ob_IMAPve_d_EMS_Gearbox_CtlAvail"
  Switch/1 -> Gain3/1  "IMAPve_d_LKA_Main_Switch"
  Data Type Conversion65/1 -> Terminator56/1  "ob_IMAPve_g_EPS_SW_Trq"
  Data Type Conversion62/1 -> Terminator53/1  "ob_IMAPve_g_GW_IC_Odometer"
  SDFAve_d_ORI_R0_LT/1 -> Gain249/1
  Data Type Conversion134/1 -> Terminator121/1  "ob_IMAPve_d_EPB_Status"
  ? -> Gain405/1
  Gain392/1 -> Data Type Conversion439/1, IMAPva_g_ORI_Obj_TTIPC/1  "IMAPva_g_ORI_Obj_TTIPC"
  SDFAva_g_ORI_Obj_LateralDis/1 -> Gain427/1
  Data Type Conversion58/1 -> Terminator49/1  "ob_IMAPve_d_ACU_Passenger_Belt"
  Data Type Conversion346/1 -> Terminator351/1  "ob_IMAPve_d_TBOX_LocalTimeMin"
  Data Type Conversion52/1 -> Terminator43/1  "ob_IMAPve_d_BCM_Ignition_State"
  Gain260/1 -> IMAPve_g_ORI_R0_C3/1, Data Type Conversion174/1  "ob_IMAPve_g_ORI_R0_C3"
  Data Type Conversion110/1 -> Terminator102/1  "ob_IMAPve_d_ESC_Veh_Standstill"
  Data Type Conversion59/1 -> Terminator50/1  "ob_IMAPve_d_SCC_Right_SwitchSig"
  Data Type Conversion45/1 -> Terminator36/1  "ob_IMAPve_d_BCM_RF_Door_State"
  Data Type Conversion411/1 -> Terminator340/1  "ob_IMAPve_d_TCU_TCU_Available"
  Data Type Conversion51/1 -> Terminator42/1  "ob_IMAPve_d_BCM_Right_Light"
  Gain345/1 -> Data Type Conversion381/1, IMAPve_d_ESC_ACC_Active/1
  Data Type Conversion46/1 -> Terminator37/1  "ob_IMAPve_d_BCM_RR_Door_State"
  Gain337/1 -> Data Type Conversion387/1, IMAPve_d_ESC_AVH_Status/1
  Gain324/1 -> Data Type Conversion346/1, IMAPve_d_TBOX_LocalTimeMin/1
  Gain279/1 -> array_transfer11/3(RF_Door), Data Type Conversion45/1, IMAPve_d_BCM_RF_Door_State/1
  Data Type Conversion40/1 -> Terminator31/1  "ob_IMAPve_d_TSR_Switch"
  SDFAve_g_R1_C3_COEF/1 -> Gain153/1
  SDFAve_g_R0_C1_BACK_COEF/1 -> Gain135/1
  Data Type Conversion47/1 -> Terminator38/1  "ob_IMAPve_d_BCM_LR_Door_State"
  Gain66/1 -> Data Type Conversion130/1, IMAPve_d_ESC_RR_Wheel_Pulse/1
  Gain188/1 -> IMAPve_d_TSR_Switch/1, Data Type Conversion40/1
  Data Type Conversion6/1 -> Terminator7/1  "ob_IMAPve_d_ELK_Switch"
  Gain278/1 -> Data Type Conversion78/1, IMAPve_g_EMS_RealPedal/1
  Data Type Conversion34/1 -> Terminator24/1  "ob_IMAPve_d_LKA_Main_Switch"
  Gain285/1 -> Data Type Conversion85/1, IMAPve_g_EMS_ACC_VirtualPedal/1
  Gain283/1 -> Data Type Conversion83/1, IMAPve_g_EMS_Actual_FlwT/1
  Data Type Conversion30/1 -> Terminator21/1  "ob_IMAPve_d_PEPS_Door_Lock_Req"
  ? -> Gain9/1
  array_transfer11/1(output) -> Data Type Conversion/1
  Data Type Conversion29/1 -> Terminator20/1  "ob_IMAPve_d_ESC_BrakeLamp_Req"
  Gain201/1 -> Data Type Conversion411/1, IMAPve_d_TCU_TCU_Available/1
  Gain266/1 -> Data Type Conversion166/1, IMAPve_g_ORI_L1_C1/1  "IMAPve_g_ORI_L1_C1"
  ? -> Gain399/1
  Gain97/1 -> Data Type Conversion328/1, IMAPve_d_EPS_Driver_Active_ESA/1
  Gain412/1 -> Data Type Conversion424/1, IMAPva_g_ORI_Obj_LengthStdDev/1  "IMAPva_g_ORI_Obj_LengthStdDev"
  Gain274/1 -> IMAPve_g_ORI_L0_VR/1, Data Type Conversion160/1  "IMAPve_g_ORI_L0_VR"
  Gain273/1 -> Data Type Conversion159/1, IMAPve_d_ORI_L0_Type/1  "IMAPve_d_ORI_L0_Type"
  Gain377/1 -> Data Type Conversion481/1, IMAPve_g_ORI_L1_TypeConf/1  "IMAPve_g_ORI_L1_TypeConf"
  Data Type Conversion200/1 -> Terminator191/1  "ob_IMAPve_d_Sign_ISA_Value"
  Gain209/1 -> Data Type Conversion409/1, IMAPve_d_BCM_IHBC_Enabled/1
  Data Type Conversion39/1 -> Terminator30/1  "ob_IMAPve_d_ISA_Switch"
  SDFAve_g_ORI_L0_C0/1 -> Gain271/1
  Gain271/1 -> IMAPve_g_ORI_L0_C0/1, Data Type Conversion157/1  "IMAPve_g_ORI_L0_C0"
  Gain281/1 -> Data Type Conversion70/1, IMAPve_g_SW_Angle/1
  Data Type Conversion293/1 -> Terminator284/1  "ob_IMAPve_g_R0_C2_Back"
  Data Type Conversion106/1 -> Terminator97/1  "ob_IMAPve_g_ESC_Static_Slope"
  Gain252/1 -> IMAPve_g_ORI_R0_W/1, Data Type Conversion182/1  "ob_IMAPve_g_ORI_R0_W"
  SDFAve_d_ORI_L0_Type/1 -> Gain273/1
  Data Type Conversion219/1 -> Terminator210/1  "ob_IMAPva_g_obj_width"
  SDFAve_g_ORI_L0_C2/1 -> Gain269/1
  Gain28/1 -> Data Type Conversion59/1, IMAPve_d_SCC_Right_SwitchSig/1
  Gain76/1 -> array_transfer11/2(LF_Door), Data Type Conversion44/1, IMAPve_d_BCM_LF_Door_State/1
  Gain242/1 -> IMAPve_g_ORI_R1_VR/1, Data Type Conversion190/1  "ob_IMAPve_g_ORI_R1_VR"
  Gain192/1 -> Data Type Conversion404/1, IMAPve_d_ACU_RearMiddle_Belt/1
  Gain49/1 -> Data Type Conversion113/1, IMAPve_d_ESC_ESC_Active/1
  Data Type Conversion36/1 -> Terminator27/1  "ob_IMAPve_d_AEB_Switch"
  Data Type Conversion349/1 -> Terminator352/1  "ob_IMAPve_d_TBOX_LocalTimeS"
  SDFAve_g_ORI_L1_C2/1 -> Gain265/1
  Gain264/1 -> IMAPve_g_ORI_L1_C3/1, Data Type Conversion164/1  "ob_IMAPve_g_ORI_L1_C3"
  Data Type Conversion389/1 -> Terminator385/1  "ob_IMAPve_d_ORI_FS_FrozenWindshield0"
  SDFAve_g_ORI_L1_C0/1 -> Gain267/1
  Data Type Conversion174/1 -> Terminator165/1  "ob_IMAPve_g_ORI_R0_C3"
  Gain244/1 -> Data Type Conversion192/1, IMAPve_g_ORI_R1_W/1  "IMAPve_g_ORI_R1_W"
  Gain239/1 -> Data Type Conversion187/1, IMAPve_g_ORI_R1_C0/1  "IMAPve_g_ORI_R1_C0"
  Data Type Conversion225/1 -> Terminator216/1  "ob_IMAPve_d_MP5_DMS_EyeFatigue"
  Gain247/1 -> Data Type Conversion177/1, IMAPve_g_ORI_R0_C0/1  "IMAPve_g_ORI_R0_C0"
  Data Type Conversion201/1 -> Terminator192/1  "ob_IMAPve_d_TSR_Sign_Type"
  Data Type Conversion96/1 -> Terminator87/1  "ob_IMAPve_d_TCU_AT_Failure"
  Data Type Conversion142/1 -> Terminator133/1  "ob_IMAPva_d_ORI_Obj_Class"
  Data Type Conversion481/1 -> Terminator462/1  "ob_IMAPve_g_ORI_L1_TypeConf"
  Gain305/1 -> Data Type Conversion2/1, IMAPve_d_LDW_Warn_Mode/1
  Gain256/1 -> Data Type Conversion170/1, IMAPve_g_ORI_L1_VR/1  "IMAPve_g_ORI_L1_VR"
  Gain232/1 -> Data Type Conversion197/1, IMAPve_d_RR_Radar_Status/1  "IMAPve_d_RR_Radar_Status"
  Gain261/1 -> Data Type Conversion175/1, IMAPve_g_ORI_R0_C2/1  "IMAPve_g_ORI_R0_C2"
  Gain249/1 -> Data Type Conversion179/1, IMAPve_d_ORI_R0_LT/1  "IMAPve_d_ORI_R0_LT"
  Data Type Conversion442/1 -> Terminator423/1  "ob_IMAPve_d_ORI_L0_ID"
  Gain138/1 -> Data Type Conversion277/1, IMAPve_d_R1_Type/1  "IMAPve_d_R1_Type"
  SDFAve_g_ORI_R0_C1/1 -> Gain246/1
  Gain358/1 -> Data Type Conversion461/1, IMAPve_d_ORI_RoadedgeL0_ID/1  "IMAPve_d_ORI_RoadedgeL0_ID"
  Gain357/1 -> Data Type Conversion467/1, IMAPve_g_ORI_RoadedgeL0_C0/1  "IMAPve_g_ORI_RoadedgeL0_C0"
  ? -> Gain244/1
  SDFAve_g_ORI_R0_C0/1 -> Gain247/1
  SDFAve_g_ORI_R0_C2/1 -> Gain261/1
  Gain241/1 -> Data Type Conversion189/1, IMAPve_d_ORI_R1_LT/1  "IMAPve_d_ORI_R1_LT"
  SDFAve_g_ORI_R0_C3/1 -> Gain260/1
  SDFAve_g_ORI_R1_C2/1 -> Gain237/1
  Gain221/1 -> Data Type Conversion209/1, IMAPva_g_obj_vel_x/1  "IMAPva_g_obj_vel_x"
  SDFAva_y_obj_id/1 -> Gain236/1
  Gain228/1 -> Data Type Conversion193/1, IMAPve_d_Sensor_Status/1  "IMAPve_d_Sensor_Status"
  Gain359/1 -> Data Type Conversion468/1, IMAPve_g_ORI_RoadedgeL0_C3/1  "IMAPve_g_ORI_RoadedgeL0_C3"
  SDFAva_g_obj_pos_var_xy/1 -> Gain227/1
  Data Type Conversion162/1 -> Terminator153/1  "ob_IMAPve_g_ORI_L0_W"
  ? -> Gain411/1
  SDFAve_g_ORI_L1_VR/1 -> Gain256/1
  Gain393/1 -> Data Type Conversion440/1, IMAPva_d_ORI_Obj_DirectionIndicator/1  "IMAPva_d_ORI_Obj_DirectionIndicator"
  Data Type Conversion222/1 -> Terminator213/1  "ob_IMAPva_d_obj_class"
  Gain231/1 -> Data Type Conversion196/1, IMAPve_d_LR_Radar_Status/1  "IMAPve_d_LR_Radar_Status"
  SWINve_y_MP5_DMS_MessageType/1 -> Gain293/1
  Data Type Conversion232/1 -> Terminator223/1  "ob_IMAPve_d_MP5_DMS_UsingPhone"
  SDFAve_d_sensor_status/1 -> Gain228/1
  ? -> Gain416/1
  Data Type Conversion86/1 -> Terminator77/1  "ob_IMAPve_g_EMS_Driver_Torque"
  Gain15/1 -> Data Type Conversion67/1, IMAPve_d_SAS_Clb_State/1
  SDFAve_g_R0_BACK_RANGE/1 -> Gain125/1
  Data Type Conversion438/1 -> Terminator419/1  "ob_IMAPva_d_ORI_Obj_HeadOrientation"
  Gain220/1 -> Data Type Conversion208/1, IMAPva_g_obj_pos_y/1  "IMAPva_g_obj_pos_y"
  Data Type Conversion252/1 -> Terminator243/1  "ob_IMAPve_g_R0_C3"
  Gain322/1 -> Data Type Conversion344/1, IMAPve_d_TBOX_LocalTimeD/1
  Data Type Conversion135/1 -> Terminator126/1  "ob_IMAPve_d_ESC_Drive_Direction"
  ? -> Gain380/1
  Gain47/1 -> Data Type Conversion112/1, IMAPve_d_ESC_AlarmSig/1
  Gain119/1 -> Data Type Conversion300/1, IMAPve_g_L1_C0_Back/1  "IMAPve_g_L1_C0_Back"
  SDFAve_y_ISAValue/1 -> Gain108/1
  Gain227/1 -> Data Type Conversion215/1, IMAPva_g_obj_pos_var_xy/1  "IMAPva_g_obj_pos_var_xy"
  Gain219/1 -> Data Type Conversion207/1, IMAPva_g_obj_pos_x/1  "IMAPva_g_obj_pos_x"
  Gain315/1 -> Data Type Conversion29/1, IMAPve_d_ESC_BrakeLamp_Req/1
  Gain225/1 -> Data Type Conversion213/1, IMAPva_g_obj_pos_var_x/1  "IMAPva_g_obj_pos_var_x"
  Gain51/1 -> Data Type Conversion115/1, IMAPve_d_ESC_TCS_Active/1
  Gain399/1 -> Data Type Conversion427/1, IMAPva_g_ORI_Obj_3DAngle/1  "IMAPva_g_ORI_Obj_3DAngle"
  SDFAva_y_obj_TurnLight/1 -> Gain204/1
  SDFAve_g_R1_C0_BACK_COEF/1 -> Gain111/1
  SDFAve_g_R1_MARK_WIDTH/1 -> Gain140/1
  Gain205/1 -> Data Type Conversion229/1, IMAPva_d_obj_BrakeLight/1  "IMAPva_d_obj_BrakeLight"
  SDFAve_g_L0_C2_COEF/1 -> Gain200/1
  SDFAve_d_obj_Num/1 -> Gain235/1
  Gain343/1 -> Data Type Conversion379/1, IMAPve_d_ESC_AEB_Active/1
  SDFAve_g_L0_C0_COEF/1 -> Gain198/1
  Gain403/1 -> Data Type Conversion434/1, IMAPva_g_ORI_Obj_PhiBottomStdDev/1  "IMAPva_g_ORI_Obj_PhiBottomStdDev"
  SDFAva_g_obj_pos_x/1 -> Gain219/1
  Data Type Conversion246/1 -> Terminator237/1  "ob_IMAPve_g_L0_W"
  Data Type Conversion264/1 -> Terminator255/1  "ob_IMAPve_g_L1_VR"
  Data Type Conversion31/1 -> Terminator22/1  "ob_IMAPve_d_BCM_Door_Lock_State"
  SDFAve_d_L0_LINE_TYPE/1 -> Gain177/1
  Gain235/1 -> Data Type Conversion205/1, IMAPve_d_obj_Num/1  "IMAPve_d_obj_Num"
  Data Type Conversion440/1 -> Terminator421/1  "ob_IMAPva_d_ORI_Obj_DirectionIndicator"
  Gain417/1 -> Data Type Conversion420/1, IMAPva_d_ORI_Obj_RelVelyStdDevValid/1  "IMAPva_d_ORI_Obj_RelVelyStdDevValid"
  SDFAve_y_L0_DETECT_QUALITY/1 -> Gain176/1
  Data Type Conversion260/1 -> Terminator251/1  "ob_IMAPve_g_L1_C0"
  SDFAve_g_L0_MARK_WIDTH/1 -> Gain179/1
  SDFAve_y_ROAD_TYPE/1 -> Gain196/1
  Data Type Conversion212/1 -> Terminator203/1  "ob_IMAPva_g_obj_acc_y"
  Gain167/1 -> Data Type Conversion252/1, IMAPve_g_R0_C3/1  "IMAPve_g_R0_C3"
  Gain217/1 -> Data Type Conversion223/1, IMAPva_d_obj_lane/1  "IMAPva_d_obj_lane"
  Gain212/1 -> Data Type Conversion414/1, IMAPve_d_MP5_LanguageSet/1
  Data Type Conversion251/1 -> Terminator242/1  "ob_IMAPve_g_R0_C2"
  SDFAve_g_L0_C3_COEF/1 -> Gain174/1
  SDFAve_g_R0_C1_COEF/1 -> Gain165/1
  Gain354/1 -> Data Type Conversion464/1, IMAPve_g_ORI_RoadedgeL0_DxStart/1  "IMAPve_g_ORI_RoadedgeL0_DxStart"
  SDFAve_g_R0_VIEW_RANGE/1 -> Gain168/1
  Data Type Conversion401/1 -> Terminator397/1  "ob_IMAPva_g_ORI_Obj_LateralDisStdDev"
  SDFAva_g_obj_acc_y/1 -> Gain224/1
  Gain168/1 -> Data Type Conversion253/1, IMAPve_g_R0_VR/1  "IMAPve_g_R0_VR"
  Data Type Conversion426/1 -> Terminator407/1  "ob_IMAPva_g_ORI_Obj_HeightStdDev"
  Data Type Conversion/1 -> Data Type Conversion42/1, IMAPve_d_BCM_Opening_State/1
  Gain169/1 -> Data Type Conversion254/1, IMAPve_d_R0_Q/1  "IMAPve_d_R0_Q"
  SDFAva_g_ORI_Obj_RelVel/1 -> Gain6/1
  SDFAve_g_L1_C0_COEF/1 -> Gain157/1
  Data Type Conversion420/1 -> Terminator401/1  "ob_IMAPva_d_ORI_Obj_RelVelyStdDevValid"
  Gain191/1 -> Data Type Conversion249/1, IMAPve_g_R0_C0/1  "IMAPve_g_R0_C0"
  Gain85/1 -> Data Type Conversion60/1, IMAPve_d_BCM_HighBeam_State/1
  SDFAve_d_L1_LINE_TYPE/1 -> Gain163/1
  Gain334/1 -> Data Type Conversion365/1, IMAPve_d_TCU_PRND_State/1
  Gain336/1 -> Data Type Conversion386/1, IMAPve_d_ESC_EBD_AlarmSig/1
  SDFAve_g_R0_C0_BACK_COEF/1 -> Gain134/1
  Gain160/1 -> Data Type Conversion263/1, IMAPve_g_L1_C3/1  "IMAPve_g_L1_C3"
  SDFAve_g_R1_C1_COEF/1 -> Gain151/1
  Data Type Conversion100/1 -> Terminator91/1  "ob_IMAPve_g_ESC_LatAcc"
  Data Type Conversion390/1 -> Terminator386/1  "ob_IMAPve_d_ORI_FS_OutOfFocus0"
  SDFAve_y_L1_DETECT_QUALITY/1 -> Gain162/1
  SDFAve_y_R1_DETECT_QUALITY/1 -> Gain155/1
  SDFAve_d_R0_LINE_TYPE/1 -> Gain170/1
  Data Type Conversion195/1 -> Terminator186/1  "ob_IMAPve_d_RF_Radar_Status"
  SDFAve_g_L1_C1_BACK_COEF/1 -> Gain124/1
  Gain162/1 -> Data Type Conversion265/1, IMAPve_d_L1_Q/1  "IMAPve_d_L1_Q"
  Data Type Conversion220/1 -> Terminator211/1  "ob_IMAPva_g_obj_length"
  Gain202/1 -> Data Type Conversion406/1, IMAPve_d_BCM_LeftTurn_Switch/1
  ? -> Gain425/1
  SDFAve_g_L1_MARK_WIDTH/1 -> Gain147/1
  Data Type Conversion185/1 -> Terminator176/1  "ob_IMAPve_g_ORI_R1_C2"
  Gain199/1 -> Data Type Conversion239/1, IMAPve_g_L0_C1/1  "IMAPve_g_L0_C1"
  Data Type Conversion268/1 -> Terminator259/1  "ob_IMAPve_g_L1_W"
  SDFAve_g_ORI_L1_C3/1 -> Gain264/1
  SDFAve_g_ORI_R1_C1/1 -> Gain238/1
  Data Type Conversion243/1 -> Terminator234/1  "ob_IMAPve_d_L0_Q"
  Data Type Conversion328/1 -> Terminator319/1  "ob_IMAPve_d_EPS_Driver_Active_ESA"
  Data Type Conversion321/1 -> Terminator312/1  "ob_IMAPve_d_ESC_TCS_ErrorStatus"
  Gain196/1 -> Data Type Conversion236/1, IMAPve_d_Road_Type/1  "IMAPve_d_Road_Type"
  Data Type Conversion124/1 -> Terminator111/1  "ob_IMAPve_g_ESC_FR_WhlSpd"
  Gain19/1 -> Data Type Conversion102/1, IMAPve_g_ESC_UnYawRate/1
  Gain347/1 -> Data Type Conversion374/1, IMAPve_d_ESC_FL_WhlSpd_Fault/1
  Gain207/1 -> Data Type Conversion407/1, IMAPve_d_BCM_RightTurn_Switch/1
  ? -> Gain407/1
  Gain150/1 -> Data Type Conversion271/1, IMAPve_g_R1_C0/1  "IMAPve_g_R1_C0"
  Data Type Conversion123/1 -> Terminator115/1  "ob_IMAPve_g_ESC_FL_WhlSpd"
  Data Type Conversion193/1 -> Terminator184/1  "ob_IMAPve_d_Sensor_Status"
  Gain425/1 -> Data Type Conversion397/1, IMAPva_g_ORI_Obj_AbsAyStdDev/1  "IMAPva_g_ORI_Obj_AbsAyStdDev"
  Gain154/1 -> Data Type Conversion275/1, IMAPve_g_R1_VR/1  "IMAPve_g_R1_VR"
  Data Type Conversion236/1 -> Terminator227/1  "ob_IMAPve_d_Road_Type"
  Data Type Conversion19/1 -> Terminator10/1  "ob_IMAPve_d_BSD_LCW_Switch"
  Gain147/1 -> Data Type Conversion268/1, IMAPve_g_L1_W/1  "IMAPve_g_L1_W"
  SDFAva_d_obj_status/1 -> Gain218/1
  Gain151/1 -> Data Type Conversion272/1, IMAPve_g_R1_C1/1  "IMAPve_g_R1_C1"
  Data Type Conversion439/1 -> Terminator420/1  "ob_IMAPva_g_ORI_Obj_TTIPC"
  Data Type Conversion326/1 -> Terminator317/1  "ob_IMAPve_g_EPS_SteeringAngle"
  SDFAve_g_ORI_R1_C3/1 -> Gain254/1
  Data Type Conversion277/1 -> Terminator268/1  "ob_IMAPve_d_R1_Type"
  Gain380/1 -> Data Type Conversion453/1, IMAPve_g_ORI_R0_TypeConf/1  "IMAPve_g_ORI_R0_TypeConf"
  Data Type Conversion197/1 -> Terminator188/1  "ob_IMAPve_d_RR_Radar_Status"
  Gain190/1 -> Data Type Conversion65/1, IMAPve_g_EPS_SW_Trq/1
  SDFAve_g_R1_VIEW_RANGE/1 -> Gain154/1
  Gain213/1 -> Data Type Conversion219/1, IMAPva_g_obj_width/1  "IMAPva_g_obj_width"
  Gain140/1 -> Data Type Conversion279/1, IMAPve_g_R1_W/1  "IMAPve_g_R1_W"
  Gain398/1 -> IMAPve_d_ORI_L0_ColorClass/1, Data Type Conversion445/1  "IMAPve_d_ORI_L0_ColorClass"
  SDFAve_g_R0_C2_BACK_COEF/1 -> Gain136/1
  Data Type Conversion323/1 -> Terminator314/1  "ob_IMAPve_d_ESC_RRW_Direction"
  Gain298/1 -> Data Type Conversion226/1, IMAPve_d_MP5_DMS_LongtimeDrive/1  "IMAPve_d_MP5_DMS_LongtimeDrive"
  SDFAve_d_fusion_time_stamp/1 -> Gain234/1
  SDFAva_g_obj_vel_y/1 -> Gain222/1
  SDFAve_g_L0_C1_BACK_COEF/1 -> Gain144/1
  Data Type Conversion118/1 -> Terminator110/1  "ob_IMAPve_d_ESC_ABS_Active"
  Gain327/1 -> Data Type Conversion353/1, IMAPve_d_Outside_Temp/1
  Gain350/1 -> Data Type Conversion369/1, IMAPve_d_ESC_LonAcc_Valid/1
  Gain340/1 -> Data Type Conversion384/1, IMAPve_d_EPB_Switch_State/1
  Data Type Conversion101/1 -> Terminator92/1  "ob_IMAPve_g_ESC_YawRate"
  Data Type Conversion97/1 -> Terminator88/1  "ob_IMAPve_d_TCU_DCT_Clutch_State"
  Gain176/1 -> Data Type Conversion243/1, IMAPve_d_L0_Q/1  "IMAPve_d_L0_Q"
  Data Type Conversion262/1 -> Terminator253/1  "ob_IMAPve_g_L1_C2"
  SDFAve_d_R1_LINE_TYPE/1 -> Gain138/1
  Data Type Conversion64/1 -> Terminator55/1  "ob_IMAPve_d_EPS_LKA_State"
  Data Type Conversion451/1 -> Terminator432/1  "ob_IMAPve_d_ORI_R0_ColorClass"
  Gain299/1 -> Data Type Conversion231/1, IMAPve_d_MP5_DMS_SideView/1  "IMAPve_d_MP5_DMS_SideView"
  Data Type Conversion210/1 -> Terminator201/1  "ob_IMAPva_g_obj_vel_y"
  Data Type Conversion74/1 -> Terminator65/1  "ob_IMAPve_d_EPS_Steer_Hold_State"
  Gain391/1 -> Data Type Conversion446/1, IMAPve_d_ORI_L0_MeasureType/1  "IMAPve_d_ORI_L0_MeasureType"
  Gain146/1 -> Data Type Conversion285/1, IMAPve_g_L0_C3_Back/1  "IMAPve_g_L0_C3_Back"
  Gain16/1 -> Data Type Conversion68/1, IMAPve_d_SAS_Trim_State/1
  SDFAve_g_ORI_L0_C3/1 -> Gain277/1
  Gain121/1 -> Data Type Conversion303/1, IMAPve_g_L1_C3_Back/1  "IMAPve_g_L1_C3_Back"
  Gain396/1 -> IMAPve_g_ORI_L0_ExistProb/1, Data Type Conversion443/1  "IMAPve_g_ORI_L0_ExistProb"
  Gain214/1 -> Data Type Conversion220/1, IMAPva_g_obj_length/1  "IMAPva_g_obj_length"
  Gain120/1 -> Data Type Conversion302/1, IMAPve_g_L1_C2_Back/1  "IMAPve_g_L1_C2_Back"
  Gain137/1 -> Data Type Conversion294/1, IMAPve_g_R0_C3_Back/1  "IMAPve_g_R0_C3_Back"
  Data Type Conversion61/1 -> Terminator52/1  "ob_IMAPve_d_Time_System_Clock"
  Gain104/1 -> Data Type Conversion313/1, IMAPve_g_R1_Range_Back/1  "IMAPve_g_R1_Range_Back"
  Gain122/1 -> Data Type Conversion304/1, IMAPve_g_L1_Range_Back/1  "IMAPve_g_L1_Range_Back"
  SDFAve_g_L1_C3_BACK_COEF/1 -> Gain121/1
  ? -> Gain11/1
  Gain203/1 -> Data Type Conversion227/1, IMAPva_d_obj_age/1  "IMAPva_d_obj_age"
  Data Type Conversion403/1 -> Terminator398/1  "ob_IMAPva_d_ORI_Obj_RelVelValid"
  Gain310/1 -> Data Type Conversion19/1, IMAPve_d_BSD_LCW_Switch/1
  Data Type Conversion87/1 -> Terminator78/1  "ob_IMAPve_g_EMS_Engine_Speed"
  Data Type Conversion136/1 -> Terminator127/1  "ob_IMAPve_d_ESC_Hold_State"
  Data Type Conversion55/1 -> Terminator46/1  "ob_IMAPve_d_BCM_CHMSL_Status"
  Data Type Conversion370/1 -> Terminator368/1  "ob_IMAPve_d_ESC_ABS_Valid"
  Gain111/1 -> Data Type Conversion309/1, IMAPve_g_R1_C0_Back/1  "IMAPve_g_R1_C0_Back"
  Gain114/1 -> Data Type Conversion312/1, IMAPve_g_R1_C3_Back/1  "IMAPve_g_R1_C3_Back"
  Gain113/1 -> Data Type Conversion311/1, IMAPve_g_R1_C2_Back/1  "IMAPve_g_R1_C2_Back"
  SDFAve_g_R1_BACK_RANGE/1 -> Gain104/1
  Data Type Conversion214/1 -> Terminator205/1  "ob_IMAPva_g_obj_pos_var_y"
  Gain313/1 -> Data Type Conversion22/1, IMAPve_d_DOW_Switch/1
  Data Type Conversion430/1 -> Terminator411/1  "ob_IMAPva_g_ORI_Obj_3DAngleStdDev"
  Data Type Conversion364/1 -> Terminator362/1  "ob_IMAPve_d_EMS_AccPedal_Fault"
  Gain153/1 -> Data Type Conversion274/1, IMAPve_g_R1_C3/1  "IMAPve_g_R1_C3"
  Data Type Conversion464/1 -> Terminator445/1  "ob_IMAPve_g_ORI_RoadedgeL0_DxStart"
  Data Type Conversion81/1 -> Terminator72/1  "ob_IMAPve_g_EMS_MinTWhl"
  Data Type Conversion436/1 -> Terminator417/1  "ob_IMAPva_g_ORI_Obj_Heading"
  Data Type Conversion203/1 -> Terminator194/1  "ob_IMAPve_d_Radar_Status"
  Gain112/1 -> Data Type Conversion310/1, IMAPve_g_R1_C1_Back/1  "IMAPve_g_R1_C1_Back"
  Gain284/1 -> Data Type Conversion84/1, IMAPve_g_EMS_Realize_TWhl/1
  ? -> Gain10/1
  SDFAva_g_obj_pos_var_y/1 -> Gain226/1
  Gain254/1 -> Data Type Conversion184/1, IMAPve_g_ORI_R1_C3/1  "IMAPve_g_ORI_R1_C3"
  Gain215/1 -> Data Type Conversion415/1, IMAPve_d_MP5_UPA_Switch/1
  ? -> Gain441/1
  SDFAve_g_R1_C1_BACK_COEF/1 -> Gain112/1
  ? -> Gain409/1
  Gain90/1 -> Data Type Conversion321/1, IMAPve_d_ESC_TCS_ErrorStatus/1
  SDFAva_g_obj_acc_x/1 -> Gain223/1
  ? -> Gain103/1
  SDFAve_g_CameraSignalFault/1 -> Gain101/1
  SDFAve_d_sen_sta_LF_radar/1 -> Gain229/1
  Data Type Conversion234/1 -> Terminator225/1  "ob_IMAPve_d_MP5_DMS_DrinkWater"
  Data Type Conversion309/1 -> Terminator300/1  "ob_IMAPve_g_R1_C0_Back"
  Data Type Conversion88/1 -> Terminator79/1  "ob_IMAPve_d_TCU_Actual_Gear"
  Gain101/1 -> Data Type Conversion202/1, IMAPve_g_Camera_Signal_Fault/1  "IMAPve_g_Camera_Signal_Fault"
  Data Type Conversion71/1 -> Terminator62/1  "ob_IMAPve_g_SW_Angle_Speed"
  ? -> Gain412/1
  SDFAva_d_ORI_Obj_ID/1 -> Gain12/1
  Data Type Conversion365/1 -> Terminator363/1  "ob_IMAPve_d_TCU_PRND_State"
  Data Type Conversion271/1 -> Terminator262/1  "ob_IMAPve_g_R1_C0"
  ? -> Gain355/1
  SDFAve_g_R1_C3_BACK_COEF/1 -> Gain114/1
  SDFAve_g_R1_C2_BACK_COEF/1 -> Gain113/1
  Gain435/1 -> IMAPve_d_ORI_FS_OutOfFocus0/1, Data Type Conversion390/1  "IMAPve_d_ORI_FS_OutOfFocus0"
  SDFAve_g_L1_C0_BACK_COEF/1 -> Gain119/1
  ? -> Gain364/1
  Data Type Conversion186/1 -> Terminator177/1  "ob_IMAPve_g_ORI_R1_C1"
  Gain296/1 -> Data Type Conversion221/1, IMAPve_d_MP5_DMS_Sensity/1  "IMAPve_d_MP5_DMS_Sensity"
  SDFAve_g_L0_C2_BACK_COEF/1 -> Gain145/1
  Gain87/1 -> Data Type Conversion136/1, IMAPve_d_ESC_Hold_State/1
  Gain200/1 -> Data Type Conversion240/1, IMAPve_g_L0_C2/1  "IMAPve_g_L0_C2"
  ? -> Gain429/1
  Gain77/1 -> Data Type Conversion91/1, IMAPve_d_EMS_ACC_Effective/1
  ? -> Gain258/1
  Data Type Conversion199/1 -> Terminator190/1  "ob_IMAPve_d_Fusion_Time_Stamp"
  Gain186/1 -> Data Type Conversion38/1, IMAPve_d_FCW_Sensitivity/1
  Gain333/1 -> Data Type Conversion364/1, IMAPve_d_EMS_AccPedal_Fault/1
  Gain82/1 -> Data Type Conversion93/1, IMAPve_d_EMS_ACC_Inhibited/1
  Gain27/1 -> Data Type Conversion48/1, IMAPve_d_SCC_Left_SwitchSig/1
  Data Type Conversion378/1 -> Terminator374/1  "ob_IMAPve_d_ESC_AEB_Available"
  ? -> Gain365/1
  Data Type Conversion386/1 -> Terminator382/1  "ob_IMAPve_d_ESC_EBD_AlarmSig"
  Data Type Conversion56/1 -> Terminator47/1  "ob_IMAPve_d_BCM_BrakeLamp_State"
  Data Type Conversion69/1 -> Terminator60/1  "ob_IMAPve_d_EPS_TrqLim_State"
  Gain159/1 -> Data Type Conversion262/1, IMAPve_g_L1_C2/1  "IMAPve_g_L1_C2"
  Gain226/1 -> Data Type Conversion214/1, IMAPva_g_obj_pos_var_y/1  "IMAPva_g_obj_pos_var_y"
  Gain81/1 -> Data Type Conversion92/1, IMAPve_d_EMS_ACC_CtlAvail/1
  Data Type Conversion102/1 -> Terminator93/1  "ob_IMAPve_g_ESC_UnYawRate"
  Data Type Conversion103/1 -> Terminator94/1  "ob_IMAPve_g_ESC_VehSpd"
  Data Type Conversion302/1 -> Terminator293/1  "ob_IMAPve_g_L1_C2_Back"
  Gain386/1 -> Data Type Conversion452/1, IMAPve_g_ORI_L0_TypeConf/1
  Gain265/1 -> Data Type Conversion165/1, IMAPve_g_ORI_L1_C2/1  "IMAPve_g_ORI_L1_C2"
  Gain70/1 -> Data Type Conversion99/1, IMAPve_d_TCU_Select_ATMode/1
  Data Type Conversion374/1 -> Terminator370/1  "ob_IMAPve_d_ESC_FL_WhlSpd_Fault"
  Gain64/1 -> Data Type Conversion128/1, IMAPve_d_ESC_FR_Wheel_Pulse/1
  Data Type Conversion470/1 -> Terminator451/1  "ob_IMAPve_d_ORI_RoadedgeL0_MeasureType"
  Gain198/1 -> Data Type Conversion238/1, IMAPve_g_L0_C0/1  "IMAPve_g_L0_C0"
  Gain68/1 -> Data Type Conversion97/1, IMAPve_d_TCU_DCT_Clutch_State/1
  SDFAve_g_R0_MARK_WIDTH/1 -> Gain172/1
